simulink model "Dyn_Nonlinear_four"  (R2021a)
settings: Solver=VariableStepAuto  StartTime=0.0  StopTime=10  FixedStep=0.048  MaxStep=0.048  RelTol=1e-5
(part 2 of 7)

== matlab function Dyn_Nonlinear_four/MATLAB Function1 ==
  data: a_teta input; tau output; t input; td input
function tau  = fcn(a_teta, t, td)
theta1 = t(1); theta2 = t(2); theta3 = t(3); 
theta4 = t(4); theta5 = t(5);  

thetad1 = td(1); thetad2 = td(2); thetad3 = td(3);
thetad4 = td(4); thetad5 = td(5); 

M=zeros(5);
M(1,1) = 0.1666*cos(theta4) - 0.4018*sin(theta4) + 0.028*cos(theta4)*cos(theta5) - 1.12*cos(theta1)*sin(theta1) + 0.095452*cos(theta2)*sin(theta2) + 0.367108*cos(theta3)*sin(theta3) - 0.103292*cos(theta4)*sin(theta4) - 0.14*cos(theta4)*sin(theta5) + 0.028*cos(theta5)*sin(theta5) - 3.54*cos(theta1)^2 + 0.30418*cos(theta2)^2 - 0.217828*cos(theta3)^2 - 0.030156*cos(theta4)^2 + 0.0672*cos(theta5)^2 + 0.87*cos(theta2)^2*cos(theta3) - 0.1666*cos(theta2)^2*cos(theta4) - 0.1666*cos(theta3)^2*cos(theta4) - 0.3136*cos(theta2)^2*sin(theta3) + 0.4018*cos(theta2)^2*sin(theta4) + 0.4018*cos(theta3)^2*sin(theta4) + 0.435656*cos(theta2)^2*cos(theta3)^2 + 0.060312*cos(theta2)^2*cos(theta4)^2 - 0.0672*cos(theta2)^2*cos(theta5)^2 + 0.060312*cos(theta3)^2*cos(theta4)^2 - 0.0672*cos(theta3)^2*cos(theta5)^2 - 0.0672*cos(theta4)^2*cos(theta5)^2 - 0.120624*cos(theta2)^2*cos(theta3)^2*cos(theta4)^2 + 0.1344*cos(theta2)^2*cos(theta3)^2*cos(theta5)^2 + 0.1344*cos(theta2)^2*cos(theta4)^2*cos(theta5)^2 + 0.1344*cos(theta3)^2*cos(theta4)^2*cos(theta5)^2 - 0.87*cos(theta2)*sin(theta2)*sin(theta3) + 0.1666*cos(theta2)*sin(theta2)*sin(theta4) + 0.098*cos(theta2)*sin(theta2)*sin(theta5) + 0.1666*cos(theta3)*sin(theta3)*sin(theta4) + 0.098*cos(theta3)*sin(theta3)*sin(theta5) + 0.098*cos(theta4)*sin(theta4)*sin(theta5) + 0.1666*cos(theta2)^2*cos(theta3)*cos(theta4) - 0.028*cos(theta2)^2*cos(theta4)*cos(theta5) - 0.028*cos(theta3)^2*cos(theta4)*cos(theta5) - 0.734216*cos(theta2)*cos(theta3)^2*sin(theta2) + 0.206584*cos(theta2)*cos(theta4)^2*sin(theta2) - 0.734216*cos(theta2)^2*cos(theta3)*sin(theta3) - 0.4018*cos(theta2)^2*cos(theta3)*sin(theta4) - 0.4018*cos(theta2)^2*cos(theta4)*sin(theta3) + 0.206584*cos(theta3)*cos(theta4)^2*sin(theta3) + 0.206584*cos(theta2)^2*cos(theta4)*sin(theta4) + 0.14*cos(theta2)^2*cos(theta4)*sin(theta5) + 0.206584*cos(theta3)^2*cos(theta4)*sin(theta4) - 0.028*cos(theta2)^2*cos(theta5)*sin(theta5) + 0.14*cos(theta3)^2*cos(theta4)*sin(theta5) - 0.028*cos(theta3)^2*cos(theta5)*sin(theta5) - 0.028*cos(theta4)^2*cos(theta5)*sin(theta5) - 0.1666*cos(theta2)^2*sin(theta3)*sin(theta4) + 0.3332*cos(theta2)^2*cos(theta3)^2*cos(theta4) - 0.8036*cos(theta2)^2*cos(theta3)^2*sin(theta4) - 0.3136*cos(theta2)*cos(theta3)*sin(theta2) + 0.4018*cos(theta2)*cos(theta4)*sin(theta2) - 0.0196*cos(theta2)*cos(theta5)*sin(theta2) + 0.4018*cos(theta3)*cos(theta4)*sin(theta3) - 0.0196*cos(theta3)*cos(theta5)*sin(theta3) - 0.0196*cos(theta4)*cos(theta5)*sin(theta4) + 0.028*cos(theta2)^2*cos(theta3)*cos(theta4)*cos(theta5) - 0.8036*cos(theta2)*cos(theta3)^2*cos(theta4)*sin(theta2) + 0.0392*cos(theta2)*cos(theta3)^2*cos(theta5)*sin(theta2) - 0.8036*cos(theta2)^2*cos(theta3)*cos(theta4)*sin(theta3) + 0.0392*cos(theta2)*cos(theta4)^2*cos(theta5)*sin(theta2) + 0.0392*cos(theta2)^2*cos(theta3)*cos(theta5)*sin(theta3) - 0.14*cos(theta2)^2*cos(theta3)*cos(theta4)*sin(theta5) + 0.0392*cos(theta3)*cos(theta4)^2*cos(theta5)*sin(theta3) + 0.0392*cos(theta2)^2*cos(theta4)*cos(theta5)*sin(theta4) + 0.0392*cos(theta3)^2*cos(theta4)*cos(theta5)*sin(theta4) - 0.2688*cos(theta2)^2*cos(theta3)^2*cos(theta4)^2*cos(theta5)^2 - 0.3332*cos(theta2)*cos(theta3)^2*sin(theta2)*sin(theta4) - 0.196*cos(theta2)*cos(theta3)^2*sin(theta2)*sin(theta5) - 0.3332*cos(theta2)^2*cos(theta3)*sin(theta3)*sin(theta4) - 0.196*cos(theta2)*cos(theta4)^2*sin(theta2)*sin(theta5) - 0.196*cos(theta2)^2*cos(theta3)*sin(theta3)*sin(theta5) - 0.028*cos(theta2)^2*cos(theta5)*sin(theta3)*sin(theta4) - 0.196*cos(theta3)*cos(theta4)^2*sin(theta3)*sin(theta5) - 0.196*cos(theta2)^2*cos(theta4)*sin(theta4)*sin(theta5) - 0.196*cos(theta3)^2*cos(theta4)*sin(theta4)*sin(theta5) + 0.14*cos(theta2)^2*sin(theta3)*sin(theta4)*sin(theta5) + 0.056*cos(theta2)^2*cos(theta3)^2*cos(theta4)*cos(theta5) - 0.413168*cos(theta2)*cos(theta3)^2*cos(theta4)^2*sin(theta2) - 0.413168*cos(theta2)^2*cos(theta3)*cos(theta4)^2*sin(theta3) - 0.413168*cos(theta2)^2*cos(theta3)^2*cos(theta4)*sin(theta4) - 0.28*cos(theta2)^2*cos(theta3)^2*cos(theta4)*sin(theta5) + 0.056*cos(theta2)^2*cos(theta3)^2*cos(theta5)*sin(theta5) + 0.056*cos(theta2)^2*cos(theta4)^2*cos(theta5)*sin(theta5) + 0.056*cos(theta3)^2*cos(theta4)^2*cos(theta5)*sin(theta5) - 0.4018*cos(theta2)*cos(theta3)*cos(theta4)*sin(theta2) - 0.435656*cos(theta2)*cos(theta3)*sin(theta2)*sin(theta3) - 0.1666*cos(theta2)*cos(theta3)*sin(theta2)*sin(theta4) - 0.1666*cos(theta2)*cos(theta4)*sin(theta2)*sin(theta3) - 0.060312*cos(theta2)*cos(theta4)*sin(theta2)*sin(theta4) + 0.028*cos(theta2)*cos(theta5)*sin(theta2)*sin(theta4) - 0.060312*cos(theta3)*cos(theta4)*sin(theta3)*sin(theta4) + 0.028*cos(theta3)*cos(theta5)*sin(theta3)*sin(theta4) + 0.4018*cos(theta2)*sin(theta2)*sin(theta3)*sin(theta4) - 0.14*cos(theta2)*sin(theta2)*sin(theta4)*sin(theta5) - 0.14*cos(theta3)*sin(theta3)*sin(theta4)*sin(theta5) + 0.120624*cos(theta2)*cos(theta3)*cos(theta4)^2*sin(theta2)*sin(theta3) - 0.1344*cos(theta2)*cos(theta3)*cos(theta5)^2*sin(theta2)*sin(theta3) + 0.120624*cos(theta2)*cos(theta3)^2*cos(theta4)*sin(theta2)*sin(theta4) - 0.056*cos(theta2)*cos(theta3)^2*cos(theta5)*sin(theta2)*sin(theta4) + 0.120624*cos(theta2)^2*cos(theta3)*cos(theta4)*sin(theta3)*sin(theta4) - 0.1344*cos(theta2)*cos(theta4)*cos(theta5)^2*sin(theta2)*sin(theta4) - 0.056*cos(theta2)^2*cos(theta3)*cos(theta5)*sin(theta3)*sin(theta4) - 0.1344*cos(theta3)*cos(theta4)*cos(theta5)^2*sin(theta3)*sin(theta4) + 0.28*cos(theta2)*cos(theta3)^2*sin(theta2)*sin(theta4)*sin(theta5) + 0.28*cos(theta2)^2*cos(theta3)*sin(theta3)*sin(theta4)*sin(theta5) - 0.0784*cos(theta2)*cos(theta3)^2*cos(theta4)^2*cos(theta5)*sin(theta2) - 0.0784*cos(theta2)^2*cos(theta3)*cos(theta4)^2*cos(theta5)*sin(theta3) - 0.0784*cos(theta2)^2*cos(theta3)^2*cos(theta4)*cos(theta5)*sin(theta4) + 0.392*cos(theta2)*cos(theta3)^2*cos(theta4)^2*sin(theta2)*sin(theta5) + 0.392*cos(theta2)^2*cos(theta3)*cos(theta4)^2*sin(theta3)*sin(theta5) + 0.392*cos(theta2)^2*cos(theta3)^2*cos(theta4)*sin(theta4)*sin(theta5) - 0.3332*cos(theta2)*cos(theta3)*cos(theta4)*sin(theta2)*sin(theta3) - 0.028*cos(theta2)*cos(theta3)*cos(theta5)*sin(theta2)*sin(theta4) - 0.028*cos(theta2)*cos(theta4)*cos(theta5)*sin(theta2)*sin(theta3) - 0.112*cos(theta2)^2*cos(theta3)^2*cos(theta4)^2*cos(theta5)*sin(theta5) + 0.8036*cos(theta2)*cos(theta3)*sin(theta2)*sin(theta3)*sin(theta4) + 0.14*cos(theta2)*cos(theta3)*sin(theta2)*sin(theta4)*sin(theta5) + 0.14*cos(theta2)*cos(theta4)*sin(theta2)*sin(theta3)*sin(theta5) + 0.2688*cos(theta2)*cos(theta3)*cos(theta4)^2*cos(theta5)^2*sin(theta2)*sin(theta3) + 0.2688*cos(theta2)*cos(theta3)^2*cos(theta4)*cos(theta5)^2*sin(theta2)*sin(theta4) + 0.2688*cos(theta2)^2*cos(theta3)*cos(theta4)*cos(theta5)^2*sin(theta3)*sin(theta4) - 0.056*cos(theta2)*cos(theta3)*cos(theta4)*cos(theta5)*sin(theta2)*sin(theta3) + 0.413168*cos(theta2)*cos(theta3)*cos(theta4)*sin(theta2)*sin(theta3)*sin(theta4) + 0.28*cos(theta2)*cos(theta3)*cos(theta4)*sin(theta2)*sin(theta3)*sin(theta5) - 0.056*cos(theta2)*cos(theta3)*cos(theta5)*sin(theta2)*sin(theta3)*sin(theta5) - 0.056*cos(theta2)*cos(theta4)*cos(theta5)*sin(theta2)*sin(theta4)*sin(theta5) - 0.056*cos(theta3)*cos(theta4)*cos(theta5)*sin(theta3)*sin(theta4)*sin(theta5) + 0.0784*cos(theta2)*cos(theta3)*cos(theta4)*cos(theta5)*sin(theta2)*sin(theta3)*sin(theta4) - 0.392*cos(theta2)*cos(theta3)*cos(theta4)*sin(theta2)*sin(theta3)*sin(theta4)*sin(theta5) + 0.112*cos(theta2)*cos(theta3)*cos(theta4)^2*cos(theta5)*sin(theta2)*sin(theta3)*sin(theta5) + 0.112*cos(theta2)*cos(theta3)^2*cos(theta4)*cos(theta5)*sin(theta2)*sin(theta4)*sin(theta5) + 0.112*cos(theta2)^2*cos(theta3)*cos(theta4)*cos(theta5)*sin(theta3)*sin(theta4)*sin(theta5) + 6.759168 ;
M(1,2) = 0.441816*sin(theta2) - 0.053508*cos(theta2) - 0.150528*cos(theta2)*cos(theta3) - 1.1*cos(theta1)*sin(theta1) + 0.4875*cos(theta2)*sin(theta3) + 0.4875*cos(theta3)*sin(theta2) + 0.07*cos(theta5)*sin(theta2) + 0.150528*sin(theta2)*sin(theta3) + 0.014*sin(theta2)*sin(theta5) - 3.54*cos(theta1)^2 - 0.373674*cos(theta2)*sin(theta3)*sin(theta4) - 0.373674*cos(theta3)*sin(theta2)*sin(theta4) - 0.373674*cos(theta4)*sin(theta2)*sin(theta3) + 0.014*cos(theta2)*sin(theta3)*sin(theta5) + 0.014*cos(theta3)*sin(theta2)*sin(theta5) - 0.190918*sin(theta2)*sin(theta3)*sin(theta4) + 0.373674*cos(theta2)*cos(theta3)*cos(theta4) + 0.190918*cos(theta2)*cos(theta3)*sin(theta4) + 0.190918*cos(theta2)*cos(theta4)*sin(theta3) + 0.190918*cos(theta3)*cos(theta4)*sin(theta2) + 0.07*cos(theta2)*cos(theta5)*sin(theta3) + 0.07*cos(theta3)*cos(theta5)*sin(theta2) + 0.028*cos(theta2)*cos(theta3)*cos(theta5)^2*sin(theta4) + 0.028*cos(theta2)*cos(theta4)*cos(theta5)^2*sin(theta3) + 0.028*cos(theta3)*cos(theta4)*cos(theta5)^2*sin(theta2) - 0.028*cos(theta5)^2*sin(theta2)*sin(theta3)*sin(theta4) + 0.049*cos(theta2)*cos(theta3)*cos(theta4)*cos(theta5) + 0.0098*cos(theta2)*cos(theta3)*cos(theta4)*sin(theta5) - 0.049*cos(theta2)*cos(theta5)*sin(theta3)*sin(theta4) - 0.049*cos(theta3)*cos(theta5)*sin(theta2)*sin(theta4) - 0.049*cos(theta4)*cos(theta5)*sin(theta2)*sin(theta3) - 0.0098*cos(theta2)*sin(theta3)*sin(theta4)*sin(theta5) - 0.0098*cos(theta3)*sin(theta2)*sin(theta4)*sin(theta5) - 0.0098*cos(theta4)*sin(theta2)*sin(theta3)*sin(theta5) - 0.0672*cos(theta2)*cos(theta3)*cos(theta5)*sin(theta4)*sin(theta5) - 0.0672*cos(theta2)*cos(theta4)*cos(theta5)*sin(theta3)*sin(theta5) - 0.0672*cos(theta3)*cos(theta4)*cos(theta5)*sin(theta2)*sin(theta5) + 0.0672*cos(theta5)*sin(theta2)*sin(theta3)*sin(theta4)*sin(theta5) + 4.14 ;
M(1,3) = 0.4875*cos(theta2)*sin(theta3) - 1.04*cos(theta1)*sin(theta1) - 0.150528*cos(theta2)*cos(theta3) + 0.4875*cos(theta3)*sin(theta2) + 0.150528*sin(theta2)*sin(theta3) - 3.43*cos(theta1)^2 - 0.373674*cos(theta2)*sin(theta3)*sin(theta4) - 0.373674*cos(theta3)*sin(theta2)*sin(theta4) - 0.373674*cos(theta4)*sin(theta2)*sin(theta3) + 0.014*cos(theta2)*sin(theta3)*sin(theta5) + 0.014*cos(theta3)*sin(theta2)*sin(theta5) - 0.190918*sin(theta2)*sin(theta3)*sin(theta4) + 0.373674*cos(theta2)*cos(theta3)*cos(theta4) + 0.190918*cos(theta2)*cos(theta3)*sin(theta4) + 0.190918*cos(theta2)*cos(theta4)*sin(theta3) + 0.190918*cos(theta3)*cos(theta4)*sin(theta2) + 0.07*cos(theta2)*cos(theta5)*sin(theta3) + 0.07*cos(theta3)*cos(theta5)*sin(theta2) + 0.028*cos(theta2)*cos(theta3)*cos(theta5)^2*sin(theta4) + 0.028*cos(theta2)*cos(theta4)*cos(theta5)^2*sin(theta3) + 0.028*cos(theta3)*cos(theta4)*cos(theta5)^2*sin(theta2) - 0.028*cos(theta5)^2*sin(theta2)*sin(theta3)*sin(theta4) + 0.049*cos(theta2)*cos(theta3)*cos(theta4)*cos(theta5) + 0.0098*cos(theta2)*cos(theta3)*cos(theta4)*sin(theta5) - 0.049*cos(theta2)*cos(theta5)*sin(theta3)*sin(theta4) - 0.049*cos(theta3)*cos(theta5)*sin(theta2)*sin(theta4) - 0.049*cos(theta4)*cos(theta5)*sin(theta2)*sin(theta3) - 0.0098*cos(theta2)*sin(theta3)*sin(theta4)*sin(theta5) - 0.0098*cos(theta3)*sin(theta2)*sin(theta4)*sin(theta5) - 0.0098*cos(theta4)*sin(theta2)*sin(theta3)*sin(theta5) - 0.0672*cos(theta2)*cos(theta3)*cos(theta5)*sin(theta4)*sin(theta5) - 0.0672*cos(theta2)*cos(theta4)*cos(theta5)*sin(theta3)*sin(theta5) - 0.0672*cos(theta3)*cos(theta4)*cos(theta5)*sin(theta2)*sin(theta5) + 0.0672*cos(theta5)*sin(theta2)*sin(theta3)*sin(theta4)*sin(theta5) + 3.98 ;
M(1,4) = 0.249082*sin(theta2)*sin(theta3)*sin(theta4) - 0.373674*cos(theta3)*sin(theta2)*sin(theta4) - 0.373674*cos(theta4)*sin(theta2)*sin(theta3) - 0.373674*cos(theta2)*sin(theta3)*sin(theta4) + 0.373674*cos(theta2)*cos(theta3)*cos(theta4) - 0.249082*cos(theta2)*cos(theta3)*sin(theta4) - 0.249082*cos(theta2)*cos(theta4)*sin(theta3) - 0.249082*cos(theta3)*cos(theta4)*sin(theta2) + 0.88*cos(theta1)^2*cos(theta2)*cos(theta3)*sin(theta4) + 0.88*cos(theta1)^2*cos(theta2)*cos(theta4)*sin(theta3) + 0.88*cos(theta1)^2*cos(theta3)*cos(theta4)*sin(theta2) + 0.028*cos(theta2)*cos(theta3)*cos(theta5)^2*sin(theta4) + 0.028*cos(theta2)*cos(theta4)*cos(theta5)^2*sin(theta3) + 0.028*cos(theta3)*cos(theta4)*cos(theta5)^2*sin(theta2) - 0.88*cos(theta1)^2*sin(theta2)*sin(theta3)*sin(theta4) - 0.028*cos(theta5)^2*sin(theta2)*sin(theta3)*sin(theta4) - 0.7*cos(theta1)*cos(theta2)*cos(theta3)*cos(theta4) + 0.049*cos(theta2)*cos(theta3)*cos(theta4)*cos(theta5) + 0.1*cos(theta2)*cos(theta3)*cos(theta4)*sin(theta1) + 0.0098*cos(theta2)*cos(theta3)*cos(theta4)*sin(theta5) + 0.7*cos(theta1)*cos(theta2)*sin(theta3)*sin(theta4) + 0.7*cos(theta1)*cos(theta3)*sin(theta2)*sin(theta4) + 0.7*cos(theta1)*cos(theta4)*sin(theta2)*sin(theta3) - 0.049*cos(theta2)*cos(theta5)*sin(theta3)*sin(theta4) - 0.049*cos(theta3)*cos(theta5)*sin(theta2)*sin(theta4) - 0.049*cos(theta4)*cos(theta5)*sin(theta2)*sin(theta3) - 0.1*cos(theta2)*sin(theta1)*sin(theta3)*sin(theta4) - 0.1*cos(theta3)*sin(theta1)*sin(theta2)*sin(theta4) - 0.1*cos(theta4)*sin(theta1)*sin(theta2)*sin(theta3) - 0.0098*cos(theta2)*sin(theta3)*sin(theta4)*sin(theta5) - 0.0098*cos(theta3)*sin(theta2)*sin(theta4)*sin(theta5) - 0.0098*cos(theta4)*sin(theta2)*sin(theta3)*sin(theta5) - 3.14*cos(theta1)*cos(theta2)*cos(theta3)*sin(theta1)*sin(theta4) - 3.14*cos(theta1)*cos(theta2)*cos(theta4)*sin(theta1)*sin(theta3) - 3.14*cos(theta1)*cos(theta3)*cos(theta4)*sin(theta1)*sin(theta2) - 0.0672*cos(theta2)*cos(theta3)*cos(theta5)*sin(theta4)*sin(theta5) - 0.0672*cos(theta2)*cos(theta4)*cos(theta5)*sin(theta3)*sin(theta5) - 0.0672*cos(theta3)*cos(theta4)*cos(theta5)*sin(theta2)*sin(theta5) + 3.14*cos(theta1)*sin(theta1)*sin(theta2)*sin(theta3)*sin(theta4) + 0.0672*cos(theta5)*sin(theta2)*sin(theta3)*sin(theta4)*sin(theta5) ;
M(1,5) = 0.014*cos(theta2)*cos(theta5) - 0.07*cos(theta2)*sin(theta5) - 0.0728*cos(theta2)*sin(theta3)*sin(theta4) - 0.0728*cos(theta3)*sin(theta2)*sin(theta4) - 0.0728*cos(theta4)*sin(theta2)*sin(theta3) - 0.014*cos(theta5)*sin(theta2)*sin(theta3) + 0.22*sin(theta2)*sin(theta3)*sin(theta4) + 0.07*sin(theta2)*sin(theta3)*sin(theta5) + 0.0728*cos(theta2)*cos(theta3)*cos(theta4) + 0.014*cos(theta2)*cos(theta3)*cos(theta5) - 0.22*cos(theta2)*cos(theta3)*sin(theta4) - 0.22*cos(theta2)*cos(theta4)*sin(theta3) - 0.22*cos(theta3)*cos(theta4)*sin(theta2) - 0.07*cos(theta2)*cos(theta3)*sin(theta5) + 0.44*cos(theta1)^2*cos(theta2)*cos(theta3)*sin(theta4) + 0.44*cos(theta1)^2*cos(theta2)*cos(theta4)*sin(theta3) + 0.44*cos(theta1)^2*cos(theta3)*cos(theta4)*sin(theta2) - 0.44*cos(theta1)^2*sin(theta2)*sin(theta3)*sin(theta4) - 0.35*cos(theta1)*cos(theta2)*cos(theta3)*cos(theta4) + 0.05*cos(theta2)*cos(theta3)*cos(theta4)*sin(theta1) - 0.0098*cos(theta2)*cos(theta3)*cos(theta5)*sin(theta4) - 0.0098*cos(theta2)*cos(theta4)*cos(theta5)*sin(theta3) - 0.0098*cos(theta3)*cos(theta4)*cos(theta5)*sin(theta2) + 0.35*cos(theta1)*cos(theta2)*sin(theta3)*sin(theta4) + 0.35*cos(theta1)*cos(theta3)*sin(theta2)*sin(theta4) + 0.35*cos(theta1)*cos(theta4)*sin(theta2)*sin(theta3) + 0.049*cos(theta2)*cos(theta3)*sin(theta4)*sin(theta5) + 0.049*cos(theta2)*cos(theta4)*sin(theta3)*sin(theta5) + 0.049*cos(theta3)*cos(theta4)*sin(theta2)*sin(theta5) - 0.05*cos(theta2)*sin(theta1)*sin(theta3)*sin(theta4) - 0.05*cos(theta3)*sin(theta1)*sin(theta2)*sin(theta4) - 0.05*cos(theta4)*sin(theta1)*sin(theta2)*sin(theta3) + 0.0098*cos(theta5)*sin(theta2)*sin(theta3)*sin(theta4) - 0.049*sin(theta2)*sin(theta3)*sin(theta4)*sin(theta5) - 1.57*cos(theta1)*cos(theta2)*cos(theta3)*sin(theta1)*sin(theta4) - 1.57*cos(theta1)*cos(theta2)*cos(theta4)*sin(theta1)*sin(theta3) - 1.57*cos(theta1)*cos(theta3)*cos(theta4)*sin(theta1)*sin(theta2) + 1.57*cos(theta1)*sin(theta1)*sin(theta2)*sin(theta3)*sin(theta4) ;
M(2,1) = 0.441816*sin(theta2) - 0.053508*cos(theta2) - 0.150528*cos(theta2)*cos(theta3) - 1.1*cos(theta1)*sin(theta1) + 0.4875*cos(theta2)*sin(theta3) + 0.4875*cos(theta3)*sin(theta2) + 0.07*cos(theta5)*sin(theta2) + 0.150528*sin(theta2)*sin(theta3) + 0.014*sin(theta2)*sin(theta5) - 3.54*cos(theta1)^2 - 0.373674*cos(theta2)*sin(theta3)*sin(theta4) - 0.373674*cos(theta3)*sin(theta2)*sin(theta4) - 0.373674*cos(theta4)*sin(theta2)*sin(theta3) + 0.014*cos(theta2)*sin(theta3)*sin(theta5) + 0.014*cos(theta3)*sin(theta2)*sin(theta5) - 0.190918*sin(theta2)*sin(theta3)*sin(theta4) + 0.373674*cos(theta2)*cos(theta3)*cos(theta4) + 0.190918*cos(theta2)*cos(theta3)*sin(theta4) + 0.190918*cos(theta2)*cos(theta4)*sin(theta3) + 0.190918*cos(theta3)*cos(theta4)*sin(theta2) + 0.07*cos(theta2)*cos(theta5)*sin(theta3) + 0.07*cos(theta3)*cos(theta5)*sin(theta2) + 0.028*cos(theta2)*cos(theta3)*cos(theta5)^2*sin(theta4) + 0.028*cos(theta2)*cos(theta4)*cos(theta5)^2*sin(theta3) + 0.028*cos(theta3)*cos(theta4)*cos(theta5)^2*sin(theta2) - 0.028*cos(theta5)^2*sin(theta2)*sin(theta3)*sin(theta4) + 0.049*cos(theta2)*cos(theta3)*cos(theta4)*cos(theta5) + 0.0098*cos(theta2)*cos(theta3)*cos(theta4)*sin(theta5) - 0.049*cos(theta2)*cos(theta5)*sin(theta3)*sin(theta4) - 0.049*cos(theta3)*cos(theta5)*sin(theta2)*sin(theta4) - 0.049*cos(theta4)*cos(theta5)*sin(theta2)*sin(theta3) - 0.0098*cos(theta2)*sin(theta3)*sin(theta4)*sin(theta5) - 0.0098*cos(theta3)*sin(theta2)*sin(theta4)*sin(theta5) - 0.0098*cos(theta4)*sin(theta2)*sin(theta3)*sin(theta5) - 0.0672*cos(theta2)*cos(theta3)*cos(theta5)*sin(theta4)*sin(theta5) - 0.0672*cos(theta2)*cos(theta4)*cos(theta5)*sin(theta3)*sin(theta5) - 0.0672*cos(theta3)*cos(theta4)*cos(theta5)*sin(theta2)*sin(theta5) + 0.0672*cos(theta5)*sin(theta2)*sin(theta3)*sin(theta4)*sin(theta5) + 4.14 ;
M(2,2) = 0.87*cos(theta3) + 0.1666*cos(theta4) - 0.3136*sin(theta3) - 0.4018*sin(theta4) + 0.1666*cos(theta3)*cos(theta4) + 0.028*cos(theta4)*cos(theta5) - 1.1*cos(theta1)*sin(theta1) - 0.4018*cos(theta3)*sin(theta4) - 0.4018*cos(theta4)*sin(theta3) - 0.14*cos(theta4)*sin(theta5) - 0.028*cos(theta5)*sin(theta5) - 0.1666*sin(theta3)*sin(theta4) - 3.54*cos(theta1)^2 - 0.0672*cos(theta5)^2 - 0.028*cos(theta5)*sin(theta3)*sin(theta4) + 0.14*sin(theta3)*sin(theta4)*sin(theta5) + 0.028*cos(theta3)*cos(theta4)*cos(theta5) - 0.14*cos(theta3)*cos(theta4)*sin(theta5) + 5.864008 ;
M(2,3) = 0.435*cos(theta3) + 0.1666*cos(theta4) - 0.1568*sin(theta3) - 0.4018*sin(theta4) + 0.0833*cos(theta3)*cos(theta4) + 0.028*cos(theta4)*cos(theta5) - 1.04*cos(theta1)*sin(theta1) - 0.2009*cos(theta3)*sin(theta4) - 0.2009*cos(theta4)*sin(theta3) - 0.14*cos(theta4)*sin(theta5) - 0.028*cos(theta5)*sin(theta5) - 0.0833*sin(theta3)*sin(theta4) - 3.43*cos(theta1)^2 - 0.0672*cos(theta5)^2 - 0.014*cos(theta5)*sin(theta3)*sin(theta4) + 0.07*sin(theta3)*sin(theta4)*sin(theta5) + 0.014*cos(theta3)*cos(theta4)*cos(theta5) - 0.07*cos(theta3)*cos(theta4)*sin(theta5) + 5.009128 ;
M(2,4) = 0.0833*cos(theta4) - 0.2009*sin(theta4) + 0.0833*cos(theta3)*cos(theta4) + 0.014*cos(theta4)*cos(theta5) - 0.2009*cos(theta3)*sin(theta4) - 0.2009*cos(theta4)*sin(theta3) - 0.07*cos(theta4)*sin(theta5) - 0.028*cos(theta5)*sin(theta5) - 0.0833*sin(theta3)*sin(theta4) - 0.0672*cos(theta5)^2 - 0.014*cos(theta5)*sin(theta3)*sin(theta4) + 0.44*sin(theta2)*sin(theta3)*sin(theta4) + 0.07*sin(theta3)*sin(theta4)*sin(theta5) + 0.014*cos(theta3)*cos(theta4)*cos(theta5) - 0.44*cos(theta2)*cos(theta3)*sin(theta4) - 0.44*cos(theta2)*cos(theta4)*sin(theta3) - 0.44*cos(theta3)*cos(theta4)*sin(theta2) - 0.07*cos(theta3)*cos(theta4)*sin(theta5) + 0.88*cos(theta1)^2*cos(theta2)*cos(theta3)*sin(theta4) + 0.88*cos(theta1)^2*cos(theta2)*cos(theta4)*sin(theta3) + 0.88*cos(theta1)^2*cos(theta3)*cos(theta4)*sin(theta2) - 0.88*cos(theta1)^2*sin(theta2)*sin(theta3)*sin(theta4) - 0.7*cos(theta1)*cos(theta2)*cos(theta3)*cos(theta4) + 0.1*cos(theta2)*cos(theta3)*cos(theta4)*sin(theta1) + 0.7*cos(theta1)*cos(theta2)*sin(theta3)*sin(theta4) + 0.7*cos(theta1)*cos(theta3)*sin(theta2)*sin(theta4) + 0.7*cos(theta1)*cos(theta4)*sin(theta2)*sin(theta3) - 0.1*cos(theta2)*sin(theta1)*sin(theta3)*sin(theta4) - 0.1*cos(theta3)*sin(theta1)*sin(theta2)*sin(theta4) - 0.1*cos(theta4)*sin(theta1)*sin(theta2)*sin(theta3) - 3.14*cos(theta1)*cos(theta2)*cos(theta3)*sin(theta1)*sin(theta4) - 3.14*cos(theta1)*cos(theta2)*cos(theta4)*sin(theta1)*sin(theta3) - 3.14*cos(theta1)*cos(theta3)*cos(theta4)*sin(theta1)*sin(theta2) + 3.14*cos(theta1)*sin(theta1)*sin(theta2)*sin(theta3)*sin(theta4) + 0.2268 ;
M(2,5) = 0.049*cos(theta5) + 0.0098*sin(theta5) - 0.07*cos(theta5)*sin(theta4) - 0.014*sin(theta4)*sin(theta5) - 0.014*cos(theta3)*sin(theta4)*sin(theta5) - 0.014*cos(theta4)*sin(theta3)*sin(theta5) + 0.22*sin(theta2)*sin(theta3)*sin(theta4) - 0.22*cos(theta2)*cos(theta3)*sin(theta4) - 0.22*cos(theta2)*cos(theta4)*sin(theta3) - 0.22*cos(theta3)*cos(theta4)*sin(theta2) - 0.07*cos(theta3)*cos(theta5)*sin(theta4) - 0.07*cos(theta4)*cos(theta5)*sin(theta3) + 0.44*cos(theta1)^2*cos(theta2)*cos(theta3)*sin(theta4) + 0.44*cos(theta1)^2*cos(theta2)*cos(theta4)*sin(theta3) + 0.44*cos(theta1)^2*cos(theta3)*cos(theta4)*sin(theta2) - 0.44*cos(theta1)^2*sin(theta2)*sin(theta3)*sin(theta4) - 0.35*cos(theta1)*cos(theta2)*cos(theta3)*cos(theta4) + 0.05*cos(theta2)*cos(theta3)*cos(theta4)*sin(theta1) + 0.35*cos(theta1)*cos(theta2)*sin(theta3)*sin(theta4) + 0.35*cos(theta1)*cos(theta3)*sin(theta2)*sin(theta4) + 0.35*cos(theta1)*cos(theta4)*sin(theta2)*sin(theta3) - 0.05*cos(theta2)*sin(theta1)*sin(theta3)*sin(theta4) - 0.05*cos(theta3)*sin(theta1)*sin(theta2)*sin(theta4) - 0.05*cos(theta4)*sin(theta1)*sin(theta2)*sin(theta3) - 1.57*cos(theta1)*cos(theta2)*cos(theta3)*sin(theta1)*sin(theta4) - 1.57*cos(theta1)*cos(theta2)*cos(theta4)*sin(theta1)*sin(theta3) - 1.57*cos(theta1)*cos(theta3)*cos(theta4)*sin(theta1)*sin(theta2) + 1.57*cos(theta1)*sin(theta1)*sin(theta2)*sin(theta3)*sin(theta4) ;
M(3,1) = 0.4875*cos(theta2)*sin(theta3) - 1.04*cos(theta1)*sin(theta1) - 0.150528*cos(theta2)*cos(theta3) + 0.4875*cos(theta3)*sin(theta2) + 0.150528*sin(theta2)*sin(theta3) - 3.43*cos(theta1)^2 - 0.373674*cos(theta2)*sin(theta3)*sin(theta4) - 0.373674*cos(theta3)*sin(theta2)*sin(theta4) - 0.373674*cos(theta4)*sin(theta2)*sin(theta3) + 0.014*cos(theta2)*sin(theta3)*sin(theta5) + 0.014*cos(theta3)*sin(theta2)*sin(theta5) - 0.190918*sin(theta2)*sin(theta3)*sin(theta4) + 0.373674*cos(theta2)*cos(theta3)*cos(theta4) + 0.190918*cos(theta2)*cos(theta3)*sin(theta4) + 0.190918*cos(theta2)*cos(theta4)*sin(theta3) + 0.190918*cos(theta3)*cos(theta4)*sin(theta2) + 0.07*cos(theta2)*cos(theta5)*sin(theta3) + 0.07*cos(theta3)*cos(theta5)*sin(theta2) + 0.028*cos(theta2)*cos(theta3)*cos(theta5)^2*sin(theta4) + 0.028*cos(theta2)*cos(theta4)*cos(theta5)^2*sin(theta3) + 0.028*cos(theta3)*cos(theta4)*cos(theta5)^2*sin(theta2) - 0.028*cos(theta5)^2*sin(theta2)*sin(theta3)*sin(theta4) + 0.049*cos(theta2)*cos(theta3)*cos(theta4)*cos(theta5) + 0.0098*cos(theta2)*cos(theta3)*cos(theta4)*sin(theta5) - 0.049*cos(theta2)*cos(theta5)*sin(theta3)*sin(theta4) - 0.049*cos(theta3)*cos(theta5)*sin(theta2)*sin(theta4) - 0.049*cos(theta4)*cos(theta5)*sin(theta2)*sin(theta3) - 0.0098*cos(theta2)*sin(theta3)*sin(theta4)*sin(theta5) - 0.0098*cos(theta3)*sin(theta2)*sin(theta4)*sin(theta5) - 0.0098*cos(theta4)*sin(theta2)*sin(theta3)*sin(theta5) - 0.0672*cos(theta2)*cos(theta3)*cos(theta5)*sin(theta4)*sin(theta5) - 0.0672*cos(theta2)*cos(theta4)*cos(theta5)*sin(theta3)*sin(theta5) - 0.0672*cos(theta3)*cos(theta4)*cos(theta5)*sin(theta2)*sin(theta5) + 0.0672*cos(theta5)*sin(theta2)*sin(theta3)*sin(theta4)*sin(theta5) + 3.98 ;
M(3,2) = 0.435*cos(theta3) + 0.1666*cos(theta4) - 0.1568*sin(theta3) - 0.4018*sin(theta4) + 0.0833*cos(theta3)*cos(theta4) + 0.028*cos(theta4)*cos(theta5) - 1.04*cos(theta1)*sin(theta1) - 0.2009*cos(theta3)*sin(theta4) - 0.2009*cos(theta4)*sin(theta3) - 0.14*cos(theta4)*sin(theta5) - 0.028*cos(theta5)*sin(theta5) - 0.0833*sin(theta3)*sin(theta4) - 3.43*cos(theta1)^2 - 0.0672*cos(theta5)^2 - 0.014*cos(theta5)*sin(theta3)*sin(theta4) + 0.07*sin(theta3)*sin(theta4)*sin(theta5) + 0.014*cos(theta3)*cos(theta4)*cos(theta5) - 0.07*cos(theta3)*cos(theta4)*sin(theta5) + 5.009128 ;
M(3,3) = 0.1666*cos(theta4) - 0.4018*sin(theta4) + 0.028*cos(theta4)*cos(theta5) - 1.04*cos(theta1)*sin(theta1) - 0.14*cos(theta4)*sin(theta5) - 0.028*cos(theta5)*sin(theta5) - 3.43*cos(theta1)^2 - 0.0672*cos(theta5)^2 + 5.009128 ;
M(3,4) = 0.0833*cos(theta4) - 0.2009*sin(theta4) + 0.014*cos(theta4)*cos(theta5) - 0.07*cos(theta4)*sin(theta5) - 0.028*cos(theta5)*sin(theta5) - 0.0672*cos(theta5)^2 + 0.44*sin(theta2)*sin(theta3)*sin(theta4) - 0.44*cos(theta2)*cos(theta3)*sin(theta4) - 0.44*cos(theta2)*cos(theta4)*sin(theta3) - 0.44*cos(theta3)*cos(theta4)*sin(theta2) + 0.88*cos(theta1)^2*cos(theta2)*cos(theta3)*sin(theta4) + 0.88*cos(theta1)^2*cos(theta2)*cos(theta4)*sin(theta3) + 0.88*cos(theta1)^2*cos(theta3)*cos(theta4)*sin(theta2) - 0.88*cos(theta1)^2*sin(theta2)*sin(theta3)*sin(theta4) - 0.7*cos(theta1)*cos(theta2)*cos(theta3)*cos(theta4) + 0.1*cos(theta2)*cos(theta3)*cos(theta4)*sin(theta1) + 0.7*cos(theta1)*cos(theta2)*sin(theta3)*sin(theta4) + 0.7*cos(theta1)*cos(theta3)*sin(theta2)*sin(theta4) + 0.7*cos(theta1)*cos(theta4)*sin(theta2)*sin(theta3) - 0.1*cos(theta2)*sin(theta1)*sin(theta3)*sin(theta4) - 0.1*cos(theta3)*sin(theta1)*sin(theta2)*sin(theta4) - 0.1*cos(theta4)*sin(theta1)*sin(theta2)*sin(theta3) - 3.14*cos(theta1)*cos(theta2)*cos(theta3)*sin(theta1)*sin(theta4) - 3.14*cos(theta1)*cos(theta2)*cos(theta4)*sin(theta1)*sin(theta3) - 3.14*cos(theta1)*cos(theta3)*cos(theta4)*sin(theta1)*sin(theta2) + 3.14*cos(theta1)*sin(theta1)*sin(theta2)*sin(theta3)*sin(theta4) + 0.2268 ;
M(3,5) = 0.049*cos(theta5) + 0.0098*sin(theta5) - 0.07*cos(theta5)*sin(theta4) - 0.014*sin(theta4)*sin(theta5) + 0.22*sin(theta2)*sin(theta3)*sin(theta4) - 0.22*cos(theta2)*cos(theta3)*sin(theta4) - 0.22*cos(theta2)*cos(theta4)*sin(theta3) - 0.22*cos(theta3)*cos(theta4)*sin(theta2) + 0.44*cos(theta1)^2*cos(theta2)*cos(theta3)*sin(theta4) + 0.44*cos(theta1)^2*cos(theta2)*cos(theta4)*sin(theta3) + 0.44*cos(theta1)^2*cos(theta3)*cos(theta4)*sin(theta2) - 0.44*cos(theta1)^2*sin(theta2)*sin(theta3)*sin(theta4) - 0.35*cos(theta1)*cos(theta2)*cos(theta3)*cos(theta4) + 0.05*cos(theta2)*cos(theta3)*cos(theta4)*sin(theta1) + 0.35*cos(theta1)*cos(theta2)*sin(theta3)*sin(theta4) + 0.35*cos(theta1)*cos(theta3)*sin(theta2)*sin(theta4) + 0.35*cos(theta1)*cos(theta4)*sin(theta2)*sin(theta3) - 0.05*cos(theta2)*sin(theta1)*sin(theta3)*sin(theta4) - 0.05*cos(theta3)*sin(theta1)*sin(theta2)*sin(theta4) - 0.05*cos(theta4)*sin(theta1)*sin(theta2)*sin(theta3) - 1.57*cos(theta1)*cos(theta2)*cos(theta3)*sin(theta1)*sin(theta4) - 1.57*cos(theta1)*cos(theta2)*cos(theta4)*sin(theta1)*sin(theta3) - 1.57*cos(theta1)*cos(theta3)*cos(theta4)*sin(theta1)*sin(theta2) + 1.57*cos(theta1)*sin(theta1)*sin(theta2)*sin(theta3)*sin(theta4) ;
M(4,1) = 0.249082*sin(theta2)*sin(theta3)*sin(theta4) - 0.373674*cos(theta3)*sin(theta2)*sin(theta4) - 0.373674*cos(theta4)*sin(theta2)*sin(theta3) - 0.373674*cos(theta2)*sin(theta3)*sin(theta4) + 0.373674*cos(theta2)*cos(theta3)*cos(theta4) - 0.249082*cos(theta2)*cos(theta3)*sin(theta4) - 0.249082*cos(theta2)*cos(theta4)*sin(theta3) - 0.249082*cos(theta3)*cos(theta4)*sin(theta2) + 0.88*cos(theta1)^2*cos(theta2)*cos(theta3)*sin(theta4) + 0.88*cos(theta1)^2*cos(theta2)*cos(theta4)*sin(theta3) + 0.88*cos(theta1)^2*cos(theta3)*cos(theta4)*sin(theta2) + 0.028*cos(theta2)*cos(theta3)*cos(theta5)^2*sin(theta4) + 0.028*cos(theta2)*cos(theta4)*cos(theta5)^2*sin(theta3) + 0.028*cos(theta3)*cos(theta4)*cos(theta5)^2*sin(theta2) - 0.88*cos(theta1)^2*sin(theta2)*sin(theta3)*sin(theta4) - 0.028*cos(theta5)^2*sin(theta2)*sin(theta3)*sin(theta4) - 0.7*cos(theta1)*cos(theta2)*cos(theta3)*cos(theta4) + 0.049*cos(theta2)*cos(theta3)*cos(theta4)*cos(theta5) + 0.1*cos(theta2)*cos(theta3)*cos(theta4)*sin(theta1) + 0.0098*cos(theta2)*cos(theta3)*cos(theta4)*sin(theta5) + 0.7*cos(theta1)*cos(theta2)*sin(theta3)*sin(theta4) + 0.7*cos(theta1)*cos(theta3)*sin(theta2)*sin(theta4) + 0.7*cos(theta1)*cos(theta4)*sin(theta2)*sin(theta3) - 0.049*cos(theta2)*cos(theta5)*sin(theta3)*sin(theta4) - 0.049*cos(theta3)*cos(theta5)*sin(theta2)*sin(theta4) - 0.049*cos(theta4)*cos(theta5)*sin(theta2)*sin(theta3) - 0.1*cos(theta2)*sin(theta1)*sin(theta3)*sin(theta4) - 0.1*cos(theta3)*sin(theta1)*sin(theta2)*sin(theta4) - 0.1*cos(theta4)*sin(theta1)*sin(theta2)*sin(theta3) - 0.0098*cos(theta2)*sin(theta3)*sin(theta4)*sin(theta5) - 0.0098*cos(theta3)*sin(theta2)*sin(theta4)*sin(theta5) - 0.0098*cos(theta4)*sin(theta2)*sin(theta3)*sin(theta5) - 3.14*cos(theta1)*cos(theta2)*cos(theta3)*sin(theta1)*sin(theta4) - 3.14*cos(theta1)*cos(theta2)*cos(theta4)*sin(theta1)*sin(theta3) - 3.14*cos(theta1)*cos(theta3)*cos(theta4)*sin(theta1)*sin(theta2) - 0.0672*cos(theta2)*cos(theta3)*cos(theta5)*sin(theta4)*sin(theta5) - 0.0672*cos(theta2)*cos(theta4)*cos(theta5)*sin(theta3)*sin(theta5) - 0.0672*cos(theta3)*cos(theta4)*cos(theta5)*sin(theta2)*sin(theta5) + 3.14*cos(theta1)*sin(theta1)*sin(theta2)*sin(theta3)*sin(theta4) + 0.0672*cos(theta5)*sin(theta2)*sin(theta3)*sin(theta4)*sin(theta5) ;
M(4,2) = 0.0833*cos(theta4) - 0.2009*sin(theta4) + 0.0833*cos(theta3)*cos(theta4) + 0.014*cos(theta4)*cos(theta5) - 0.2009*cos(theta3)*sin(theta4) - 0.2009*cos(theta4)*sin(theta3) - 0.07*cos(theta4)*sin(theta5) - 0.028*cos(theta5)*sin(theta5) - 0.0833*sin(theta3)*sin(theta4) - 0.0672*cos(theta5)^2 - 0.014*cos(theta5)*sin(theta3)*sin(theta4) + 0.44*sin(theta2)*sin(theta3)*sin(theta4) + 0.07*sin(theta3)*sin(theta4)*sin(theta5) + 0.014*cos(theta3)*cos(theta4)*cos(theta5) - 0.44*cos(theta2)*cos(theta3)*sin(theta4) - 0.44*cos(theta2)*cos(theta4)*sin(theta3) - 0.44*cos(theta3)*cos(theta4)*sin(theta2) - 0.07*cos(theta3)*cos(theta4)*sin(theta5) + 0.88*cos(theta1)^2*cos(theta2)*cos(theta3)*sin(theta4) + 0.88*cos(theta1)^2*cos(theta2)*cos(theta4)*sin(theta3) + 0.88*cos(theta1)^2*cos(theta3)*cos(theta4)*sin(theta2) - 0.88*cos(theta1)^2*sin(theta2)*sin(theta3)*sin(theta4) - 0.7*cos(theta1)*cos(theta2)*cos(theta3)*cos(theta4) + 0.1*cos(theta2)*cos(theta3)*cos(theta4)*sin(theta1) + 0.7*cos(theta1)*cos(theta2)*sin(theta3)*sin(theta4) + 0.7*cos(theta1)*cos(theta3)*sin(theta2)*sin(theta4) + 0.7*cos(theta1)*cos(theta4)*sin(theta2)*sin(theta3) - 0.1*cos(theta2)*sin(theta1)*sin(theta3)*sin(theta4) - 0.1*cos(theta3)*sin(theta1)*sin(theta2)*sin(theta4) - 0.1*cos(theta4)*sin(theta1)*sin(theta2)*sin(theta3) - 3.14*cos(theta1)*cos(theta2)*cos(theta3)*sin(theta1)*sin(theta4) - 3.14*cos(theta1)*cos(theta2)*cos(theta4)*sin(theta1)*sin(theta3) - 3.14*cos(theta1)*cos(theta3)*cos(theta4)*sin(theta1)*sin(theta2) + 3.14*cos(theta1)*sin(theta1)*sin(theta2)*sin(theta3)*sin(theta4) + 0.2268 ;
M(4,3) = 0.0833*cos(theta4) - 0.2009*sin(theta4) + 0.014*cos(theta4)*cos(theta5) - 0.07*cos(theta4)*sin(theta5) - 0.028*cos(theta5)*sin(theta5) - 0.0672*cos(theta5)^2 + 0.44*sin(theta2)*sin(theta3)*sin(theta4) - 0.44*cos(theta2)*cos(theta3)*sin(theta4) - 0.44*cos(theta2)*cos(theta4)*sin(theta3) - 0.44*cos(theta3)*cos(theta4)*sin(theta2) + 0.88*cos(theta1)^2*cos(theta2)*cos(theta3)*sin(theta4) + 0.88*cos(theta1)^2*cos(theta2)*cos(theta4)*sin(theta3) + 0.88*cos(theta1)^2*cos(theta3)*cos(theta4)*sin(theta2) - 0.88*cos(theta1)^2*sin(theta2)*sin(theta3)*sin(theta4) - 0.7*cos(theta1)*cos(theta2)*cos(theta3)*cos(theta4) + 0.1*cos(theta2)*cos(theta3)*cos(theta4)*sin(theta1) + 0.7*cos(theta1)*cos(theta2)*sin(theta3)*sin(theta4) + 0.7*cos(theta1)*cos(theta3)*sin(theta2)*sin(theta4) + 0.7*cos(theta1)*cos(theta4)*sin(theta2)*sin(theta3) - 0.1*cos(theta2)*sin(theta1)*sin(theta3)*sin(theta4) - 0.1*cos(theta3)*sin(theta1)*sin(theta2)*sin(theta4) - 0.1*cos(theta4)*sin(theta1)*sin(theta2)*sin(theta3) - 3.14*cos(theta1)*cos(theta2)*cos(theta3)*sin(theta1)*sin(theta4) - 3.14*cos(theta1)*cos(theta2)*cos(theta4)*sin(theta1)*sin(theta3) - 3.14*cos(theta1)*cos(theta3)*cos(theta4)*sin(theta1)*sin(theta2) + 3.14*cos(theta1)*sin(theta1)*sin(theta2)*sin(theta3)*sin(theta4) + 0.2268 ;
M(4,4) = 0.88*cos(theta1)*sin(theta1) - 0.028*cos(theta5)*sin(theta5) + 3.14*cos(theta1)^2 + 2.82*cos(theta2)^2 + 2.82*cos(theta3)^2 + 2.82*cos(theta4)^2 - 0.0672*cos(theta5)^2 - 3.14*cos(theta1)^2*cos(theta2)^2 - 3.14*cos(theta1)^2*cos(theta3)^2 - 3.14*cos(theta1)^2*cos(theta4)^2 - 5.64*cos(theta2)^2*cos(theta3)^2 - 5.64*cos(theta2)^2*cos(theta4)^2 - 5.64*cos(theta3)^2*cos(theta4)^2 + 6.28*cos(theta1)^2*cos(theta2)^2*cos(theta3)^2 + 6.28*cos(theta1)^2*cos(theta2)^2*cos(theta4)^2 + 6.28*cos(theta1)^2*cos(theta3)^2*cos(theta4)^2 + 11.28*cos(theta2)^2*cos(theta3)^2*cos(theta4)^2 - 1.4*cos(theta2)*sin(theta1)*sin(theta2) - 1.4*cos(theta3)*sin(theta1)*sin(theta3) - 1.4*cos(theta4)*sin(theta1)*sin(theta4) - 0.88*cos(theta1)*cos(theta2)^2*sin(theta1) - 0.88*cos(theta1)*cos(theta3)^2*sin(theta1) - 0.88*cos(theta1)*cos(theta4)^2*sin(theta1) - 0.2*cos(theta1)*cos(theta2)*sin(theta2) - 0.2*cos(theta1)*cos(theta3)*sin(theta3) - 0.2*cos(theta1)*cos(theta4)*sin(theta4) + 0.4*cos(theta1)*cos(theta2)*cos(theta3)^2*sin(theta2) + 0.4*cos(theta1)*cos(theta2)*cos(theta4)^2*sin(theta2) + 0.4*cos(theta1)*cos(theta2)^2*cos(theta3)*sin(theta3) + 0.4*cos(theta1)*cos(theta3)*cos(theta4)^2*sin(theta3) + 0.4*cos(theta1)*cos(theta2)^2*cos(theta4)*sin(theta4) + 0.4*cos(theta1)*cos(theta3)^2*cos(theta4)*sin(theta4) - 12.56*cos(theta1)^2*cos(theta2)^2*cos(theta3)^2*cos(theta4)^2 + 2.8*cos(theta2)*cos(theta3)^2*sin(theta1)*sin(theta2) + 2.8*cos(theta2)*cos(theta4)^2*sin(theta1)*sin(theta2) + 2.8*cos(theta2)^2*cos(theta3)*sin(theta1)*sin(theta3) + 2.8*cos(theta3)*cos(theta4)^2*sin(theta1)*sin(theta3) + 2.8*cos(theta2)^2*cos(theta4)*sin(theta1)*sin(theta4) + 2.8*cos(theta3)^2*cos(theta4)*sin(theta1)*sin(theta4) + 1.76*cos(theta1)*cos(theta2)^2*cos(theta3)^2*sin(theta1) + 1.76*cos(theta1)*cos(theta2)^2*cos(theta4)^2*sin(theta1) + 1.76*cos(theta1)*cos(theta3)^2*cos(theta4)^2*sin(theta1) + 5.64*cos(theta2)*cos(theta3)*sin(theta2)*sin(theta3) + 5.64*cos(theta2)*cos(theta4)*sin(theta2)*sin(theta4) + 5.64*cos(theta3)*cos(theta4)*sin(theta3)*sin(theta4) - 6.28*cos(theta1)^2*cos(theta2)*cos(theta3)*sin(theta2)*sin(theta3) - 6.28*cos(theta1)^2*cos(theta2)*cos(theta4)*sin(theta2)*sin(theta4) - 11.28*cos(theta2)*cos(theta3)*cos(theta4)^2*sin(theta2)*sin(theta3) - 11.28*cos(theta2)*cos(theta3)^2*cos(theta4)*sin(theta2)*sin(theta4) - 6.28*cos(theta1)^2*cos(theta3)*cos(theta4)*sin(theta3)*sin(theta4) - 11.28*cos(theta2)^2*cos(theta3)*cos(theta4)*sin(theta3)*sin(theta4) - 0.8*cos(theta1)*cos(theta2)*cos(theta3)^2*cos(theta4)^2*sin(theta2) - 0.8*cos(theta1)*cos(theta2)^2*cos(theta3)*cos(theta4)^2*sin(theta3) - 0.8*cos(theta1)*cos(theta2)^2*cos(theta3)^2*cos(theta4)*sin(theta4) - 5.6*cos(theta2)*cos(theta3)^2*cos(theta4)^2*sin(theta1)*sin(theta2) - 5.6*cos(theta2)^2*cos(theta3)*cos(theta4)^2*sin(theta1)*sin(theta3) - 5.6*cos(theta2)^2*cos(theta3)^2*cos(theta4)*sin(theta1)*sin(theta4) - 3.52*cos(theta1)*cos(theta2)^2*cos(theta3)^2*cos(theta4)^2*sin(theta1) + 12.56*cos(theta1)^2*cos(theta2)*cos(theta3)*cos(theta4)^2*sin(theta2)*sin(theta3) + 12.56*cos(theta1)^2*cos(theta2)*cos(theta3)^2*cos(theta4)*sin(theta2)*sin(theta4) + 12.56*cos(theta1)^2*cos(theta2)^2*cos(theta3)*cos(theta4)*sin(theta3)*sin(theta4) - 1.76*cos(theta1)*cos(theta2)*cos(theta3)*sin(theta1)*sin(theta2)*sin(theta3) - 1.76*cos(theta1)*cos(theta2)*cos(theta4)*sin(theta1)*sin(theta2)*sin(theta4) - 1.76*cos(theta1)*cos(theta3)*cos(theta4)*sin(theta1)*sin(theta3)*sin(theta4) + 0.8*cos(theta1)*cos(theta2)*cos(theta3)*cos(theta4)*sin(theta2)*sin(theta3)*sin(theta4) + 5.6*cos(theta2)*cos(theta3)*cos(theta4)*sin(theta1)*sin(theta2)*sin(theta3)*sin(theta4) + 3.52*cos(theta1)*cos(theta2)*cos(theta3)*cos(theta4)^2*sin(theta1)*sin(theta2)*sin(theta3) + 3.52*cos(theta1)*cos(theta2)*cos(theta3)^2*cos(theta4)*sin(theta1)*sin(theta2)*sin(theta4) + 3.52*cos(theta1)*cos(theta2)^2*cos(theta3)*cos(theta4)*sin(theta1)*sin(theta3)*sin(theta4) + 0.6668 ;
M(4,5) = 0.049*cos(theta5) + 0.0098*sin(theta5) + 0.44*cos(theta1)*sin(theta1) + 1.57*cos(theta1)^2 + 1.41*cos(theta2)^2 + 1.41*cos(theta3)^2 + 1.41*cos(theta4)^2 - 1.57*cos(theta1)^2*cos(theta2)^2 - 1.57*cos(theta1)^2*cos(theta3)^2 - 1.57*cos(theta1)^2*cos(theta4)^2 - 2.82*cos(theta2)^2*cos(theta3)^2 - 2.82*cos(theta2)^2*cos(theta4)^2 - 2.82*cos(theta3)^2*cos(theta4)^2 + 3.14*cos(theta1)^2*cos(theta2)^2*cos(theta3)^2 + 3.14*cos(theta1)^2*cos(theta2)^2*cos(theta4)^2 + 3.14*cos(theta1)^2*cos(theta3)^2*cos(theta4)^2 + 5.64*cos(theta2)^2*cos(theta3)^2*cos(theta4)^2 - 0.7*cos(theta2)*sin(theta1)*sin(theta2) - 0.7*cos(theta3)*sin(theta1)*sin(theta3) - 0.7*cos(theta4)*sin(theta1)*sin(theta4) - 0.44*cos(theta1)*cos(theta2)^2*sin(theta1) - 0.44*cos(theta1)*cos(theta3)^2*sin(theta1) - 0.44*cos(theta1)*cos(theta4)^2*sin(theta1) - 0.1*cos(theta1)*cos(theta2)*sin(theta2) - 0.1*cos(theta1)*cos(theta3)*sin(theta3) - 0.1*cos(theta1)*cos(theta4)*sin(theta4) + 0.2*cos(theta1)*cos(theta2)*cos(theta3)^2*sin(theta2) + 0.2*cos(theta1)*cos(theta2)*cos(theta4)^2*sin(theta2) + 0.2*cos(theta1)*cos(theta2)^2*cos(theta3)*sin(theta3) + 0.2*cos(theta1)*cos(theta3)*cos(theta4)^2*sin(theta3) + 0.2*cos(theta1)*cos(theta2)^2*cos(theta4)*sin(theta4) + 0.2*cos(theta1)*cos(theta3)^2*cos(theta4)*sin(theta4) - 6.28*cos(theta1)^2*cos(theta2)^2*cos(theta3)^2*cos(theta4)^2 + 1.4*cos(theta2)*cos(theta3)^2*sin(theta1)*sin(theta2) + 1.4*cos(theta2)*cos(theta4)^2*sin(theta1)*sin(theta2) + 1.4*cos(theta2)^2*cos(theta3)*sin(theta1)*sin(theta3) + 1.4*cos(theta3)*cos(theta4)^2*sin(theta1)*sin(theta3) + 1.4*cos(theta2)^2*cos(theta4)*sin(theta1)*sin(theta4) + 1.4*cos(theta3)^2*cos(theta4)*sin(theta1)*sin(theta4) + 0.88*cos(theta1)*cos(theta2)^2*cos(theta3)^2*sin(theta1) + 0.88*cos(theta1)*cos(theta2)^2*cos(theta4)^2*sin(theta1) + 0.88*cos(theta1)*cos(theta3)^2*cos(theta4)^2*sin(theta1) + 2.82*cos(theta2)*cos(theta3)*sin(theta2)*sin(theta3) + 2.82*cos(theta2)*cos(theta4)*sin(theta2)*sin(theta4) + 2.82*cos(theta3)*cos(theta4)*sin(theta3)*sin(theta4) - 3.14*cos(theta1)^2*cos(theta2)*cos(theta3)*sin(theta2)*sin(theta3) - 3.14*cos(theta1)^2*cos(theta2)*cos(theta4)*sin(theta2)*sin(theta4) - 5.64*cos(theta2)*cos(theta3)*cos(theta4)^2*sin(theta2)*sin(theta3) - 5.64*cos(theta2)*cos(theta3)^2*cos(theta4)*sin(theta2)*sin(theta4) - 3.14*cos(theta1)^2*cos(theta3)*cos(theta4)*sin(theta3)*sin(theta4) - 5.64*cos(theta2)^2*cos(theta3)*cos(theta4)*sin(theta3)*sin(theta4) - 0.4*cos(theta1)*cos(theta2)*cos(theta3)^2*cos(theta4)^2*sin(theta2) - 0.4*cos(theta1)*cos(theta2)^2*cos(theta3)*cos(theta4)^2*sin(theta3) - 0.4*cos(theta1)*cos(theta2)^2*cos(theta3)^2*cos(theta4)*sin(theta4) - 2.8*cos(theta2)*cos(theta3)^2*cos(theta4)^2*sin(theta1)*sin(theta2) - 2.8*cos(theta2)^2*cos(theta3)*cos(theta4)^2*sin(theta1)*sin(theta3) - 2.8*cos(theta2)^2*cos(theta3)^2*cos(theta4)*sin(theta1)*sin(theta4) - 1.76*cos(theta1)*cos(theta2)^2*cos(theta3)^2*cos(theta4)^2*sin(theta1) + 6.28*cos(theta1)^2*cos(theta2)*cos(theta3)*cos(theta4)^2*sin(theta2)*sin(theta3) + 6.28*cos(theta1)^2*cos(theta2)*cos(theta3)^2*cos(theta4)*sin(theta2)*sin(theta4) + 6.28*cos(theta1)^2*cos(theta2)^2*cos(theta3)*cos(theta4)*sin(theta3)*sin(theta4) - 0.88*cos(theta1)*cos(theta2)*cos(theta3)*sin(theta1)*sin(theta2)*sin(theta3) - 0.88*cos(theta1)*cos(theta2)*cos(theta4)*sin(theta1)*sin(theta2)*sin(theta4) - 0.88*cos(theta1)*cos(theta3)*cos(theta4)*sin(theta1)*sin(theta3)*sin(theta4) + 0.4*cos(theta1)*cos(theta2)*cos(theta3)*cos(theta4)*sin(theta2)*sin(theta3)*sin(theta4) + 2.8*cos(theta2)*cos(theta3)*cos(theta4)*sin(theta1)*sin(theta2)*sin(theta3)*sin(theta4) + 1.76*cos(theta1)*cos(theta2)*cos(theta3)*cos(theta4)^2*sin(theta1)*sin(theta2)*sin(theta3) + 1.76*cos(theta1)*cos(theta2)*cos(theta3)^2*cos(theta4)*sin(theta1)*sin(theta2)*sin(theta4) + 1.76*cos(theta1)*cos(theta2)^2*cos(theta3)*cos(theta4)*sin(theta1)*sin(theta3)*sin(theta4) + 0.22 ;
M(5,1) = 0.014*cos(theta2)*cos(theta5) - 0.07*cos(theta2)*sin(theta5) - 0.0728*cos(theta2)*sin(theta3)*sin(theta4) - 0.0728*cos(theta3)*sin(theta2)*sin(theta4) - 0.0728*cos(theta4)*sin(theta2)*sin(theta3) - 0.014*cos(theta5)*sin(theta2)*sin(theta3) + 0.22*sin(theta2)*sin(theta3)*sin(theta4) + 0.07*sin(theta2)*sin(theta3)*sin(theta5) + 0.0728*cos(theta2)*cos(theta3)*cos(theta4) + 0.014*cos(theta2)*cos(theta3)*cos(theta5) - 0.22*cos(theta2)*cos(theta3)*sin(theta4) - 0.22*cos(theta2)*cos(theta4)*sin(theta3) - 0.22*cos(theta3)*cos(theta4)*sin(theta2) - 0.07*cos(theta2)*cos(theta3)*sin(theta5) + 0.44*cos(theta1)^2*cos(theta2)*cos(theta3)*sin(theta4) + 0.44*cos(theta1)^2*cos(theta2)*cos(theta4)*sin(theta3) + 0.44*cos(theta1)^2*cos(theta3)*cos(theta4)*sin(theta2) - 0.44*cos(theta1)^2*sin(theta2)*sin(theta3)*sin(theta4) - 0.35*cos(theta1)*cos(theta2)*cos(theta3)*cos(theta4) + 0.05*cos(theta2)*cos(theta3)*cos(theta4)*sin(theta1) - 0.0098*cos(theta2)*cos(theta3)*cos(theta5)*sin(theta4) - 0.0098*cos(theta2)*cos(theta4)*cos(theta5)*sin(theta3) - 0.0098*cos(theta3)*cos(theta4)*cos(theta5)*sin(theta2) + 0.35*cos(theta1)*cos(theta2)*sin(theta3)*sin(theta4) + 0.35*cos(theta1)*cos(theta3)*sin(theta2)*sin(theta4) + 0.35*cos(theta1)*cos(theta4)*sin(theta2)*sin(theta3) + 0.049*cos(theta2)*cos(theta3)*sin(theta4)*sin(theta5) + 0.049*cos(theta2)*cos(theta4)*sin(theta3)*sin(theta5) + 0.049*cos(theta3)*cos(theta4)*sin(theta2)*sin(theta5) - 0.05*cos(theta2)*sin(theta1)*sin(theta3)*sin(theta4) - 0.05*cos(theta3)*sin(theta1)*sin(theta2)*sin(theta4) - 0.05*cos(theta4)*sin(theta1)*sin(theta2)*sin(theta3) + 0.0098*cos(theta5)*sin(theta2)*sin(theta3)*sin(theta4) - 0.049*sin(theta2)*sin(theta3)*sin(theta4)*sin(theta5) - 1.57*cos(theta1)*cos(theta2)*cos(theta3)*sin(theta1)*sin(theta4) - 1.57*cos(theta1)*cos(theta2)*cos(theta4)*sin(theta1)*sin(theta3) - 1.57*cos(theta1)*cos(theta3)*cos(theta4)*sin(theta1)*sin(theta2) + 1.57*cos(theta1)*sin(theta1)*sin(theta2)*sin(theta3)*sin(theta4) ;
M(5,2) = 0.049*cos(theta5) + 0.0098*sin(theta5) - 0.07*cos(theta5)*sin(theta4) - 0.014*sin(theta4)*sin(theta5) - 0.014*cos(theta3)*sin(theta4)*sin(theta5) - 0.014*cos(theta4)*sin(theta3)*sin(theta5) + 0.22*sin(theta2)*sin(theta3)*sin(theta4) - 0.22*cos(theta2)*cos(theta3)*sin(theta4) - 0.22*cos(theta2)*cos(theta4)*sin(theta3) - 0.22*cos(theta3)*cos(theta4)*sin(theta2) - 0.07*cos(theta3)*cos(theta5)*sin(theta4) - 0.07*cos(theta4)*cos(theta5)*sin(theta3) + 0.44*cos(theta1)^2*cos(theta2)*cos(theta3)*sin(theta4) + 0.44*cos(theta1)^2*cos(theta2)*cos(theta4)*sin(theta3) + 0.44*cos(theta1)^2*cos(theta3)*cos(theta4)*sin(theta2) - 0.44*cos(theta1)^2*sin(theta2)*sin(theta3)*sin(theta4) - 0.35*cos(theta1)*cos(theta2)*cos(theta3)*cos(theta4) + 0.05*cos(theta2)*cos(theta3)*cos(theta4)*sin(theta1) + 0.35*cos(theta1)*cos(theta2)*sin(theta3)*sin(theta4) + 0.35*cos(theta1)*cos(theta3)*sin(theta2)*sin(theta4) + 0.35*cos(theta1)*cos(theta4)*sin(theta2)*sin(theta3) - 0.05*cos(theta2)*sin(theta1)*sin(theta3)*sin(theta4) - 0.05*cos(theta3)*sin(theta1)*sin(theta2)*sin(theta4) - 0.05*cos(theta4)*sin(theta1)*sin(theta2)*sin(theta3) - 1.57*cos(theta1)*cos(theta2)*cos(theta3)*sin(theta1)*sin(theta4) - 1.57*cos(theta1)*cos(theta2)*cos(theta4)*sin(theta1)*sin(theta3) - 1.57*cos(theta1)*cos(theta3)*cos(theta4)*sin(theta1)*sin(theta2) + 1.57*cos(theta1)*sin(theta1)*sin(theta2)*sin(theta3)*sin(theta4) ;
M(5,3) = 0.049*cos(theta5) + 0.0098*sin(theta5) - 0.07*cos(theta5)*sin(theta4) - 0.014*sin(theta4)*sin(theta5) + 0.22*sin(theta2)*sin(theta3)*sin(theta4) - 0.22*cos(theta2)*cos(theta3)*sin(theta4) - 0.22*cos(theta2)*cos(theta4)*sin(theta3) - 0.22*cos(theta3)*cos(theta4)*sin(theta2) + 0.44*cos(theta1)^2*cos(theta2)*cos(theta3)*sin(theta4) + 0.44*cos(theta1)^2*cos(theta2)*cos(theta4)*sin(theta3) + 0.44*cos(theta1)^2*cos(theta3)*cos(theta4)*sin(theta2) - 0.44*cos(theta1)^2*sin(theta2)*sin(theta3)*sin(theta4) - 0.35*cos(theta1)*cos(theta2)*cos(theta3)*cos(theta4) + 0.05*cos(theta2)*cos(theta3)*cos(theta4)*sin(theta1) + 0.35*cos(theta1)*cos(theta2)*sin(theta3)*sin(theta4) + 0.35*cos(theta1)*cos(theta3)*sin(theta2)*sin(theta4) + 0.35*cos(theta1)*cos(theta4)*sin(theta2)*sin(theta3) - 0.05*cos(theta2)*sin(theta1)*sin(theta3)*sin(theta4) - 0.05*cos(theta3)*sin(theta1)*sin(theta2)*sin(theta4) - 0.05*cos(theta4)*sin(theta1)*sin(theta2)*sin(theta3) - 1.57*cos(theta1)*cos(theta2)*cos(theta3)*sin(theta1)*sin(theta4) - 1.57*cos(theta1)*cos(theta2)*cos(theta4)*sin(theta1)*sin(theta3) - 1.57*cos(theta1)*cos(theta3)*cos(theta4)*sin(theta1)*sin(theta2) + 1.57*cos(theta1)*sin(theta1)*sin(theta2)*sin(theta3)*sin(theta4) ;
M(5,4) = 0.049*cos(theta5) + 0.0098*sin(theta5) + 0.44*cos(theta1)*sin(theta1) + 1.57*cos(theta1)^2 + 1.41*cos(theta2)^2 + 1.41*cos(theta3)^2 + 1.41*cos(theta4)^2 - 1.57*cos(theta1)^2*cos(theta2)^2 - 1.57*cos(theta1)^2*cos(theta3)^2 - 1.57*cos(theta1)^2*cos(theta4)^2 - 2.82*cos(theta2)^2*cos(theta3)^2 - 2.82*cos(theta2)^2*cos(theta4)^2 - 2.82*cos(theta3)^2*cos(theta4)^2 + 3.14*cos(theta1)^2*cos(theta2)^2*cos(theta3)^2 + 3.14*cos(theta1)^2*cos(theta2)^2*cos(theta4)^2 + 3.14*cos(theta1)^2*cos(theta3)^2*cos(theta4)^2 + 5.64*cos(theta2)^2*cos(theta3)^2*cos(theta4)^2 - 0.7*cos(theta2)*sin(theta1)*sin(theta2) - 0.7*cos(theta3)*sin(theta1)*sin(theta3) - 0.7*cos(theta4)*sin(theta1)*sin(theta4) - 0.44*cos(theta1)*cos(theta2)^2*sin(theta1) - 0.44*cos(theta1)*cos(theta3)^2*sin(theta1) - 0.44*cos(theta1)*cos(theta4)^2*sin(theta1) - 0.1*cos(theta1)*cos(theta2)*sin(theta2) - 0.1*cos(theta1)*cos(theta3)*sin(theta3) - 0.1*cos(theta1)*cos(theta4)*sin(theta4) + 0.2*cos(theta1)*cos(theta2)*cos(theta3)^2*sin(theta2) + 0.2*cos(theta1)*cos(theta2)*cos(theta4)^2*sin(theta2) + 0.2*cos(theta1)*cos(theta2)^2*cos(theta3)*sin(theta3) + 0.2*cos(theta1)*cos(theta3)*cos(theta4)^2*sin(theta3) + 0.2*cos(theta1)*cos(theta2)^2*cos(theta4)*sin(theta4) + 0.2*cos(theta1)*cos(theta3)^2*cos(theta4)*sin(theta4) - 6.28*cos(theta1)^2*cos(theta2)^2*cos(theta3)^2*cos(theta4)^2 + 1.4*cos(theta2)*cos(theta3)^2*sin(theta1)*sin(theta2) + 1.4*cos(theta2)*cos(theta4)^2*sin(theta1)*sin(theta2) + 1.4*cos(theta2)^2*cos(theta3)*sin(theta1)*sin(theta3) + 1.4*cos(theta3)*cos(theta4)^2*sin(theta1)*sin(theta3) + 1.4*cos(theta2)^2*cos(theta4)*sin(theta1)*sin(theta4) + 1.4*cos(theta3)^2*cos(theta4)*sin(theta1)*sin(theta4) + 0.88*cos(theta1)*cos(theta2)^2*cos(theta3)^2*sin(theta1) + 0.88*cos(theta1)*cos(theta2)^2*cos(theta4)^2*sin(theta1) + 0.88*cos(theta1)*cos(theta3)^2*cos(theta4)^2*sin(theta1) + 2.82*cos(theta2)*cos(theta3)*sin(theta2)*sin(theta3) + 2.82*cos(theta2)*cos(theta4)*sin(theta2)*sin(theta4) + 2.82*cos(theta3)*cos(theta4)*sin(theta3)*sin(theta4) - 3.14*cos(theta1)^2*cos(theta2)*cos(theta3)*sin(theta2)*sin(theta3) - 3.14*cos(theta1)^2*cos(theta2)*cos(theta4)*sin(theta2)*sin(theta4) - 5.64*cos(theta2)*cos(theta3)*cos(theta4)^2*sin(theta2)*sin(theta3) - 5.64*cos(theta2)*cos(theta3)^2*cos(theta4)*sin(theta2)*sin(theta4) - 3.14*cos(theta1)^2*cos(theta3)*cos(theta4)*sin(theta3)*sin(theta4) - 5.64*cos(theta2)^2*cos(theta3)*cos(theta4)*sin(theta3)*sin(theta4) - 0.4*cos(theta1)*cos(theta2)*cos(theta3)^2*cos(theta4)^2*sin(theta2) - 0.4*cos(theta1)*cos(theta2)^2*cos(theta3)*cos(theta4)^2*sin(theta3) - 0.4*cos(theta1)*cos(theta2)^2*cos(theta3)^2*cos(theta4)*sin(theta4) - 2.8*cos(theta2)*cos(theta3)^2*cos(theta4)^2*sin(theta1)*sin(theta2) - 2.8*cos(theta2)^2*cos(theta3)*cos(theta4)^2*sin(theta1)*sin(theta3) - 2.8*cos(theta2)^2*cos(theta3)^2*cos(theta4)*sin(theta1)*sin(theta4) - 1.76*cos(theta1)*cos(theta2)^2*cos(theta3)^2*cos(theta4)^2*sin(theta1) + 6.28*cos(theta1)^2*cos(theta2)*cos(theta3)*cos(theta4)^2*sin(theta2)*sin(theta3) + 6.28*cos(theta1)^2*cos(theta2)*cos(theta3)^2*cos(theta4)*sin(theta2)*sin(theta4) + 6.28*cos(theta1)^2*cos(theta2)^2*cos(theta3)*cos(theta4)*sin(theta3)*sin(theta4) - 0.88*cos(theta1)*cos(theta2)*cos(theta3)*sin(theta1)*sin(theta2)*sin(theta3) - 0.88*cos(theta1)*cos(theta2)*cos(theta4)*sin(theta1)*sin(theta2)*sin(theta4) - 0.88*cos(theta1)*cos(theta3)*cos(theta4)*sin(theta1)*sin(theta3)*sin(theta4) + 0.4*cos(theta1)*cos(theta2)*cos(theta3)*cos(theta4)*sin(theta2)*sin(theta3)*sin(theta4) + 2.8*cos(theta2)*cos(theta3)*cos(theta4)*sin(theta1)*sin(theta2)*sin(theta3)*sin(theta4) + 1.76*cos(theta1)*cos(theta2)*cos(theta3)*cos(theta4)^2*sin(theta1)*sin(theta2)*sin(theta3) + 1.76*cos(theta1)*cos(theta2)*cos(theta3)^2*cos(theta4)*sin(theta1)*sin(theta2)*sin(theta4) + 1.76*cos(theta1)*cos(theta2)^2*cos(theta3)*cos(theta4)*sin(theta1)*sin(theta3)*sin(theta4) + 0.22 ;
M(5,5) = 0.44*cos(theta1)*sin(theta1) + 1.57*cos(theta1)^2 + 1.41*cos(theta2)^2 + 1.41*cos(theta3)^2 + 1.41*cos(theta4)^2 - 1.57*cos(theta1)^2*cos(theta2)^2 - 1.57*cos(theta1)^2*cos(theta3)^2 - 1.57*cos(theta1)^2*cos(theta4)^2 - 2.82*cos(theta2)^2*cos(theta3)^2 - 2.82*cos(theta2)^2*cos(theta4)^2 - 2.82*cos(theta3)^2*cos(theta4)^2 + 3.14*cos(theta1)^2*cos(theta2)^2*cos(theta3)^2 + 3.14*cos(theta1)^2*cos(theta2)^2*cos(theta4)^2 + 3.14*cos(theta1)^2*cos(theta3)^2*cos(theta4)^2 + 5.64*cos(theta2)^2*cos(theta3)^2*cos(theta4)^2 - 0.7*cos(theta2)*sin(theta1)*sin(theta2) - 0.7*cos(theta3)*sin(theta1)*sin(theta3) - 0.7*cos(theta4)*sin(theta1)*sin(theta4) - 0.44*cos(theta1)*cos(theta2)^2*sin(theta1) - 0.44*cos(theta1)*cos(theta3)^2*sin(theta1) - 0.44*cos(theta1)*cos(theta4)^2*sin(theta1) - 0.1*cos(theta1)*cos(theta2)*sin(theta2) - 0.1*cos(theta1)*cos(theta3)*sin(theta3) - 0.1*cos(theta1)*cos(theta4)*sin(theta4) + 0.2*cos(theta1)*cos(theta2)*cos(theta3)^2*sin(theta2) + 0.2*cos(theta1)*cos(theta2)*cos(theta4)^2*sin(theta2) + 0.2*cos(theta1)*cos(theta2)^2*cos(theta3)*sin(theta3) + 0.2*cos(theta1)*cos(theta3)*cos(theta4)^2*sin(theta3) + 0.2*cos(theta1)*cos(theta2)^2*cos(theta4)*sin(theta4) + 0.2*cos(theta1)*cos(theta3)^2*cos(theta4)*sin(theta4) - 6.28*cos(theta1)^2*cos(theta2)^2*cos(theta3)^2*cos(theta4)^2 + 1.4*cos(theta2)*cos(theta3)^2*sin(theta1)*sin(theta2) + 1.4*cos(theta2)*cos(theta4)^2*sin(theta1)*sin(theta2) + 1.4*cos(theta2)^2*cos(theta3)*sin(theta1)*sin(theta3) + 1.4*cos(theta3)*cos(theta4)^2*sin(theta1)*sin(theta3) + 1.4*cos(theta2)^2*cos(theta4)*sin(theta1)*sin(theta4) + 1.4*cos(theta3)^2*cos(theta4)*sin(theta1)*sin(theta4) + 0.88*cos(theta1)*cos(theta2)^2*cos(theta3)^2*sin(theta1) + 0.88*cos(theta1)*cos(theta2)^2*cos(theta4)^2*sin(theta1) + 0.88*cos(theta1)*cos(theta3)^2*cos(theta4)^2*sin(theta1) + 2.82*cos(theta2)*cos(theta3)*sin(theta2)*sin(theta3) + 2.82*cos(theta2)*cos(theta4)*sin(theta2)*sin(theta4) + 2.82*cos(theta3)*cos(theta4)*sin(theta3)*sin(theta4) - 3.14*cos(theta1)^2*cos(theta2)*cos(theta3)*sin(theta2)*sin(theta3) - 3.14*cos(theta1)^2*cos(theta2)*cos(theta4)*sin(theta2)*sin(theta4) - 5.64*cos(theta2)*cos(theta3)*cos(theta4)^2*sin(theta2)*sin(theta3) - 5.64*cos(theta2)*cos(theta3)^2*cos(theta4)*sin(theta2)*sin(theta4) - 3.14*cos(theta1)^2*cos(theta3)*cos(theta4)*sin(theta3)*sin(theta4) - 5.64*cos(theta2)^2*cos(theta3)*cos(theta4)*sin(theta3)*sin(theta4) - 0.4*cos(theta1)*cos(theta2)*cos(theta3)^2*cos(theta4)^2*sin(theta2) - 0.4*cos(theta1)*cos(theta2)^2*cos(theta3)*cos(theta4)^2*sin(theta3) - 0.4*cos(theta1)*cos(theta2)^2*cos(theta3)^2*cos(theta4)*sin(theta4) - 2.8*cos(theta2)*cos(theta3)^2*cos(theta4)^2*sin(theta1)*sin(theta2) - 2.8*cos(theta2)^2*cos(theta3)*cos(theta4)^2*sin(theta1)*sin(theta3) - 2.8*cos(theta2)^2*cos(theta3)^2*cos(theta4)*sin(theta1)*sin(theta4) - 1.76*cos(theta1)*cos(theta2)^2*cos(theta3)^2*cos(theta4)^2*sin(theta1) + 6.28*cos(theta1)^2*cos(theta2)*cos(theta3)*cos(theta4)^2*sin(theta2)*sin(theta3) + 6.28*cos(theta1)^2*cos(theta2)*cos(theta3)^2*cos(theta4)*sin(theta2)*sin(theta4) + 6.28*cos(theta1)^2*cos(theta2)^2*cos(theta3)*cos(theta4)*sin(theta3)*sin(theta4) - 0.88*cos(theta1)*cos(theta2)*cos(theta3)*sin(theta1)*sin(theta2)*sin(theta3) - 0.88*cos(theta1)*cos(theta2)*cos(theta4)*sin(theta1)*sin(theta2)*sin(theta4) - 0.88*cos(theta1)*cos(theta3)*cos(theta4)*sin(theta1)*sin(theta3)*sin(theta4) + 0.4*cos(theta1)*cos(theta2)*cos(theta3)*cos(theta4)*sin(theta2)*sin(theta3)*sin(theta4) + 2.8*cos(theta2)*cos(theta3)*cos(theta4)*sin(theta1)*sin(theta2)*sin(theta3)*sin(theta4) + 1.76*cos(theta1)*cos(theta2)*cos(theta3)*cos(theta4)^2*sin(theta1)*sin(theta2)*sin(theta3) + 1.76*cos(theta1)*cos(theta2)*cos(theta3)^2*cos(theta4)*sin(theta1)*sin(theta2)*sin(theta4) + 1.76*cos(theta1)*cos(theta2)^2*cos(theta3)*cos(theta4)*sin(theta1)*sin(theta3)*sin(theta4) + 0.2928 ;



C=zeros(5);
C(1,1) = 2.24*thetad1*cos(theta1)^2 - 1.1*thetad2 - 1.04*thetad3 - 1.12*thetad1 + 2.2*thetad2*cos(theta1)^2 + 2.08*thetad3*cos(theta1)^2 - 7.08*thetad1*cos(theta1)*sin(theta1) - 7.08*thetad2*cos(theta1)*sin(theta1) - 6.86*thetad3*cos(theta1)*sin(theta1) - 3.14*thetad4*cos(theta2)*cos(theta3)*sin(theta4) - 3.14*thetad4*cos(theta2)*cos(theta4)*sin(theta3) - 3.14*thetad4*cos(theta3)*cos(theta4)*sin(theta2) - 1.57*thetad5*cos(theta2)*cos(theta3)*sin(theta4) - 1.57*thetad5*cos(theta2)*cos(theta4)*sin(theta3) - 1.57*thetad5*cos(theta3)*cos(theta4)*sin(theta2) + 3.14*thetad4*sin(theta2)*sin(theta3)*sin(theta4) + 1.57*thetad5*sin(theta2)*sin(theta3)*sin(theta4) - 0.1*thetad4*cos(theta1)*cos(theta2)*cos(theta3)*cos(theta4) - 0.05*thetad5*cos(theta1)*cos(theta2)*cos(theta3)*cos(theta4) - 0.7*thetad4*cos(theta2)*cos(theta3)*cos(theta4)*sin(theta1) - 0.35*thetad5*cos(theta2)*cos(theta3)*cos(theta4)*sin(theta1) + 0.1*thetad4*cos(theta1)*cos(theta2)*sin(theta3)*sin(theta4) + 0.1*thetad4*cos(theta1)*cos(theta3)*sin(theta2)*sin(theta4) + 0.1*thetad4*cos(theta1)*cos(theta4)*sin(theta2)*sin(theta3) + 0.05*thetad5*cos(theta1)*cos(theta2)*sin(theta3)*sin(theta4) + 0.05*thetad5*cos(theta1)*cos(theta3)*sin(theta2)*sin(theta4) + 0.05*thetad5*cos(theta1)*cos(theta4)*sin(theta2)*sin(theta3) + 0.7*thetad4*cos(theta2)*sin(theta1)*sin(theta3)*sin(theta4) + 0.7*thetad4*cos(theta3)*sin(theta1)*sin(theta2)*sin(theta4) + 0.7*thetad4*cos(theta4)*sin(theta1)*sin(theta2)*sin(theta3) + 0.35*thetad5*cos(theta2)*sin(theta1)*sin(theta3)*sin(theta4) + 0.35*thetad5*cos(theta3)*sin(theta1)*sin(theta2)*sin(theta4) + 0.35*thetad5*cos(theta4)*sin(theta1)*sin(theta2)*sin(theta3) + 6.28*thetad4*cos(theta1)^2*cos(theta2)*cos(theta3)*sin(theta4) + 6.28*thetad4*cos(theta1)^2*cos(theta2)*cos(theta4)*sin(theta3) + 6.28*thetad4*cos(theta1)^2*cos(theta3)*cos(theta4)*sin(theta2) + 3.14*thetad5*cos(theta1)^2*cos(theta2)*cos(theta3)*sin(theta4) + 3.14*thetad5*cos(theta1)^2*cos(theta2)*cos(theta4)*sin(theta3) + 3.14*thetad5*cos(theta1)^2*cos(theta3)*cos(theta4)*sin(theta2) - 6.28*thetad4*cos(theta1)^2*sin(theta2)*sin(theta3)*sin(theta4) - 3.14*thetad5*cos(theta1)^2*sin(theta2)*sin(theta3)*sin(theta4) + 1.76*thetad4*cos(theta1)*cos(theta2)*cos(theta3)*sin(theta1)*sin(theta4) + 1.76*thetad4*cos(theta1)*cos(theta2)*cos(theta4)*sin(theta1)*sin(theta3) + 1.76*thetad4*cos(theta1)*cos(theta3)*cos(theta4)*sin(theta1)*sin(theta2) + 0.88*thetad5*cos(theta1)*cos(theta2)*cos(theta3)*sin(theta1)*sin(theta4) + 0.88*thetad5*cos(theta1)*cos(theta2)*cos(theta4)*sin(theta1)*sin(theta3) + 0.88*thetad5*cos(theta1)*cos(theta3)*cos(theta4)*sin(theta1)*sin(theta2) - 1.76*thetad4*cos(theta1)*sin(theta1)*sin(theta2)*sin(theta3)*sin(theta4) - 0.88*thetad5*cos(theta1)*sin(theta1)*sin(theta2)*sin(theta3)*sin(theta4) ;
C(1,2) = 2.2*thetad1*cos(theta1)^2 - 1.1*thetad2 - 1.04*thetad3 - 1.1*thetad1 + 2.2*thetad2*cos(theta1)^2 + 2.08*thetad3*cos(theta1)^2 - 7.08*thetad1*cos(theta1)*sin(theta1) - 7.08*thetad2*cos(theta1)*sin(theta1) - 6.86*thetad3*cos(theta1)*sin(theta1) - 3.14*thetad4*cos(theta2)*cos(theta3)*sin(theta4) - 3.14*thetad4*cos(theta2)*cos(theta4)*sin(theta3) - 3.14*thetad4*cos(theta3)*cos(theta4)*sin(theta2) - 1.57*thetad5*cos(theta2)*cos(theta3)*sin(theta4) - 1.57*thetad5*cos(theta2)*cos(theta4)*sin(theta3) - 1.57*thetad5*cos(theta3)*cos(theta4)*sin(theta2) + 3.14*thetad4*sin(theta2)*sin(theta3)*sin(theta4) + 1.57*thetad5*sin(theta2)*sin(theta3)*sin(theta4) - 0.1*thetad4*cos(theta1)*cos(theta2)*cos(theta3)*cos(theta4) - 0.05*thetad5*cos(theta1)*cos(theta2)*cos(theta3)*cos(theta4) - 0.7*thetad4*cos(theta2)*cos(theta3)*cos(theta4)*sin(theta1) - 0.35*thetad5*cos(theta2)*cos(theta3)*cos(theta4)*sin(theta1) + 0.1*thetad4*cos(theta1)*cos(theta2)*sin(theta3)*sin(theta4) + 0.1*thetad4*cos(theta1)*cos(theta3)*sin(theta2)*sin(theta4) + 0.1*thetad4*cos(theta1)*cos(theta4)*sin(theta2)*sin(theta3) + 0.05*thetad5*cos(theta1)*cos(theta2)*sin(theta3)*sin(theta4) + 0.05*thetad5*cos(theta1)*cos(theta3)*sin(theta2)*sin(theta4) + 0.05*thetad5*cos(theta1)*cos(theta4)*sin(theta2)*sin(theta3) + 0.7*thetad4*cos(theta2)*sin(theta1)*sin(theta3)*sin(theta4) + 0.7*thetad4*cos(theta3)*sin(theta1)*sin(theta2)*sin(theta4) + 0.7*thetad4*cos(theta4)*sin(theta1)*sin(theta2)*sin(theta3) + 0.35*thetad5*cos(theta2)*sin(theta1)*sin(theta3)*sin(theta4) + 0.35*thetad5*cos(theta3)*sin(theta1)*sin(theta2)*sin(theta4) + 0.35*thetad5*cos(theta4)*sin(theta1)*sin(theta2)*sin(theta3) + 6.28*thetad4*cos(theta1)^2*cos(theta2)*cos(theta3)*sin(theta4) + 6.28*thetad4*cos(theta1)^2*cos(theta2)*cos(theta4)*sin(theta3) + 6.28*thetad4*cos(theta1)^2*cos(theta3)*cos(theta4)*sin(theta2) + 3.14*thetad5*cos(theta1)^2*cos(theta2)*cos(theta3)*sin(theta4) + 3.14*thetad5*cos(theta1)^2*cos(theta2)*cos(theta4)*sin(theta3) + 3.14*thetad5*cos(theta1)^2*cos(theta3)*cos(theta4)*sin(theta2) - 6.28*thetad4*cos(theta1)^2*sin(theta2)*sin(theta3)*sin(theta4) - 3.14*thetad5*cos(theta1)^2*sin(theta2)*sin(theta3)*sin(theta4) + 1.76*thetad4*cos(theta1)*cos(theta2)*cos(theta3)*sin(theta1)*sin(theta4) + 1.76*thetad4*cos(theta1)*cos(theta2)*cos(theta4)*sin(theta1)*sin(theta3) + 1.76*thetad4*cos(theta1)*cos(theta3)*cos(theta4)*sin(theta1)*sin(theta2) + 0.88*thetad5*cos(theta1)*cos(theta2)*cos(theta3)*sin(theta1)*sin(theta4) + 0.88*thetad5*cos(theta1)*cos(theta2)*cos(theta4)*sin(theta1)*sin(theta3) + 0.88*thetad5*cos(theta1)*cos(theta3)*cos(theta4)*sin(theta1)*sin(theta2) - 1.76*thetad4*cos(theta1)*sin(theta1)*sin(theta2)*sin(theta3)*sin(theta4) - 0.88*thetad5*cos(theta1)*sin(theta1)*sin(theta2)*sin(theta3)*sin(theta4) ;
C(1,3) = 2.08*thetad1*cos(theta1)^2 - 1.04*thetad2 - 1.04*thetad3 - 1.04*thetad1 + 2.08*thetad2*cos(theta1)^2 + 2.08*thetad3*cos(theta1)^2 - 6.86*thetad1*cos(theta1)*sin(theta1) - 6.86*thetad2*cos(theta1)*sin(theta1) - 6.86*thetad3*cos(theta1)*sin(theta1) - 3.14*thetad4*cos(theta2)*cos(theta3)*sin(theta4) - 3.14*thetad4*cos(theta2)*cos(theta4)*sin(theta3) - 3.14*thetad4*cos(theta3)*cos(theta4)*sin(theta2) - 1.57*thetad5*cos(theta2)*cos(theta3)*sin(theta4) - 1.57*thetad5*cos(theta2)*cos(theta4)*sin(theta3) - 1.57*thetad5*cos(theta3)*cos(theta4)*sin(theta2) + 3.14*thetad4*sin(theta2)*sin(theta3)*sin(theta4) + 1.57*thetad5*sin(theta2)*sin(theta3)*sin(theta4) - 0.1*thetad4*cos(theta1)*cos(theta2)*cos(theta3)*cos(theta4) - 0.05*thetad5*cos(theta1)*cos(theta2)*cos(theta3)*cos(theta4) - 0.7*thetad4*cos(theta2)*cos(theta3)*cos(theta4)*sin(theta1) - 0.35*thetad5*cos(theta2)*cos(theta3)*cos(theta4)*sin(theta1) + 0.1*thetad4*cos(theta1)*cos(theta2)*sin(theta3)*sin(theta4) + 0.1*thetad4*cos(theta1)*cos(theta3)*sin(theta2)*sin(theta4) + 0.1*thetad4*cos(theta1)*cos(theta4)*sin(theta2)*sin(theta3) + 0.05*thetad5*cos(theta1)*cos(theta2)*sin(theta3)*sin(theta4) + 0.05*thetad5*cos(theta1)*cos(theta3)*sin(theta2)*sin(theta4) + 0.05*thetad5*cos(theta1)*cos(theta4)*sin(theta2)*sin(theta3) + 0.7*thetad4*cos(theta2)*sin(theta1)*sin(theta3)*sin(theta4) + 0.7*thetad4*cos(theta3)*sin(theta1)*sin(theta2)*sin(theta4) + 0.7*thetad4*cos(theta4)*sin(theta1)*sin(theta2)*sin(theta3) + 0.35*thetad5*cos(theta2)*sin(theta1)*sin(theta3)*sin(theta4) + 0.35*thetad5*cos(theta3)*sin(theta1)*sin(theta2)*sin(theta4) + 0.35*thetad5*cos(theta4)*sin(theta1)*sin(theta2)*sin(theta3) + 6.28*thetad4*cos(theta1)^2*cos(theta2)*cos(theta3)*sin(theta4) + 6.28*thetad4*cos(theta1)^2*cos(theta2)*cos(theta4)*sin(theta3) + 6.28*thetad4*cos(theta1)^2*cos(theta3)*cos(theta4)*sin(theta2) + 3.14*thetad5*cos(theta1)^2*cos(theta2)*cos(theta3)*sin(theta4) + 3.14*thetad5*cos(theta1)^2*cos(theta2)*cos(theta4)*sin(theta3) + 3.14*thetad5*cos(theta1)^2*cos(theta3)*cos(theta4)*sin(theta2) - 6.28*thetad4*cos(theta1)^2*sin(theta2)*sin(theta3)*sin(theta4) - 3.14*thetad5*cos(theta1)^2*sin(theta2)*sin(theta3)*sin(theta4) + 1.76*thetad4*cos(theta1)*cos(theta2)*cos(theta3)*sin(theta1)*sin(theta4) + 1.76*thetad4*cos(theta1)*cos(theta2)*cos(theta4)*sin(theta1)*sin(theta3) + 1.76*thetad4*cos(theta1)*cos(theta3)*cos(theta4)*sin(theta1)*sin(theta2) + 0.88*thetad5*cos(theta1)*cos(theta2)*cos(theta3)*sin(theta1)*sin(theta4) + 0.88*thetad5*cos(theta1)*cos(theta2)*cos(theta4)*sin(theta1)*sin(theta3) + 0.88*thetad5*cos(theta1)*cos(theta3)*cos(theta4)*sin(theta1)*sin(theta2) - 1.76*thetad4*cos(theta1)*sin(theta1)*sin(theta2)*sin(theta3)*sin(theta4) - 0.88*thetad5*cos(theta1)*sin(theta1)*sin(theta2)*sin(theta3)*sin(theta4) ;
C(1,4) = 0.88*thetad4 + 0.44*thetad5 - 1.76*thetad4*cos(theta1)^2 - 0.88*thetad4*cos(theta2)^2 - 0.88*thetad5*cos(theta1)^2 - 0.88*thetad4*cos(theta3)^2 - 0.44*thetad5*cos(theta2)^2 - 0.88*thetad4*cos(theta4)^2 - 0.44*thetad5*cos(theta3)^2 - 0.44*thetad5*cos(theta4)^2 + 1.76*thetad4*cos(theta1)^2*cos(theta2)^2 + 1.76*thetad4*cos(theta1)^2*cos(theta3)^2 + 0.88*thetad5*cos(theta1)^2*cos(theta2)^2 + 1.76*thetad4*cos(theta1)^2*cos(theta4)^2 + 1.76*thetad4*cos(theta2)^2*cos(theta3)^2 + 0.88*thetad5*cos(theta1)^2*cos(theta3)^2 + 1.76*thetad4*cos(theta2)^2*cos(theta4)^2 + 0.88*thetad5*cos(theta1)^2*cos(theta4)^2 + 0.88*thetad5*cos(theta2)^2*cos(theta3)^2 + 1.76*thetad4*cos(theta3)^2*cos(theta4)^2 + 0.88*thetad5*cos(theta2)^2*cos(theta4)^2 + 0.88*thetad5*cos(theta3)^2*cos(theta4)^2 + 6.28*thetad4*cos(theta1)*sin(theta1) + 3.14*thetad5*cos(theta1)*sin(theta1) + 1.4*thetad4*cos(theta1)*cos(theta2)*sin(theta2) - 3.14*thetad1*cos(theta2)*cos(theta3)*sin(theta4) - 3.14*thetad1*cos(theta2)*cos(theta4)*sin(theta3) - 3.14*thetad1*cos(theta3)*cos(theta4)*sin(theta2) + 0.7*thetad5*cos(theta1)*cos(theta2)*sin(theta2) - 3.14*thetad2*cos(theta2)*cos(theta3)*sin(theta4) - 3.14*thetad2*cos(theta2)*cos(theta4)*sin(theta3) - 3.14*thetad2*cos(theta3)*cos(theta4)*sin(theta2) + 1.4*thetad4*cos(theta1)*cos(theta3)*sin(theta3) - 3.14*thetad3*cos(theta2)*cos(theta3)*sin(theta4) - 3.14*thetad3*cos(theta2)*cos(theta4)*sin(theta3) - 3.14*thetad3*cos(theta3)*cos(theta4)*sin(theta2) + 0.7*thetad5*cos(theta1)*cos(theta3)*sin(theta3) + 1.4*thetad4*cos(theta1)*cos(theta4)*sin(theta4) + 0.7*thetad5*cos(theta1)*cos(theta4)*sin(theta4) - 3.52*thetad4*cos(theta1)^2*cos(theta2)^2*cos(theta3)^2 - 3.52*thetad4*cos(theta1)^2*cos(theta2)^2*cos(theta4)^2 - 1.76*thetad5*cos(theta1)^2*cos(theta2)^2*cos(theta3)^2 - 3.52*thetad4*cos(theta1)^2*cos(theta3)^2*cos(theta4)^2 - 1.76*thetad5*cos(theta1)^2*cos(theta2)^2*cos(theta4)^2 - 3.52*thetad4*cos(theta2)^2*cos(theta3)^2*cos(theta4)^2 - 1.76*thetad5*cos(theta1)^2*cos(theta3)^2*cos(theta4)^2 - 1.76*thetad5*cos(theta2)^2*cos(theta3)^2*cos(theta4)^2 - 0.2*thetad4*cos(theta2)*sin(theta1)*sin(theta2) - 0.1*thetad5*cos(theta2)*sin(theta1)*sin(theta2) - 0.2*thetad4*cos(theta3)*sin(theta1)*sin(theta3) - 0.1*thetad5*cos(theta3)*sin(theta1)*sin(theta3) - 0.2*thetad4*cos(theta4)*sin(theta1)*sin(theta4) - 0.1*thetad5*cos(theta4)*sin(theta1)*sin(theta4) + 3.14*thetad1*sin(theta2)*sin(theta3)*sin(theta4) + 3.14*thetad2*sin(theta2)*sin(theta3)*sin(theta4) + 3.14*thetad3*sin(theta2)*sin(theta3)*sin(theta4) - 6.28*thetad4*cos(theta1)*cos(theta2)^2*sin(theta1) - 6.28*thetad4*cos(theta1)*cos(theta3)^2*sin(theta1) - 3.14*thetad5*cos(theta1)*cos(theta2)^2*sin(theta1) - 6.28*thetad4*cos(theta1)*cos(theta4)^2*sin(theta1) - 3.14*thetad5*cos(theta1)*cos(theta3)^2*sin(theta1) - 3.14*thetad5*cos(theta1)*cos(theta4)^2*sin(theta1) + 12.56*thetad4*cos(theta1)*cos(theta2)^2*cos(theta3)^2*sin(theta1) + 12.56*thetad4*cos(theta1)*cos(theta2)^2*cos(theta4)^2*sin(theta1) + 6.28*thetad5*cos(theta1)*cos(theta2)^2*cos(theta3)^2*sin(theta1) + 12.56*thetad4*cos(theta1)*cos(theta3)^2*cos(theta4)^2*sin(theta1) + 6.28*thetad5*cos(theta1)*cos(theta2)^2*cos(theta4)^2*sin(theta1) + 6.28*thetad5*cos(theta1)*cos(theta3)^2*cos(theta4)^2*sin(theta1) - 0.1*thetad1*cos(theta1)*cos(theta2)*cos(theta3)*cos(theta4) - 0.1*thetad2*cos(theta1)*cos(theta2)*cos(theta3)*cos(theta4) - 0.1*thetad3*cos(theta1)*cos(theta2)*cos(theta3)*cos(theta4) - 0.7*thetad1*cos(theta2)*cos(theta3)*cos(theta4)*sin(theta1) - 0.7*thetad2*cos(theta2)*cos(theta3)*cos(theta4)*sin(theta1) - 0.7*thetad3*cos(theta2)*cos(theta3)*cos(theta4)*sin(theta1) + 0.1*thetad1*cos(theta1)*cos(theta2)*sin(theta3)*sin(theta4) + 0.1*thetad1*cos(theta1)*cos(theta3)*sin(theta2)*sin(theta4) + 0.1*thetad1*cos(theta1)*cos(theta4)*sin(theta2)*sin(theta3) + 0.1*thetad2*cos(theta1)*cos(theta2)*sin(theta3)*sin(theta4) + 0.1*thetad2*cos(theta1)*cos(theta3)*sin(theta2)*sin(theta4) + 0.1*thetad2*cos(theta1)*cos(theta4)*sin(theta2)*sin(theta3) + 0.1*thetad3*cos(theta1)*cos(theta2)*sin(theta3)*sin(theta4) + 0.1*thetad3*cos(theta1)*cos(theta3)*sin(theta2)*sin(theta4) + 0.1*thetad3*cos(theta1)*cos(theta4)*sin(theta2)*sin(theta3) - 1.76*thetad4*cos(theta2)*cos(theta3)*sin(theta2)*sin(theta3) - 0.88*thetad5*cos(theta2)*cos(theta3)*sin(theta2)*sin(theta3) - 1.76*thetad4*cos(theta2)*cos(theta4)*sin(theta2)*sin(theta4) - 0.88*thetad5*cos(theta2)*cos(theta4)*sin(theta2)*sin(theta4) - 1.76*thetad4*cos(theta3)*cos(theta4)*sin(theta3)*sin(theta4) - 0.88*thetad5*cos(theta3)*cos(theta4)*sin(theta3)*sin(theta4) + 0.7*thetad1*cos(theta2)*sin(theta1)*sin(theta3)*sin(theta4) + 0.7*thetad1*cos(theta3)*sin(theta1)*sin(theta2)*sin(theta4) + 0.7*thetad1*cos(theta4)*sin(theta1)*sin(theta2)*sin(theta3) + 0.7*thetad2*cos(theta2)*sin(theta1)*sin(theta3)*sin(theta4) + 0.7*thetad2*cos(theta3)*sin(theta1)*sin(theta2)*sin(theta4) + 0.7*thetad2*cos(theta4)*sin(theta1)*sin(theta2)*sin(theta3) + 0.7*thetad3*cos(theta2)*sin(theta1)*sin(theta3)*sin(theta4) + 0.7*thetad3*cos(theta3)*sin(theta1)*sin(theta2)*sin(theta4) + 0.7*thetad3*cos(theta4)*sin(theta1)*sin(theta2)*sin(theta3) + 6.28*thetad1*cos(theta1)^2*cos(theta2)*cos(theta3)*sin(theta4) + 6.28*thetad1*cos(theta1)^2*cos(theta2)*cos(theta4)*sin(theta3) + 6.28*thetad1*cos(theta1)^2*cos(theta3)*cos(theta4)*sin(theta2) + 6.28*thetad2*cos(theta1)^2*cos(theta2)*cos(theta3)*sin(theta4) + 6.28*thetad2*cos(theta1)^2*cos(theta2)*cos(theta4)*sin(theta3) + 6.28*thetad2*cos(theta1)^2*cos(theta3)*cos(theta4)*sin(theta2) - 2.8*thetad4*cos(theta1)*cos(theta2)*cos(theta3)^2*sin(theta2) + 6.28*thetad3*cos(theta1)^2*cos(theta2)*cos(theta3)*sin(theta4) + 6.28*thetad3*cos(theta1)^2*cos(theta2)*cos(theta4)*sin(theta3) + 6.28*thetad3*cos(theta1)^2*cos(theta3)*cos(theta4)*sin(theta2) - 2.8*thetad4*cos(theta1)*cos(theta2)*cos(theta4)^2*sin(theta2) - 2.8*thetad4*cos(theta1)*cos(theta2)^2*cos(theta3)*sin(theta3) - 1.4*thetad5*cos(theta1)*cos(theta2)*cos(theta3)^2*sin(theta2) - 1.4*thetad5*cos(theta1)*cos(theta2)*cos(theta4)^2*sin(theta2) - 1.4*thetad5*cos(theta1)*cos(theta2)^2*cos(theta3)*sin(theta3) - 2.8*thetad4*cos(theta1)*cos(theta3)*cos(theta4)^2*sin(theta3) - 2.8*thetad4*cos(theta1)*cos(theta2)^2*cos(theta4)*sin(theta4) - 2.8*thetad4*cos(theta1)*cos(theta3)^2*cos(theta4)*sin(theta4) - 1.4*thetad5*cos(theta1)*cos(theta3)*cos(theta4)^2*sin(theta3) - 1.4*thetad5*cos(theta1)*cos(theta2)^2*cos(theta4)*sin(theta4) - 1.4*thetad5*cos(theta1)*cos(theta3)^2*cos(theta4)*sin(theta4) + 7.04*thetad4*cos(theta1)^2*cos(theta2)^2*cos(theta3)^2*cos(theta4)^2 + 3.52*thetad5*cos(theta1)^2*cos(theta2)^2*cos(theta3)^2*cos(theta4)^2 + 0.4*thetad4*cos(theta2)*cos(theta3)^2*sin(theta1)*sin(theta2) + 0.4*thetad4*cos(theta2)*cos(theta4)^2*sin(theta1)*sin(theta2) + 0.4*thetad4*cos(theta2)^2*cos(theta3)*sin(theta1)*sin(theta3) + 0.2*thetad5*cos(theta2)*cos(theta3)^2*sin(theta1)*sin(theta2) + 0.2*thetad5*cos(theta2)*cos(theta4)^2*sin(theta1)*sin(theta2) + 0.2*thetad5*cos(theta2)^2*cos(theta3)*sin(theta1)*sin(theta3) + 0.4*thetad4*cos(theta3)*cos(theta4)^2*sin(theta1)*sin(theta3) + 0.4*thetad4*cos(theta2)^2*cos(theta4)*sin(theta1)*sin(theta4) + 0.4*thetad4*cos(theta3)^2*cos(theta4)*sin(theta1)*sin(theta4) + 0.2*thetad5*cos(theta3)*cos(theta4)^2*sin(theta1)*sin(theta3) + 0.2*thetad5*cos(theta2)^2*cos(theta4)*sin(theta1)*sin(theta4) + 0.2*thetad5*cos(theta3)^2*cos(theta4)*sin(theta1)*sin(theta4) - 6.28*thetad1*cos(theta1)^2*sin(theta2)*sin(theta3)*sin(theta4) - 6.28*thetad2*cos(theta1)^2*sin(theta2)*sin(theta3)*sin(theta4) - 6.28*thetad3*cos(theta1)^2*sin(theta2)*sin(theta3)*sin(theta4) + 1.76*thetad1*cos(theta1)*cos(theta2)*cos(theta3)*sin(theta1)*sin(theta4) + 1.76*thetad1*cos(theta1)*cos(theta2)*cos(theta4)*sin(theta1)*sin(theta3) + 1.76*thetad1*cos(theta1)*cos(theta3)*cos(theta4)*sin(theta1)*sin(theta2) + 1.76*thetad2*cos(theta1)*cos(theta2)*cos(theta3)*sin(theta1)*sin(theta4) + 1.76*thetad2*cos(theta1)*cos(theta2)*cos(theta4)*sin(theta1)*sin(theta3) + 1.76*thetad2*cos(theta1)*cos(theta3)*cos(theta4)*sin(theta1)*sin(theta2) + 1.76*thetad3*cos(theta1)*cos(theta2)*cos(theta3)*sin(theta1)*sin(theta4) + 1.76*thetad3*cos(theta1)*cos(theta2)*cos(theta4)*sin(theta1)*sin(theta3) + 1.76*thetad3*cos(theta1)*cos(theta3)*cos(theta4)*sin(theta1)*sin(theta2) - 25.12*thetad4*cos(theta1)*cos(theta2)^2*cos(theta3)^2*cos(theta4)^2*sin(theta1) - 12.56*thetad5*cos(theta1)*cos(theta2)^2*cos(theta3)^2*cos(theta4)^2*sin(theta1) - 1.76*thetad1*cos(theta1)*sin(theta1)*sin(theta2)*sin(theta3)*sin(theta4) - 1.76*thetad2*cos(theta1)*sin(theta1)*sin(theta2)*sin(theta3)*sin(theta4) - 1.76*thetad3*cos(theta1)*sin(theta1)*sin(theta2)*sin(theta3)*sin(theta4) + 3.52*thetad4*cos(theta1)^2*cos(theta2)*cos(theta3)*sin(theta2)*sin(theta3) + 1.76*thetad5*cos(theta1)^2*cos(theta2)*cos(theta3)*sin(theta2)*sin(theta3) + 3.52*thetad4*cos(theta1)^2*cos(theta2)*cos(theta4)*sin(theta2)*sin(theta4) + 3.52*thetad4*cos(theta2)*cos(theta3)*cos(theta4)^2*sin(theta2)*sin(theta3) + 1.76*thetad5*cos(theta1)^2*cos(theta2)*cos(theta4)*sin(theta2)*sin(theta4) + 3.52*thetad4*cos(theta2)*cos(theta3)^2*cos(theta4)*sin(theta2)*sin(theta4) + 3.52*thetad4*cos(theta1)^2*cos(theta3)*cos(theta4)*sin(theta3)*sin(theta4) + 1.76*thetad5*cos(theta2)*cos(theta3)*cos(theta4)^2*sin(theta2)*sin(theta3) + 3.52*thetad4*cos(theta2)^2*cos(theta3)*cos(theta4)*sin(theta3)*sin(theta4) + 1.76*thetad5*cos(theta2)*cos(theta3)^2*cos(theta4)*sin(theta2)*sin(theta4) + 1.76*thetad5*cos(theta1)^2*cos(theta3)*cos(theta4)*sin(theta3)*sin(theta4) + 1.76*thetad5*cos(theta2)^2*cos(theta3)*cos(theta4)*sin(theta3)*sin(theta4) + 5.6*thetad4*cos(theta1)*cos(theta2)*cos(theta3)^2*cos(theta4)^2*sin(theta2) + 5.6*thetad4*cos(theta1)*cos(theta2)^2*cos(theta3)*cos(theta4)^2*sin(theta3) + 2.8*thetad5*cos(theta1)*cos(theta2)*cos(theta3)^2*cos(theta4)^2*sin(theta2) + 5.6*thetad4*cos(theta1)*cos(theta2)^2*cos(theta3)^2*cos(theta4)*sin(theta4) + 2.8*thetad5*cos(theta1)*cos(theta2)^2*cos(theta3)*cos(theta4)^2*sin(theta3) + 2.8*thetad5*cos(theta1)*cos(theta2)^2*cos(theta3)^2*cos(theta4)*sin(theta4) - 0.8*thetad4*cos(theta2)*cos(theta3)^2*cos(theta4)^2*sin(theta1)*sin(theta2) - 0.8*thetad4*cos(theta2)^2*cos(theta3)*cos(theta4)^2*sin(theta1)*sin(theta3) - 0.4*thetad5*cos(theta2)*cos(theta3)^2*cos(theta4)^2*sin(theta1)*sin(theta2) - 0.8*thetad4*cos(theta2)^2*cos(theta3)^2*cos(theta4)*sin(theta1)*sin(theta4) - 0.4*thetad5*cos(theta2)^2*cos(theta3)*cos(theta4)^2*sin(theta1)*sin(theta3) - 0.4*thetad5*cos(theta2)^2*cos(theta3)^2*cos(theta4)*sin(theta1)*sin(theta4) - 12.56*thetad4*cos(theta1)*cos(theta2)*cos(theta3)*sin(theta1)*sin(theta2)*sin(theta3) - 6.28*thetad5*cos(theta1)*cos(theta2)*cos(theta3)*sin(theta1)*sin(theta2)*sin(theta3) - 12.56*thetad4*cos(theta1)*cos(theta2)*cos(theta4)*sin(theta1)*sin(theta2)*sin(theta4) - 6.28*thetad5*cos(theta1)*cos(theta2)*cos(theta4)*sin(theta1)*sin(theta2)*sin(theta4) - 12.56*thetad4*cos(theta1)*cos(theta3)*cos(theta4)*sin(theta1)*sin(theta3)*sin(theta4) - 6.28*thetad5*cos(theta1)*cos(theta3)*cos(theta4)*sin(theta1)*sin(theta3)*sin(theta4) - 7.04*thetad4*cos(theta1)^2*cos(theta2)*cos(theta3)*cos(theta4)^2*sin(theta2)*sin(theta3) - 7.04*thetad4*cos(theta1)^2*cos(theta2)*cos(theta3)^2*cos(theta4)*sin(theta2)*sin(theta4) - 3.52*thetad5*cos(theta1)^2*cos(theta2)*cos(theta3)*cos(theta4)^2*sin(theta2)*sin(theta3) - 7.04*thetad4*cos(theta1)^2*cos(theta2)^2*cos(theta3)*cos(theta4)*sin(theta3)*sin(theta4) - 3.52*thetad5*cos(theta1)^2*cos(theta2)*cos(theta3)^2*cos(theta4)*sin(theta2)*sin(theta4) - 3.52*thetad5*cos(theta1)^2*cos(theta2)^2*cos(theta3)*cos(theta4)*sin(theta3)*sin(theta4) + 25.12*thetad4*cos(theta1)*cos(theta2)*cos(theta3)*cos(theta4)^2*sin(theta1)*sin(theta2)*sin(theta3) + 25.12*thetad4*cos(theta1)*cos(theta2)*cos(theta3)^2*cos(theta4)*sin(theta1)*sin(theta2)*sin(theta4) + 12.56*thetad5*cos(theta1)*cos(theta2)*cos(theta3)*cos(theta4)^2*sin(theta1)*sin(theta2)*sin(theta3) + 25.12*thetad4*cos(theta1)*cos(theta2)^2*cos(theta3)*cos(theta4)*sin(theta1)*sin(theta3)*sin(theta4) + 12.56*thetad5*cos(theta1)*cos(theta2)*cos(theta3)^2*cos(theta4)*sin(theta1)*sin(theta2)*sin(theta4) + 12.56*thetad5*cos(theta1)*cos(theta2)^2*cos(theta3)*cos(theta4)*sin(theta1)*sin(theta3)*sin(theta4) - 5.6*thetad4*cos(theta1)*cos(theta2)*cos(theta3)*cos(theta4)*sin(theta2)*sin(theta3)*sin(theta4) - 2.8*thetad5*cos(theta1)*cos(theta2)*cos(theta3)*cos(theta4)*sin(theta2)*sin(theta3)*sin(theta4) + 0.8*thetad4*cos(theta2)*cos(theta3)*cos(theta4)*sin(theta1)*sin(theta2)*sin(theta3)*sin(theta4) + 0.4*thetad5*cos(theta2)*cos(theta3)*cos(theta4)*sin(theta1)*sin(theta2)*sin(theta3)*sin(theta4) ;
C(1,5) = 0.44*thetad4 + 0.44*thetad5 - 0.88*thetad4*cos(theta1)^2 - 0.44*thetad4*cos(theta2)^2 - 0.88*thetad5*cos(theta1)^2 - 0.44*thetad4*cos(theta3)^2 - 0.44*thetad5*cos(theta2)^2 - 0.44*thetad4*cos(theta4)^2 - 0.44*thetad5*cos(theta3)^2 - 0.44*thetad5*cos(theta4)^2 + 0.88*thetad4*cos(theta1)^2*cos(theta2)^2 + 0.88*thetad4*cos(theta1)^2*cos(theta3)^2 + 0.88*thetad5*cos(theta1)^2*cos(theta2)^2 + 0.88*thetad4*cos(theta1)^2*cos(theta4)^2 + 0.88*thetad4*cos(theta2)^2*cos(theta3)^2 + 0.88*thetad5*cos(theta1)^2*cos(theta3)^2 + 0.88*thetad4*cos(theta2)^2*cos(theta4)^2 + 0.88*thetad5*cos(theta1)^2*cos(theta4)^2 + 0.88*thetad5*cos(theta2)^2*cos(theta3)^2 + 0.88*thetad4*cos(theta3)^2*cos(theta4)^2 + 0.88*thetad5*cos(theta2)^2*cos(theta4)^2 + 0.88*thetad5*cos(theta3)^2*cos(theta4)^2 + 3.14*thetad4*cos(theta1)*sin(theta1) + 3.14*thetad5*cos(theta1)*sin(theta1) + 0.7*thetad4*cos(theta1)*cos(theta2)*sin(theta2) - 1.57*thetad1*cos(theta2)*cos(theta3)*sin(theta4) - 1.57*thetad1*cos(theta2)*cos(theta4)*sin(theta3) - 1.57*thetad1*cos(theta3)*cos(theta4)*sin(theta2) + 0.7*thetad5*cos(theta1)*cos(theta2)*sin(theta2) - 1.57*thetad2*cos(theta2)*cos(theta3)*sin(theta4) - 1.57*thetad2*cos(theta2)*cos(theta4)*sin(theta3) - 1.57*thetad2*cos(theta3)*cos(theta4)*sin(theta2) + 0.7*thetad4*cos(theta1)*cos(theta3)*sin(theta3) - 1.57*thetad3*cos(theta2)*cos(theta3)*sin(theta4) - 1.57*thetad3*cos(theta2)*cos(theta4)*sin(theta3) - 1.57*thetad3*cos(theta3)*cos(theta4)*sin(theta2) + 0.7*thetad5*cos(theta1)*cos(theta3)*sin(theta3) + 0.7*thetad4*cos(theta1)*cos(theta4)*sin(theta4) + 0.7*thetad5*cos(theta1)*cos(theta4)*sin(theta4) - 1.76*thetad4*cos(theta1)^2*cos(theta2)^2*cos(theta3)^2 - 1.76*thetad4*cos(theta1)^2*cos(theta2)^2*cos(theta4)^2 - 1.76*thetad5*cos(theta1)^2*cos(theta2)^2*cos(theta3)^2 - 1.76*thetad4*cos(theta1)^2*cos(theta3)^2*cos(theta4)^2 - 1.76*thetad5*cos(theta1)^2*cos(theta2)^2*cos(theta4)^2 - 1.76*thetad4*cos(theta2)^2*cos(theta3)^2*cos(theta4)^2 - 1.76*thetad5*cos(theta1)^2*cos(theta3)^2*cos(theta4)^2 - 1.76*thetad5*cos(theta2)^2*cos(theta3)^2*cos(theta4)^2 - 0.1*thetad4*cos(theta2)*sin(theta1)*sin(theta2) - 0.1*thetad5*cos(theta2)*sin(theta1)*sin(theta2) - 0.1*thetad4*cos(theta3)*sin(theta1)*sin(theta3) - 0.1*thetad5*cos(theta3)*sin(theta1)*sin(theta3) - 0.1*thetad4*cos(theta4)*sin(theta1)*sin(theta4) - 0.1*thetad5*cos(theta4)*sin(theta1)*sin(theta4) + 1.57*thetad1*sin(theta2)*sin(theta3)*sin(theta4) + 1.57*thetad2*sin(theta2)*sin(theta3)*sin(theta4) + 1.57*thetad3*sin(theta2)*sin(theta3)*sin(theta4) - 3.14*thetad4*cos(theta1)*cos(theta2)^2*sin(theta1) - 3.14*thetad4*cos(theta1)*cos(theta3)^2*sin(theta1) - 3.14*thetad5*cos(theta1)*cos(theta2)^2*sin(theta1) - 3.14*thetad4*cos(theta1)*cos(theta4)^2*sin(theta1) - 3.14*thetad5*cos(theta1)*cos(theta3)^2*sin(theta1) - 3.14*thetad5*cos(theta1)*cos(theta4)^2*sin(theta1) + 6.28*thetad4*cos(theta1)*cos(theta2)^2*cos(theta3)^2*sin(theta1) + 6.28*thetad4*cos(theta1)*cos(theta2)^2*cos(theta4)^2*sin(theta1) + 6.28*thetad5*cos(theta1)*cos(theta2)^2*cos(theta3)^2*sin(theta1) + 6.28*thetad4*cos(theta1)*cos(theta3)^2*cos(theta4)^2*sin(theta1) + 6.28*thetad5*cos(theta1)*cos(theta2)^2*cos(theta4)^2*sin(theta1) + 6.28*thetad5*cos(theta1)*cos(theta3)^2*cos(theta4)^2*sin(theta1) - 0.05*thetad1*cos(theta1)*cos(theta2)*cos(theta3)*cos(theta4) - 0.05*thetad2*cos(theta1)*cos(theta2)*cos(theta3)*cos(theta4) - 0.05*thetad3*cos(theta1)*cos(theta2)*cos(theta3)*cos(theta4) - 0.35*thetad1*cos(theta2)*cos(theta3)*cos(theta4)*sin(theta1) - 0.35*thetad2*cos(theta2)*cos(theta3)*cos(theta4)*sin(theta1) - 0.35*thetad3*cos(theta2)*cos(theta3)*cos(theta4)*sin(theta1) + 0.05*thetad1*cos(theta1)*cos(theta2)*sin(theta3)*sin(theta4) + 0.05*thetad1*cos(theta1)*cos(theta3)*sin(theta2)*sin(theta4) + 0.05*thetad1*cos(theta1)*cos(theta4)*sin(theta2)*sin(theta3) + 0.05*thetad2*cos(theta1)*cos(theta2)*sin(theta3)*sin(theta4) + 0.05*thetad2*cos(theta1)*cos(theta3)*sin(theta2)*sin(theta4) + 0.05*thetad2*cos(theta1)*cos(theta4)*sin(theta2)*sin(theta3) + 0.05*thetad3*cos(theta1)*cos(theta2)*sin(theta3)*sin(theta4) + 0.05*thetad3*cos(theta1)*cos(theta3)*sin(theta2)*sin(theta4) + 0.05*thetad3*cos(theta1)*cos(theta4)*sin(theta2)*sin(theta3) - 0.88*thetad4*cos(theta2)*cos(theta3)*sin(theta2)*sin(theta3) - 0.88*thetad5*cos(theta2)*cos(theta3)*sin(theta2)*sin(theta3) - 0.88*thetad4*cos(theta2)*cos(theta4)*sin(theta2)*sin(theta4) - 0.88*thetad5*cos(theta2)*cos(theta4)*sin(theta2)*sin(theta4) - 0.88*thetad4*cos(theta3)*cos(theta4)*sin(theta3)*sin(theta4) - 0.88*thetad5*cos(theta3)*cos(theta4)*sin(theta3)*sin(theta4) + 0.35*thetad1*cos(theta2)*sin(theta1)*sin(theta3)*sin(theta4) + 0.35*thetad1*cos(theta3)*sin(theta1)*sin(theta2)*sin(theta4) + 0.35*thetad1*cos(theta4)*sin(theta1)*sin(theta2)*sin(theta3) + 0.35*thetad2*cos(theta2)*sin(theta1)*sin(theta3)*sin(theta4) + 0.35*thetad2*cos(theta3)*sin(theta1)*sin(theta2)*sin(theta4) + 0.35*thetad2*cos(theta4)*sin(theta1)*sin(theta2)*sin(theta3) + 0.35*thetad3*cos(theta2)*sin(theta1)*sin(theta3)*sin(theta4) + 0.35*thetad3*cos(theta3)*sin(theta1)*sin(theta2)*sin(theta4) + 0.35*thetad3*cos(theta4)*sin(theta1)*sin(theta2)*sin(theta3) + 3.14*thetad1*cos(theta1)^2*cos(theta2)*cos(theta3)*sin(theta4) + 3.14*thetad1*cos(theta1)^2*cos(theta2)*cos(theta4)*sin(theta3) + 3.14*thetad1*cos(theta1)^2*cos(theta3)*cos(theta4)*sin(theta2) + 3.14*thetad2*cos(theta1)^2*cos(theta2)*cos(theta3)*sin(theta4) + 3.14*thetad2*cos(theta1)^2*cos(theta2)*cos(theta4)*sin(theta3) + 3.14*thetad2*cos(theta1)^2*cos(theta3)*cos(theta4)*sin(theta2) - 1.4*thetad4*cos(theta1)*cos(theta2)*cos(theta3)^2*sin(theta2) + 3.14*thetad3*cos(theta1)^2*cos(theta2)*cos(theta3)*sin(theta4) + 3.14*thetad3*cos(theta1)^2*cos(theta2)*cos(theta4)*sin(theta3) + 3.14*thetad3*cos(theta1)^2*cos(theta3)*cos(theta4)*sin(theta2) - 1.4*thetad4*cos(theta1)*cos(theta2)*cos(theta4)^2*sin(theta2) - 1.4*thetad4*cos(theta1)*cos(theta2)^2*cos(theta3)*sin(theta3) - 1.4*thetad5*cos(theta1)*cos(theta2)*cos(theta3)^2*sin(theta2) - 1.4*thetad5*cos(theta1)*cos(theta2)*cos(theta4)^2*sin(theta2) - 1.4*thetad5*cos(theta1)*cos(theta2)^2*cos(theta3)*sin(theta3) - 1.4*thetad4*cos(theta1)*cos(theta3)*cos(theta4)^2*sin(theta3) - 1.4*thetad4*cos(theta1)*cos(theta2)^2*cos(theta4)*sin(theta4) - 1.4*thetad4*cos(theta1)*cos(theta3)^2*cos(theta4)*sin(theta4) - 1.4*thetad5*cos(theta1)*cos(theta3)*cos(theta4)^2*sin(theta3) - 1.4*thetad5*cos(theta1)*cos(theta2)^2*cos(theta4)*sin(theta4) - 1.4*thetad5*cos(theta1)*cos(theta3)^2*cos(theta4)*sin(theta4) + 3.52*thetad4*cos(theta1)^2*cos(theta2)^2*cos(theta3)^2*cos(theta4)^2 + 3.52*thetad5*cos(theta1)^2*cos(theta2)^2*cos(theta3)^2*cos(theta4)^2 + 0.2*thetad4*cos(theta2)*cos(theta3)^2*sin(theta1)*sin(theta2) + 0.2*thetad4*cos(theta2)*cos(theta4)^2*sin(theta1)*sin(theta2) + 0.2*thetad4*cos(theta2)^2*cos(theta3)*sin(theta1)*sin(theta3) + 0.2*thetad5*cos(theta2)*cos(theta3)^2*sin(theta1)*sin(theta2) + 0.2*thetad5*cos(theta2)*cos(theta4)^2*sin(theta1)*sin(theta2) + 0.2*thetad5*cos(theta2)^2*cos(theta3)*sin(theta1)*sin(theta3) + 0.2*thetad4*cos(theta3)*cos(theta4)^2*sin(theta1)*sin(theta3) + 0.2*thetad4*cos(theta2)^2*cos(theta4)*sin(theta1)*sin(theta4) + 0.2*thetad4*cos(theta3)^2*cos(theta4)*sin(theta1)*sin(theta4) + 0.2*thetad5*cos(theta3)*cos(theta4)^2*sin(theta1)*sin(theta3) + 0.2*thetad5*cos(theta2)^2*cos(theta4)*sin(theta1)*sin(theta4) + 0.2*thetad5*cos(theta3)^2*cos(theta4)*sin(theta1)*sin(theta4) - 3.14*thetad1*cos(theta1)^2*sin(theta2)*sin(theta3)*sin(theta4) - 3.14*thetad2*cos(theta1)^2*sin(theta2)*sin(theta3)*sin(theta4) - 3.14*thetad3*cos(theta1)^2*sin(theta2)*sin(theta3)*sin(theta4) + 0.88*thetad1*cos(theta1)*cos(theta2)*cos(theta3)*sin(theta1)*sin(theta4) + 0.88*thetad1*cos(theta1)*cos(theta2)*cos(theta4)*sin(theta1)*sin(theta3) + 0.88*thetad1*cos(theta1)*cos(theta3)*cos(theta4)*sin(theta1)*sin(theta2) + 0.88*thetad2*cos(theta1)*cos(theta2)*cos(theta3)*sin(theta1)*sin(theta4) + 0.88*thetad2*cos(theta1)*cos(theta2)*cos(theta4)*sin(theta1)*sin(theta3) + 0.88*thetad2*cos(theta1)*cos(theta3)*cos(theta4)*sin(theta1)*sin(theta2) + 0.88*thetad3*cos(theta1)*cos(theta2)*cos(theta3)*sin(theta1)*sin(theta4) + 0.88*thetad3*cos(theta1)*cos(theta2)*cos(theta4)*sin(theta1)*sin(theta3) + 0.88*thetad3*cos(theta1)*cos(theta3)*cos(theta4)*sin(theta1)*sin(theta2) - 12.56*thetad4*cos(theta1)*cos(theta2)^2*cos(theta3)^2*cos(theta4)^2*sin(theta1) - 12.56*thetad5*cos(theta1)*cos(theta2)^2*cos(theta3)^2*cos(theta4)^2*sin(theta1) - 0.88*thetad1*cos(theta1)*sin(theta1)*sin(theta2)*sin(theta3)*sin(theta4) - 0.88*thetad2*cos(theta1)*sin(theta1)*sin(theta2)*sin(theta3)*sin(theta4) - 0.88*thetad3*cos(theta1)*sin(theta1)*sin(theta2)*sin(theta3)*sin(theta4) + 1.76*thetad4*cos(theta1)^2*cos(theta2)*cos(theta3)*sin(theta2)*sin(theta3) + 1.76*thetad5*cos(theta1)^2*cos(theta2)*cos(theta3)*sin(theta2)*sin(theta3) + 1.76*thetad4*cos(theta1)^2*cos(theta2)*cos(theta4)*sin(theta2)*sin(theta4) + 1.76*thetad4*cos(theta2)*cos(theta3)*cos(theta4)^2*sin(theta2)*sin(theta3) + 1.76*thetad5*cos(theta1)^2*cos(theta2)*cos(theta4)*sin(theta2)*sin(theta4) + 1.76*thetad4*cos(theta2)*cos(theta3)^2*cos(theta4)*sin(theta2)*sin(theta4) + 1.76*thetad4*cos(theta1)^2*cos(theta3)*cos(theta4)*sin(theta3)*sin(theta4) + 1.76*thetad5*cos(theta2)*cos(theta3)*cos(theta4)^2*sin(theta2)*sin(theta3) + 1.76*thetad4*cos(theta2)^2*cos(theta3)*cos(theta4)*sin(theta3)*sin(theta4) + 1.76*thetad5*cos(theta2)*cos(theta3)^2*cos(theta4)*sin(theta2)*sin(theta4) + 1.76*thetad5*cos(theta1)^2*cos(theta3)*cos(theta4)*sin(theta3)*sin(theta4) + 1.76*thetad5*cos(theta2)^2*cos(theta3)*cos(theta4)*sin(theta3)*sin(theta4) + 2.8*thetad4*cos(theta1)*cos(theta2)*cos(theta3)^2*cos(theta4)^2*sin(theta2) + 2.8*thetad4*cos(theta1)*cos(theta2)^2*cos(theta3)*cos(theta4)^2*sin(theta3) + 2.8*thetad5*cos(theta1)*cos(theta2)*cos(theta3)^2*cos(theta4)^2*sin(theta2) + 2.8*thetad4*cos(theta1)*cos(theta2)^2*cos(theta3)^2*cos(theta4)*sin(theta4) + 2.8*thetad5*cos(theta1)*cos(theta2)^2*cos(theta3)*cos(theta4)^2*sin(theta3) + 2.8*thetad5*cos(theta1)*cos(theta2)^2*cos(theta3)^2*cos(theta4)*sin(theta4) - 0.4*thetad4*cos(theta2)*cos(theta3)^2*cos(theta4)^2*sin(theta1)*sin(theta2) - 0.4*thetad4*cos(theta2)^2*cos(theta3)*cos(theta4)^2*sin(theta1)*sin(theta3) - 0.4*thetad5*cos(theta2)*cos(theta3)^2*cos(theta4)^2*sin(theta1)*sin(theta2) - 0.4*thetad4*cos(theta2)^2*cos(theta3)^2*cos(theta4)*sin(theta1)*sin(theta4) - 0.4*thetad5*cos(theta2)^2*cos(theta3)*cos(theta4)^2*sin(theta1)*sin(theta3) - 0.4*thetad5*cos(theta2)^2*cos(theta3)^2*cos(theta4)*sin(theta1)*sin(theta4) - 6.28*thetad4*cos(theta1)*cos(theta2)*cos(theta3)*sin(theta1)*sin(theta2)*sin(theta3) - 6.28*thetad5*cos(theta1)*cos(theta2)*cos(theta3)*sin(theta1)*sin(theta2)*sin(theta3) - 6.28*thetad4*cos(theta1)*cos(theta2)*cos(theta4)*sin(theta1)*sin(theta2)*sin(theta4) - 6.28*thetad5*cos(theta1)*cos(theta2)*cos(theta4)*sin(theta1)*sin(theta2)*sin(theta4) - 6.28*thetad4*cos(theta1)*cos(theta3)*cos(theta4)*sin(theta1)*sin(theta3)*sin(theta4) - 6.28*thetad5*cos(theta1)*cos(theta3)*cos(theta4)*sin(theta1)*sin(theta3)*sin(theta4) - 3.52*thetad4*cos(theta1)^2*cos(theta2)*cos(theta3)*cos(theta4)^2*sin(theta2)*sin(theta3) - 3.52*thetad4*cos(theta1)^2*cos(theta2)*cos(theta3)^2*cos(theta4)*sin(theta2)*sin(theta4) - 3.52*thetad5*cos(theta1)^2*cos(theta2)*cos(theta3)*cos(theta4)^2*sin(theta2)*sin(theta3) - 3.52*thetad4*cos(theta1)^2*cos(theta2)^2*cos(theta3)*cos(theta4)*sin(theta3)*sin(theta4) - 3.52*thetad5*cos(theta1)^2*cos(theta2)*cos(theta3)^2*cos(theta4)*sin(theta2)*sin(theta4) - 3.52*thetad5*cos(theta1)^2*cos(theta2)^2*cos(theta3)*cos(theta4)*sin(theta3)*sin(theta4) + 12.56*thetad4*cos(theta1)*cos(theta2)*cos(theta3)*cos(theta4)^2*sin(theta1)*sin(theta2)*sin(theta3) + 12.56*thetad4*cos(theta1)*cos(theta2)*cos(theta3)^2*cos(theta4)*sin(theta1)*sin(theta2)*sin(theta4) + 12.56*thetad5*cos(theta1)*cos(theta2)*cos(theta3)*cos(theta4)^2*sin(theta1)*sin(theta2)*sin(theta3) + 12.56*thetad4*cos(theta1)*cos(theta2)^2*cos(theta3)*cos(theta4)*sin(theta1)*sin(theta3)*sin(theta4) + 12.56*thetad5*cos(theta1)*cos(theta2)*cos(theta3)^2*cos(theta4)*sin(theta1)*sin(theta2)*sin(theta4) + 12.56*thetad5*cos(theta1)*cos(theta2)^2*cos(theta3)*cos(theta4)*sin(theta1)*sin(theta3)*sin(theta4) - 2.8*thetad4*cos(theta1)*cos(theta2)*cos(theta3)*cos(theta4)*sin(theta2)*sin(theta3)*sin(theta4) - 2.8*thetad5*cos(theta1)*cos(theta2)*cos(theta3)*cos(theta4)*sin(theta2)*sin(theta3)*sin(theta4) + 0.4*thetad4*cos(theta2)*cos(theta3)*cos(theta4)*sin(theta1)*sin(theta2)*sin(theta3)*sin(theta4) + 0.4*thetad5*cos(theta2)*cos(theta3)*cos(theta4)*sin(theta1)*sin(theta2)*sin(theta3)*sin(theta4) ;
C(2,1) = 0.095452*thetad1 - 0.190904*thetad1*cos(theta2)^2 - 0.734216*thetad1*cos(theta3)^2 + 0.206584*thetad1*cos(theta4)^2 - 0.3136*thetad1*cos(theta3) - 0.441816*thetad2*cos(theta2) + 0.4018*thetad1*cos(theta4) - 0.0196*thetad1*cos(theta5) - 0.87*thetad1*sin(theta3) - 0.053508*thetad2*sin(theta2) + 0.1666*thetad1*sin(theta4) + 0.098*thetad1*sin(theta5) + 1.468432*thetad1*cos(theta2)^2*cos(theta3)^2 - 0.413168*thetad1*cos(theta2)^2*cos(theta4)^2 - 0.413168*thetad1*cos(theta3)^2*cos(theta4)^2 - 0.4875*thetad2*cos(theta2)*cos(theta3) - 0.4018*thetad1*cos(theta3)*cos(theta4) - 0.4875*thetad3*cos(theta2)*cos(theta3) - 0.07*thetad2*cos(theta2)*cos(theta5) + 0.60836*thetad1*cos(theta2)*sin(theta2) - 0.435656*thetad1*cos(theta3)*sin(theta3) - 0.150528*thetad2*cos(theta2)*sin(theta3) - 0.150528*thetad2*cos(theta3)*sin(theta2) - 0.1666*thetad1*cos(theta3)*sin(theta4) - 0.1666*thetad1*cos(theta4)*sin(theta3) - 0.150528*thetad3*cos(theta2)*sin(theta3) - 0.150528*thetad3*cos(theta3)*sin(theta2) - 0.060312*thetad1*cos(theta4)*sin(theta4) - 0.014*thetad2*cos(theta2)*sin(theta5) + 0.028*thetad1*cos(theta5)*sin(theta4) + 0.014*thetad5*cos(theta5)*sin(theta2) + 0.4875*thetad2*sin(theta2)*sin(theta3) + 0.4018*thetad1*sin(theta3)*sin(theta4) + 0.4875*thetad3*sin(theta2)*sin(theta3) - 0.14*thetad1*sin(theta4)*sin(theta5) - 0.07*thetad5*sin(theta2)*sin(theta5) + 0.6272*thetad1*cos(theta2)^2*cos(theta3) - 0.8036*thetad1*cos(theta2)^2*cos(theta4) + 0.0392*thetad1*cos(theta2)^2*cos(theta5) - 0.8036*thetad1*cos(theta3)^2*cos(theta4) + 0.0392*thetad1*cos(theta3)^2*cos(theta5) + 0.0392*thetad1*cos(theta4)^2*cos(theta5) + 1.74*thetad1*cos(theta2)^2*sin(theta3) - 0.3332*thetad1*cos(theta2)^2*sin(theta4) - 0.196*thetad1*cos(theta2)^2*sin(theta5) - 0.3332*thetad1*cos(theta3)^2*sin(theta4) - 0.196*thetad1*cos(theta3)^2*sin(theta5) - 0.196*thetad1*cos(theta4)^2*sin(theta5) + 1.6072*thetad1*cos(theta2)^2*cos(theta3)^2*cos(theta4) - 0.0784*thetad1*cos(theta2)^2*cos(theta3)^2*cos(theta5) - 0.0784*thetad1*cos(theta2)^2*cos(theta4)^2*cos(theta5) - 0.0784*thetad1*cos(theta3)^2*cos(theta4)^2*cos(theta5) + 0.6664*thetad1*cos(theta2)^2*cos(theta3)^2*sin(theta4) + 0.392*thetad1*cos(theta2)^2*cos(theta3)^2*sin(theta5) + 0.392*thetad1*cos(theta2)^2*cos(theta4)^2*sin(theta5) + 0.392*thetad1*cos(theta3)^2*cos(theta4)^2*sin(theta5) - 0.190918*thetad2*cos(theta2)*cos(theta3)*cos(theta4) - 0.07*thetad2*cos(theta2)*cos(theta3)*cos(theta5) - 0.190918*thetad3*cos(theta2)*cos(theta3)*cos(theta4) - 0.07*thetad3*cos(theta2)*cos(theta3)*cos(theta5) + 0.249082*thetad4*cos(theta2)*cos(theta3)*cos(theta4) + 0.22*thetad5*cos(theta2)*cos(theta3)*cos(theta4) + 1.74*thetad1*cos(theta2)*cos(theta3)*sin(theta2) - 0.3332*thetad1*cos(theta2)*cos(theta4)*sin(theta2) - 0.3332*thetad1*cos(theta3)*cos(theta4)*sin(theta3) + 0.373674*thetad2*cos(theta2)*cos(theta3)*sin(theta4) + 0.373674*thetad2*cos(theta2)*cos(theta4)*sin(theta3) + 0.373674*thetad2*cos(theta3)*cos(theta4)*sin(theta2) - 0.014*thetad2*cos(theta2)*cos(theta3)*sin(theta5) + 0.373674*thetad3*cos(theta2)*cos(theta3)*sin(theta4) + 0.373674*thetad3*cos(theta2)*cos(theta4)*sin(theta3) + 0.373674*thetad3*cos(theta3)*cos(theta4)*sin(theta2) - 0.028*thetad1*cos(theta3)*cos(theta5)*sin(theta4) - 0.028*thetad1*cos(theta4)*cos(theta5)*sin(theta3) - 0.014*thetad3*cos(theta2)*cos(theta3)*sin(theta5) + 0.373674*thetad4*cos(theta2)*cos(theta3)*sin(theta4) + 0.373674*thetad4*cos(theta2)*cos(theta4)*sin(theta3) + 0.373674*thetad4*cos(theta3)*cos(theta4)*sin(theta2) + 0.0728*thetad5*cos(theta2)*cos(theta3)*sin(theta4) + 0.0728*thetad5*cos(theta2)*cos(theta4)*sin(theta3) + 0.0728*thetad5*cos(theta3)*cos(theta4)*sin(theta2) + 0.014*thetad5*cos(theta2)*cos(theta5)*sin(theta3) + 0.014*thetad5*cos(theta3)*cos(theta5)*sin(theta2) + 0.826336*thetad1*cos(theta2)^2*cos(theta3)^2*cos(theta4)^2 - 0.6272*thetad1*cos(theta2)*sin(theta2)*sin(theta3) + 0.8036*thetad1*cos(theta2)*sin(theta2)*sin(theta4) + 0.8036*thetad1*cos(theta3)*sin(theta3)*sin(theta4) + 0.190918*thetad2*cos(theta2)*sin(theta3)*sin(theta4) + 0.190918*thetad2*cos(theta3)*sin(theta2)*sin(theta4) + 0.190918*thetad2*cos(theta4)*sin(theta2)*sin(theta3) + 0.07*thetad2*cos(theta5)*sin(theta2)*sin(theta3) + 0.190918*thetad3*cos(theta2)*sin(theta3)*sin(theta4) + 0.190918*thetad3*cos(theta3)*sin(theta2)*sin(theta4) + 0.190918*thetad3*cos(theta4)*sin(theta2)*sin(theta3) + 0.14*thetad1*cos(theta3)*sin(theta4)*sin(theta5) + 0.14*thetad1*cos(theta4)*sin(theta3)*sin(theta5) + 0.07*thetad3*cos(theta5)*sin(theta2)*sin(theta3) - 0.249082*thetad4*cos(theta2)*sin(theta3)*sin(theta4) - 0.249082*thetad4*cos(theta3)*sin(theta2)*sin(theta4) - 0.249082*thetad4*cos(theta4)*sin(theta2)*sin(theta3) - 0.22*thetad5*cos(theta2)*sin(theta3)*sin(theta4) - 0.22*thetad5*cos(theta3)*sin(theta2)*sin(theta4) - 0.22*thetad5*cos(theta4)*sin(theta2)*sin(theta3) - 0.07*thetad5*cos(theta2)*sin(theta3)*sin(theta5) - 0.07*thetad5*cos(theta3)*sin(theta2)*sin(theta5) - 0.373674*thetad2*sin(theta2)*sin(theta3)*sin(theta4) + 0.014*thetad2*sin(theta2)*sin(theta3)*sin(theta5) - 0.373674*thetad3*sin(theta2)*sin(theta3)*sin(theta4) + 0.014*thetad3*sin(theta2)*sin(theta3)*sin(theta5) - 0.373674*thetad4*sin(theta2)*sin(theta3)*sin(theta4) - 0.0728*thetad5*sin(theta2)*sin(theta3)*sin(theta4) + 0.8036*thetad1*cos(theta2)^2*cos(theta3)*cos(theta4) + 0.871312*thetad1*cos(theta2)*cos(theta3)^2*sin(theta2) + 0.120624*thetad1*cos(theta2)*cos(theta4)^2*sin(theta2) + 0.871312*thetad1*cos(theta2)^2*cos(theta3)*sin(theta3) - 0.1344*thetad1*cos(theta2)*cos(theta5)^2*sin(theta2) + 0.3332*thetad1*cos(theta2)^2*cos(theta3)*sin(theta4) + 0.3332*thetad1*cos(theta2)^2*cos(theta4)*sin(theta3) + 0.120624*thetad1*cos(theta3)*cos(theta4)^2*sin(theta3) + 0.120624*thetad1*cos(theta2)^2*cos(theta4)*sin(theta4) - 0.1344*thetad1*cos(theta3)*cos(theta5)^2*sin(theta3) - 0.056*thetad1*cos(theta2)^2*cos(theta5)*sin(theta4) + 0.120624*thetad1*cos(theta3)^2*cos(theta4)*sin(theta4) - 0.056*thetad1*cos(theta3)^2*cos(theta5)*sin(theta4) - 0.1344*thetad1*cos(theta4)*cos(theta5)^2*sin(theta4) - 0.8036*thetad1*cos(theta2)^2*sin(theta3)*sin(theta4) + 0.28*thetad1*cos(theta2)^2*sin(theta4)*sin(theta5) + 0.28*thetad1*cos(theta3)^2*sin(theta4)*sin(theta5) - 0.241248*thetad1*cos(theta2)*cos(theta3)^2*cos(theta4)^2*sin(theta2) + 0.2688*thetad1*cos(theta2)*cos(theta3)^2*cos(theta5)^2*sin(theta2) - 0.241248*thetad1*cos(theta2)^2*cos(theta3)*cos(theta4)^2*sin(theta3) + 0.2688*thetad1*cos(theta2)*cos(theta4)^2*cos(theta5)^2*sin(theta2) + 0.2688*thetad1*cos(theta2)^2*cos(theta3)*cos(theta5)^2*sin(theta3) - 0.241248*thetad1*cos(theta2)^2*cos(theta3)^2*cos(theta4)*sin(theta4) + 0.112*thetad1*cos(theta2)^2*cos(theta3)^2*cos(theta5)*sin(theta4) + 0.2688*thetad1*cos(theta3)*cos(theta4)^2*cos(theta5)^2*sin(theta3) + 0.2688*thetad1*cos(theta2)^2*cos(theta4)*cos(theta5)^2*sin(theta4) + 0.2688*thetad1*cos(theta3)^2*cos(theta4)*cos(theta5)^2*sin(theta4) - 0.56*thetad1*cos(theta2)^2*cos(theta3)^2*sin(theta4)*sin(theta5) + 0.0098*thetad5*cos(theta2)*cos(theta3)*cos(theta4)*cos(theta5) + 0.3332*thetad1*cos(theta2)*cos(theta3)*cos(theta4)*sin(theta2) - 0.056*thetad1*cos(theta2)*cos(theta4)*cos(theta5)*sin(theta2) - 0.7*thetad4*cos(theta1)*cos(theta2)*cos(theta3)*sin(theta4) - 0.7*thetad4*cos(theta1)*cos(theta2)*cos(theta4)*sin(theta3) - 0.7*thetad4*cos(theta1)*cos(theta3)*cos(theta4)*sin(theta2) - 0.35*thetad5*cos(theta1)*cos(theta2)*cos(theta3)*sin(theta4) - 0.35*thetad5*cos(theta1)*cos(theta2)*cos(theta4)*sin(theta3) - 0.35*thetad5*cos(theta1)*cos(theta3)*cos(theta4)*sin(theta2) - 0.056*thetad1*cos(theta3)*cos(theta4)*cos(theta5)*sin(theta3) + 0.049*thetad2*cos(theta2)*cos(theta3)*cos(theta5)*sin(theta4) + 0.049*thetad2*cos(theta2)*cos(theta4)*cos(theta5)*sin(theta3) + 0.049*thetad2*cos(theta3)*cos(theta4)*cos(theta5)*sin(theta2) + 0.049*thetad3*cos(theta2)*cos(theta3)*cos(theta5)*sin(theta4) + 0.049*thetad3*cos(theta2)*cos(theta4)*cos(theta5)*sin(theta3) + 0.049*thetad3*cos(theta3)*cos(theta4)*cos(theta5)*sin(theta2) + 0.049*thetad4*cos(theta2)*cos(theta3)*cos(theta5)*sin(theta4) + 0.049*thetad4*cos(theta2)*cos(theta4)*cos(theta5)*sin(theta3) + 0.049*thetad4*cos(theta3)*cos(theta4)*cos(theta5)*sin(theta2) - 0.049*thetad5*cos(theta2)*cos(theta3)*cos(theta4)*sin(theta5) + 0.1568*thetad1*cos(theta2)^2*cos(theta3)^2*cos(theta4)^2*cos(theta5) - 1.468432*thetad1*cos(theta2)*cos(theta3)*sin(theta2)*sin(theta3) - 0.8036*thetad1*cos(theta2)*cos(theta3)*sin(theta2)*sin(theta4) - 0.8036*thetad1*cos(theta2)*cos(theta4)*sin(theta2)*sin(theta3) + 0.413168*thetad1*cos(theta2)*cos(theta4)*sin(theta2)*sin(theta4) + 0.28*thetad1*cos(theta2)*cos(theta4)*sin(theta2)*sin(theta5) + 0.1*thetad4*cos(theta2)*cos(theta3)*sin(theta1)*sin(theta4) + 0.1*thetad4*cos(theta2)*cos(theta4)*sin(theta1)*sin(theta3) + 0.1*thetad4*cos(theta3)*cos(theta4)*sin(theta1)*sin(theta2) - 0.056*thetad1*cos(theta2)*cos(theta5)*sin(theta2)*sin(theta5) + 0.413168*thetad1*cos(theta3)*cos(theta4)*sin(theta3)*sin(theta4) + 0.05*thetad5*cos(theta2)*cos(theta3)*sin(theta1)*sin(theta4) + 0.05*thetad5*cos(theta2)*cos(theta4)*sin(theta1)*sin(theta3) + 0.05*thetad5*cos(theta3)*cos(theta4)*sin(theta1)*sin(theta2) + 0.28*thetad1*cos(theta3)*cos(theta4)*sin(theta3)*sin(theta5) + 0.0098*thetad2*cos(theta2)*cos(theta3)*sin(theta4)*sin(theta5) + 0.0098*thetad2*cos(theta2)*cos(theta4)*sin(theta3)*sin(theta5) + 0.0098*thetad2*cos(theta3)*cos(theta4)*sin(theta2)*sin(theta5) - 0.056*thetad1*cos(theta3)*cos(theta5)*sin(theta3)*sin(theta5) + 0.0098*thetad3*cos(theta2)*cos(theta3)*sin(theta4)*sin(theta5) + 0.0098*thetad3*cos(theta2)*cos(theta4)*sin(theta3)*sin(theta5) + 0.0098*thetad3*cos(theta3)*cos(theta4)*sin(theta2)*sin(theta5) + 0.0098*thetad4*cos(theta2)*cos(theta3)*sin(theta4)*sin(theta5) + 0.0098*thetad4*cos(theta2)*cos(theta4)*sin(theta3)*sin(theta5) + 0.0098*thetad4*cos(theta3)*cos(theta4)*sin(theta2)*sin(theta5) - 0.056*thetad1*cos(theta4)*cos(theta5)*sin(theta4)*sin(theta5) - 0.0098*thetad5*cos(theta2)*cos(theta5)*sin(theta3)*sin(theta4) - 0.0098*thetad5*cos(theta3)*cos(theta5)*sin(theta2)*sin(theta4) - 0.0098*thetad5*cos(theta4)*cos(theta5)*sin(theta2)*sin(theta3) - 0.784*thetad1*cos(theta2)^2*cos(theta3)^2*cos(theta4)^2*sin(theta5) - 0.3332*thetad1*cos(theta2)*sin(theta2)*sin(theta3)*sin(theta4) + 0.7*thetad4*cos(theta1)*sin(theta2)*sin(theta3)*sin(theta4) + 0.35*thetad5*cos(theta1)*sin(theta2)*sin(theta3)*sin(theta4) - 0.049*thetad2*cos(theta5)*sin(theta2)*sin(theta3)*sin(theta4) - 0.049*thetad3*cos(theta5)*sin(theta2)*sin(theta3)*sin(theta4) - 0.049*thetad4*cos(theta5)*sin(theta2)*sin(theta3)*sin(theta4) + 0.049*thetad5*cos(theta2)*sin(theta3)*sin(theta4)*sin(theta5) + 0.049*thetad5*cos(theta3)*sin(theta2)*sin(theta4)*sin(theta5) + 0.049*thetad5*cos(theta4)*sin(theta2)*sin(theta3)*sin(theta5) - 0.1*thetad4*sin(theta1)*sin(theta2)*sin(theta3)*sin(theta4) - 0.05*thetad5*sin(theta1)*sin(theta2)*sin(theta3)*sin(theta4) - 0.0098*thetad2*sin(theta2)*sin(theta3)*sin(theta4)*sin(theta5) - 0.0098*thetad3*sin(theta2)*sin(theta3)*sin(theta4)*sin(theta5) - 0.0098*thetad4*sin(theta2)*sin(theta3)*sin(theta4)*sin(theta5) - 0.88*thetad4*cos(theta1)^2*cos(theta2)*cos(theta3)*cos(theta4) - 0.44*thetad5*cos(theta1)^2*cos(theta2)*cos(theta3)*cos(theta4) - 0.028*thetad2*cos(theta2)*cos(theta3)*cos(theta4)*cos(theta5)^2 - 0.028*thetad3*cos(theta2)*cos(theta3)*cos(theta4)*cos(theta5)^2 - 0.028*thetad4*cos(theta2)*cos(theta3)*cos(theta4)*cos(theta5)^2 + 0.6664*thetad1*cos(theta2)*cos(theta3)^2*cos(theta4)*sin(theta2) + 0.6664*thetad1*cos(theta2)^2*cos(theta3)*cos(theta4)*sin(theta3) + 0.056*thetad1*cos(theta2)^2*cos(theta3)*cos(theta5)*sin(theta4) + 0.056*thetad1*cos(theta2)^2*cos(theta4)*cos(theta5)*sin(theta3) - 1.6072*thetad1*cos(theta2)*cos(theta3)^2*sin(theta2)*sin(theta4) - 1.6072*thetad1*cos(theta2)^2*cos(theta3)*sin(theta3)*sin(theta4) + 0.88*thetad4*cos(theta1)^2*cos(theta2)*sin(theta3)*sin(theta4) + 0.88*thetad4*cos(theta1)^2*cos(theta3)*sin(theta2)*sin(theta4) + 0.88*thetad4*cos(theta1)^2*cos(theta4)*sin(theta2)*sin(theta3) - 0.28*thetad1*cos(theta2)^2*cos(theta3)*sin(theta4)*sin(theta5) - 0.28*thetad1*cos(theta2)^2*cos(theta4)*sin(theta3)*sin(theta5) + 0.44*thetad5*cos(theta1)^2*cos(theta2)*sin(theta3)*sin(theta4) + 0.44*thetad5*cos(theta1)^2*cos(theta3)*sin(theta2)*sin(theta4) + 0.44*thetad5*cos(theta1)^2*cos(theta4)*sin(theta2)*sin(theta3) + 0.028*thetad2*cos(theta2)*cos(theta5)^2*sin(theta3)*sin(theta4) + 0.028*thetad2*cos(theta3)*cos(theta5)^2*sin(theta2)*sin(theta4) + 0.028*thetad2*cos(theta4)*cos(theta5)^2*sin(theta2)*sin(theta3) + 0.028*thetad3*cos(theta2)*cos(theta5)^2*sin(theta3)*sin(theta4) + 0.028*thetad3*cos(theta3)*cos(theta5)^2*sin(theta2)*sin(theta4) + 0.028*thetad3*cos(theta4)*cos(theta5)^2*sin(theta2)*sin(theta3) + 0.028*thetad4*cos(theta2)*cos(theta5)^2*sin(theta3)*sin(theta4) + 0.028*thetad4*cos(theta3)*cos(theta5)^2*sin(theta2)*sin(theta4) + 0.028*thetad4*cos(theta4)*cos(theta5)^2*sin(theta2)*sin(theta3) + 3.14*thetad4*cos(theta1)*cos(theta2)*cos(theta3)*cos(theta4)*sin(theta1) + 1.57*thetad5*cos(theta1)*cos(theta2)*cos(theta3)*cos(theta4)*sin(theta1) + 0.056*thetad1*cos(theta2)*cos(theta3)*cos(theta4)*cos(theta5)*sin(theta2) + 0.0672*thetad2*cos(theta2)*cos(theta3)*cos(theta4)*cos(theta5)*sin(theta5) + 0.0672*thetad3*cos(theta2)*cos(theta3)*cos(theta4)*cos(theta5)*sin(theta5) + 0.0672*thetad4*cos(theta2)*cos(theta3)*cos(theta4)*cos(theta5)*sin(theta5) - 1.6072*thetad1*cos(theta2)*cos(theta3)*cos(theta4)*sin(theta2)*sin(theta3) + 0.0784*thetad1*cos(theta2)*cos(theta3)*cos(theta5)*sin(theta2)*sin(theta3) - 0.28*thetad1*cos(theta2)*cos(theta3)*cos(theta4)*sin(theta2)*sin(theta5) + 0.0784*thetad1*cos(theta2)*cos(theta4)*cos(theta5)*sin(theta2)*sin(theta4) + 0.0784*thetad1*cos(theta3)*cos(theta4)*cos(theta5)*sin(theta3)*sin(theta4) - 0.5376*thetad1*cos(theta2)*cos(theta3)^2*cos(theta4)^2*cos(theta5)^2*sin(theta2) - 0.5376*thetad1*cos(theta2)^2*cos(theta3)*cos(theta4)^2*cos(theta5)^2*sin(theta3) - 0.5376*thetad1*cos(theta2)^2*cos(theta3)^2*cos(theta4)*cos(theta5)^2*sin(theta4) - 0.6664*thetad1*cos(theta2)*cos(theta3)*sin(theta2)*sin(theta3)*sin(theta4) - 3.14*thetad4*cos(theta1)*cos(theta2)*sin(theta1)*sin(theta3)*sin(theta4) - 3.14*thetad4*cos(theta1)*cos(theta3)*sin(theta1)*sin(theta2)*sin(theta4) - 3.14*thetad4*cos(theta1)*cos(theta4)*sin(theta1)*sin(theta2)*sin(theta3) - 0.392*thetad1*cos(theta2)*cos(theta3)*sin(theta2)*sin(theta3)*sin(theta5) - 1.57*thetad5*cos(theta1)*cos(theta2)*sin(theta1)*sin(theta3)*sin(theta4) - 1.57*thetad5*cos(theta1)*cos(theta3)*sin(theta1)*sin(theta2)*sin(theta4) - 1.57*thetad5*cos(theta1)*cos(theta4)*sin(theta1)*sin(theta2)*sin(theta3) - 0.056*thetad1*cos(theta2)*cos(theta5)*sin(theta2)*sin(theta3)*sin(theta4) - 0.392*thetad1*cos(theta2)*cos(theta4)*sin(theta2)*sin(theta4)*sin(theta5) - 0.392*thetad1*cos(theta3)*cos(theta4)*sin(theta3)*sin(theta4)*sin(theta5) - 0.0672*thetad2*cos(theta2)*cos(theta5)*sin(theta3)*sin(theta4)*sin(theta5) - 0.0672*thetad2*cos(theta3)*cos(theta5)*sin(theta2)*sin(theta4)*sin(theta5) - 0.0672*thetad2*cos(theta4)*cos(theta5)*sin(theta2)*sin(theta3)*sin(theta5) - 0.0672*thetad3*cos(theta2)*cos(theta5)*sin(theta3)*sin(theta4)*sin(theta5) - 0.0672*thetad3*cos(theta3)*cos(theta5)*sin(theta2)*sin(theta4)*sin(theta5) - 0.0672*thetad3*cos(theta4)*cos(theta5)*sin(theta2)*sin(theta3)*sin(theta5) - 0.0672*thetad4*cos(theta2)*cos(theta5)*sin(theta3)*sin(theta4)*sin(theta5) - 0.0672*thetad4*cos(theta3)*cos(theta5)*sin(theta2)*sin(theta4)*sin(theta5) - 0.0672*thetad4*cos(theta4)*cos(theta5)*sin(theta2)*sin(theta3)*sin(theta5) + 0.28*thetad1*cos(theta2)*sin(theta2)*sin(theta3)*sin(theta4)*sin(theta5) + 0.112*thetad1*cos(theta2)*cos(theta3)^2*cos(theta4)*cos(theta5)*sin(theta2) + 0.112*thetad1*cos(theta2)^2*cos(theta3)*cos(theta4)*cos(theta5)*sin(theta3) - 0.826336*thetad1*cos(theta2)*cos(theta3)*cos(theta4)^2*sin(theta2)*sin(theta3) - 0.826336*thetad1*cos(theta2)*cos(theta3)^2*cos(theta4)*sin(theta2)*sin(theta4) - 0.56*thetad1*cos(theta2)*cos(theta3)^2*cos(theta4)*sin(theta2)*sin(theta5) - 0.826336*thetad1*cos(theta2)^2*cos(theta3)*cos(theta4)*sin(theta3)*sin(theta4) + 0.112*thetad1*cos(theta2)*cos(theta3)^2*cos(theta5)*sin(theta2)*sin(theta5) - 0.56*thetad1*cos(theta2)^2*cos(theta3)*cos(theta4)*sin(theta3)*sin(theta5) + 0.112*thetad1*cos(theta2)*cos(theta4)^2*cos(theta5)*sin(theta2)*sin(theta5) + 0.112*thetad1*cos(theta2)^2*cos(theta3)*cos(theta5)*sin(theta3)*sin(theta5) + 0.112*thetad1*cos(theta3)*cos(theta4)^2*cos(theta5)*sin(theta3)*sin(theta5) + 0.112*thetad1*cos(theta2)^2*cos(theta4)*cos(theta5)*sin(theta4)*sin(theta5) + 0.112*thetad1*cos(theta3)^2*cos(theta4)*cos(theta5)*sin(theta4)*sin(theta5) + 0.241248*thetad1*cos(theta2)*cos(theta3)*cos(theta4)*sin(theta2)*sin(theta3)*sin(theta4) - 0.112*thetad1*cos(theta2)*cos(theta3)*cos(theta5)*sin(theta2)*sin(theta3)*sin(theta4) + 0.56*thetad1*cos(theta2)*cos(theta3)*sin(theta2)*sin(theta3)*sin(theta4)*sin(theta5) - 0.1568*thetad1*cos(theta2)*cos(theta3)*cos(theta4)^2*cos(theta5)*sin(theta2)*sin(theta3) - 0.1568*thetad1*cos(theta2)*cos(theta3)^2*cos(theta4)*cos(theta5)*sin(theta2)*sin(theta4) - 0.1568*thetad1*cos(theta2)^2*cos(theta3)*cos(theta4)*cos(theta5)*sin(theta3)*sin(theta4) + 0.784*thetad1*cos(theta2)*cos(theta3)*cos(theta4)^2*sin(theta2)*sin(theta3)*sin(theta5) + 0.784*thetad1*cos(theta2)*cos(theta3)^2*cos(theta4)*sin(theta2)*sin(theta4)*sin(theta5) + 0.784*thetad1*cos(theta2)^2*cos(theta3)*cos(theta4)*sin(theta3)*sin(theta4)*sin(theta5) - 0.224*thetad1*cos(theta2)*cos(theta3)^2*cos(theta4)^2*cos(theta5)*sin(theta2)*sin(theta5) - 0.224*thetad1*cos(theta2)^2*cos(theta3)*cos(theta4)^2*cos(theta5)*sin(theta3)*sin(theta5) - 0.224*thetad1*cos(theta2)^2*cos(theta3)^2*cos(theta4)*cos(theta5)*sin(theta4)*sin(theta5) + 0.5376*thetad1*cos(theta2)*cos(theta3)*cos(theta4)*cos(theta5)^2*sin(theta2)*sin(theta3)*sin(theta4) + 0.224*thetad1*cos(theta2)*cos(theta3)*cos(theta4)*cos(theta5)*sin(theta2)*sin(theta3)*sin(theta4)*sin(theta5) ;
C(2,2) = 0.4875*thetad1*sin(theta2)*sin(theta3) - 0.053508*thetad1*sin(theta2) - 0.4875*thetad1*cos(theta2)*cos(theta3) - 0.07*thetad1*cos(theta2)*cos(theta5) - 0.150528*thetad1*cos(theta2)*sin(theta3) - 0.150528*thetad1*cos(theta3)*sin(theta2) - 0.014*thetad1*cos(theta2)*sin(theta5) - 0.441816*thetad1*cos(theta2) - 0.190918*thetad1*cos(theta2)*cos(theta3)*cos(theta4) - 0.07*thetad1*cos(theta2)*cos(theta3)*cos(theta5) + 0.44*thetad4*cos(theta2)*cos(theta3)*cos(theta4) + 0.22*thetad5*cos(theta2)*cos(theta3)*cos(theta4) + 0.373674*thetad1*cos(theta2)*cos(theta3)*sin(theta4) + 0.373674*thetad1*cos(theta2)*cos(theta4)*sin(theta3) + 0.373674*thetad1*cos(theta3)*cos(theta4)*sin(theta2) - 0.014*thetad1*cos(theta2)*cos(theta3)*sin(theta5) + 0.190918*thetad1*cos(theta2)*sin(theta3)*sin(theta4) + 0.190918*thetad1*cos(theta3)*sin(theta2)*sin(theta4) + 0.190918*thetad1*cos(theta4)*sin(theta2)*sin(theta3) + 0.07*thetad1*cos(theta5)*sin(theta2)*sin(theta3) - 0.44*thetad4*cos(theta2)*sin(theta3)*sin(theta4) - 0.44*thetad4*cos(theta3)*sin(theta2)*sin(theta4) - 0.44*thetad4*cos(theta4)*sin(theta2)*sin(theta3) - 0.22*thetad5*cos(theta2)*sin(theta3)*sin(theta4) - 0.22*thetad5*cos(theta3)*sin(theta2)*sin(theta4) - 0.22*thetad5*cos(theta4)*sin(theta2)*sin(theta3) - 0.373674*thetad1*sin(theta2)*sin(theta3)*sin(theta4) + 0.014*thetad1*sin(theta2)*sin(theta3)*sin(theta5) - 0.7*thetad4*cos(theta1)*cos(theta2)*cos(theta3)*sin(theta4) - 0.7*thetad4*cos(theta1)*cos(theta2)*cos(theta4)*sin(theta3) - 0.7*thetad4*cos(theta1)*cos(theta3)*cos(theta4)*sin(theta2) + 0.049*thetad1*cos(theta2)*cos(theta3)*cos(theta5)*sin(theta4) + 0.049*thetad1*cos(theta2)*cos(theta4)*cos(theta5)*sin(theta3) + 0.049*thetad1*cos(theta3)*cos(theta4)*cos(theta5)*sin(theta2) - 0.35*thetad5*cos(theta1)*cos(theta2)*cos(theta3)*sin(theta4) - 0.35*thetad5*cos(theta1)*cos(theta2)*cos(theta4)*sin(theta3) - 0.35*thetad5*cos(theta1)*cos(theta3)*cos(theta4)*sin(theta2) + 0.1*thetad4*cos(theta2)*cos(theta3)*sin(theta1)*sin(theta4) + 0.1*thetad4*cos(theta2)*cos(theta4)*sin(theta1)*sin(theta3) + 0.1*thetad4*cos(theta3)*cos(theta4)*sin(theta1)*sin(theta2) + 0.0098*thetad1*cos(theta2)*cos(theta3)*sin(theta4)*sin(theta5) + 0.0098*thetad1*cos(theta2)*cos(theta4)*sin(theta3)*sin(theta5) + 0.0098*thetad1*cos(theta3)*cos(theta4)*sin(theta2)*sin(theta5) + 0.05*thetad5*cos(theta2)*cos(theta3)*sin(theta1)*sin(theta4) + 0.05*thetad5*cos(theta2)*cos(theta4)*sin(theta1)*sin(theta3) + 0.05*thetad5*cos(theta3)*cos(theta4)*sin(theta1)*sin(theta2) + 0.7*thetad4*cos(theta1)*sin(theta2)*sin(theta3)*sin(theta4) - 0.049*thetad1*cos(theta5)*sin(theta2)*sin(theta3)*sin(theta4) + 0.35*thetad5*cos(theta1)*sin(theta2)*sin(theta3)*sin(theta4) - 0.1*thetad4*sin(theta1)*sin(theta2)*sin(theta3)*sin(theta4) - 0.0098*thetad1*sin(theta2)*sin(theta3)*sin(theta4)*sin(theta5) - 0.05*thetad5*sin(theta1)*sin(theta2)*sin(theta3)*sin(theta4) - 0.88*thetad4*cos(theta1)^2*cos(theta2)*cos(theta3)*cos(theta4) - 0.028*thetad1*cos(theta2)*cos(theta3)*cos(theta4)*cos(theta5)^2 - 0.44*thetad5*cos(theta1)^2*cos(theta2)*cos(theta3)*cos(theta4) + 0.88*thetad4*cos(theta1)^2*cos(theta2)*sin(theta3)*sin(theta4) + 0.88*thetad4*cos(theta1)^2*cos(theta3)*sin(theta2)*sin(theta4) + 0.88*thetad4*cos(theta1)^2*cos(theta4)*sin(theta2)*sin(theta3) + 0.028*thetad1*cos(theta2)*cos(theta5)^2*sin(theta3)*sin(theta4) + 0.028*thetad1*cos(theta3)*cos(theta5)^2*sin(theta2)*sin(theta4) + 0.028*thetad1*cos(theta4)*cos(theta5)^2*sin(theta2)*sin(theta3) + 0.44*thetad5*cos(theta1)^2*cos(theta2)*sin(theta3)*sin(theta4) + 0.44*thetad5*cos(theta1)^2*cos(theta3)*sin(theta2)*sin(theta4) + 0.44*thetad5*cos(theta1)^2*cos(theta4)*sin(theta2)*sin(theta3) + 3.14*thetad4*cos(theta1)*cos(theta2)*cos(theta3)*cos(theta4)*sin(theta1) + 1.57*thetad5*cos(theta1)*cos(theta2)*cos(theta3)*cos(theta4)*sin(theta1) + 0.0672*thetad1*cos(theta2)*cos(theta3)*cos(theta4)*cos(theta5)*sin(theta5) - 3.14*thetad4*cos(theta1)*cos(theta2)*sin(theta1)*sin(theta3)*sin(theta4) - 3.14*thetad4*cos(theta1)*cos(theta3)*sin(theta1)*sin(theta2)*sin(theta4) - 3.14*thetad4*cos(theta1)*cos(theta4)*sin(theta1)*sin(theta2)*sin(theta3) - 1.57*thetad5*cos(theta1)*cos(theta2)*sin(theta1)*sin(theta3)*sin(theta4) - 1.57*thetad5*cos(theta1)*cos(theta3)*sin(theta1)*sin(theta2)*sin(theta4) - 1.57*thetad5*cos(theta1)*cos(theta4)*sin(theta1)*sin(theta2)*sin(theta3) - 0.0672*thetad1*cos(theta2)*cos(theta5)*sin(theta3)*sin(theta4)*sin(theta5) - 0.0672*thetad1*cos(theta3)*cos(theta5)*sin(theta2)*sin(theta4)*sin(theta5) - 0.0672*thetad1*cos(theta4)*cos(theta5)*sin(theta2)*sin(theta3)*sin(theta5) ;
C(2,3) = 0.4875*thetad1*sin(theta2)*sin(theta3) - 0.150528*thetad1*cos(theta2)*sin(theta3) - 0.150528*thetad1*cos(theta3)*sin(theta2) - 0.4875*thetad1*cos(theta2)*cos(theta3) - 0.190918*thetad1*cos(theta2)*cos(theta3)*cos(theta4) - 0.07*thetad1*cos(theta2)*cos(theta3)*cos(theta5) + 0.44*thetad4*cos(theta2)*cos(theta3)*cos(theta4) + 0.22*thetad5*cos(theta2)*cos(theta3)*cos(theta4) + 0.373674*thetad1*cos(theta2)*cos(theta3)*sin(theta4) + 0.373674*thetad1*cos(theta2)*cos(theta4)*sin(theta3) + 0.373674*thetad1*cos(theta3)*cos(theta4)*sin(theta2) - 0.014*thetad1*cos(theta2)*cos(theta3)*sin(theta5) + 0.190918*thetad1*cos(theta2)*sin(theta3)*sin(theta4) + 0.190918*thetad1*cos(theta3)*sin(theta2)*sin(theta4) + 0.190918*thetad1*cos(theta4)*sin(theta2)*sin(theta3) + 0.07*thetad1*cos(theta5)*sin(theta2)*sin(theta3) - 0.44*thetad4*cos(theta2)*sin(theta3)*sin(theta4) - 0.44*thetad4*cos(theta3)*sin(theta2)*sin(theta4) - 0.44*thetad4*cos(theta4)*sin(theta2)*sin(theta3) - 0.22*thetad5*cos(theta2)*sin(theta3)*sin(theta4) - 0.22*thetad5*cos(theta3)*sin(theta2)*sin(theta4) - 0.22*thetad5*cos(theta4)*sin(theta2)*sin(theta3) - 0.373674*thetad1*sin(theta2)*sin(theta3)*sin(theta4) + 0.014*thetad1*sin(theta2)*sin(theta3)*sin(theta5) - 0.7*thetad4*cos(theta1)*cos(theta2)*cos(theta3)*sin(theta4) - 0.7*thetad4*cos(theta1)*cos(theta2)*cos(theta4)*sin(theta3) - 0.7*thetad4*cos(theta1)*cos(theta3)*cos(theta4)*sin(theta2) + 0.049*thetad1*cos(theta2)*cos(theta3)*cos(theta5)*sin(theta4) + 0.049*thetad1*cos(theta2)*cos(theta4)*cos(theta5)*sin(theta3) + 0.049*thetad1*cos(theta3)*cos(theta4)*cos(theta5)*sin(theta2) - 0.35*thetad5*cos(theta1)*cos(theta2)*cos(theta3)*sin(theta4) - 0.35*thetad5*cos(theta1)*cos(theta2)*cos(theta4)*sin(theta3) - 0.35*thetad5*cos(theta1)*cos(theta3)*cos(theta4)*sin(theta2) + 0.1*thetad4*cos(theta2)*cos(theta3)*sin(theta1)*sin(theta4) + 0.1*thetad4*cos(theta2)*cos(theta4)*sin(theta1)*sin(theta3) + 0.1*thetad4*cos(theta3)*cos(theta4)*sin(theta1)*sin(theta2) + 0.0098*thetad1*cos(theta2)*cos(theta3)*sin(theta4)*sin(theta5) + 0.0098*thetad1*cos(theta2)*cos(theta4)*sin(theta3)*sin(theta5) + 0.0098*thetad1*cos(theta3)*cos(theta4)*sin(theta2)*sin(theta5) + 0.05*thetad5*cos(theta2)*cos(theta3)*sin(theta1)*sin(theta4) + 0.05*thetad5*cos(theta2)*cos(theta4)*sin(theta1)*sin(theta3) + 0.05*thetad5*cos(theta3)*cos(theta4)*sin(theta1)*sin(theta2) + 0.7*thetad4*cos(theta1)*sin(theta2)*sin(theta3)*sin(theta4) - 0.049*thetad1*cos(theta5)*sin(theta2)*sin(theta3)*sin(theta4) + 0.35*thetad5*cos(theta1)*sin(theta2)*sin(theta3)*sin(theta4) - 0.1*thetad4*sin(theta1)*sin(theta2)*sin(theta3)*sin(theta4) - 0.0098*thetad1*sin(theta2)*sin(theta3)*sin(theta4)*sin(theta5) - 0.05*thetad5*sin(theta1)*sin(theta2)*sin(theta3)*sin(theta4) - 0.88*thetad4*cos(theta1)^2*cos(theta2)*cos(theta3)*cos(theta4) - 0.028*thetad1*cos(theta2)*cos(theta3)*cos(theta4)*cos(theta5)^2 - 0.44*thetad5*cos(theta1)^2*cos(theta2)*cos(theta3)*cos(theta4) + 0.88*thetad4*cos(theta1)^2*cos(theta2)*sin(theta3)*sin(theta4) + 0.88*thetad4*cos(theta1)^2*cos(theta3)*sin(theta2)*sin(theta4) + 0.88*thetad4*cos(theta1)^2*cos(theta4)*sin(theta2)*sin(theta3) + 0.028*thetad1*cos(theta2)*cos(theta5)^2*sin(theta3)*sin(theta4) + 0.028*thetad1*cos(theta3)*cos(theta5)^2*sin(theta2)*sin(theta4) + 0.028*thetad1*cos(theta4)*cos(theta5)^2*sin(theta2)*sin(theta3) + 0.44*thetad5*cos(theta1)^2*cos(theta2)*sin(theta3)*sin(theta4) + 0.44*thetad5*cos(theta1)^2*cos(theta3)*sin(theta2)*sin(theta4) + 0.44*thetad5*cos(theta1)^2*cos(theta4)*sin(theta2)*sin(theta3) + 3.14*thetad4*cos(theta1)*cos(theta2)*cos(theta3)*cos(theta4)*sin(theta1) + 1.57*thetad5*cos(theta1)*cos(theta2)*cos(theta3)*cos(theta4)*sin(theta1) + 0.0672*thetad1*cos(theta2)*cos(theta3)*cos(theta4)*cos(theta5)*sin(theta5) - 3.14*thetad4*cos(theta1)*cos(theta2)*sin(theta1)*sin(theta3)*sin(theta4) - 3.14*thetad4*cos(theta1)*cos(theta3)*sin(theta1)*sin(theta2)*sin(theta4) - 3.14*thetad4*cos(theta1)*cos(theta4)*sin(theta1)*sin(theta2)*sin(theta3) - 1.57*thetad5*cos(theta1)*cos(theta2)*sin(theta1)*sin(theta3)*sin(theta4) - 1.57*thetad5*cos(theta1)*cos(theta3)*sin(theta1)*sin(theta2)*sin(theta4) - 1.57*thetad5*cos(theta1)*cos(theta4)*sin(theta1)*sin(theta2)*sin(theta3) - 0.0672*thetad1*cos(theta2)*cos(theta5)*sin(theta3)*sin(theta4)*sin(theta5) - 0.0672*thetad1*cos(theta3)*cos(theta5)*sin(theta2)*sin(theta4)*sin(theta5) - 0.0672*thetad1*cos(theta4)*cos(theta5)*sin(theta2)*sin(theta3)*sin(theta5) ;
C(2,4) = 5.64*thetad4*cos(theta2)*sin(theta2) - 0.1*thetad5*cos(theta1) - 1.4*thetad4*sin(theta1) - 0.7*thetad5*sin(theta1) - 0.2*thetad4*cos(theta1) + 2.82*thetad5*cos(theta2)*sin(theta2) + 5.64*thetad4*cos(theta3)*sin(theta3) + 2.82*thetad5*cos(theta3)*sin(theta3) + 5.64*thetad4*cos(theta4)*sin(theta4) + 2.82*thetad5*cos(theta4)*sin(theta4) + 0.4*thetad4*cos(theta1)*cos(theta2)^2 + 0.4*thetad4*cos(theta1)*cos(theta3)^2 + 0.2*thetad5*cos(theta1)*cos(theta2)^2 + 0.4*thetad4*cos(theta1)*cos(theta4)^2 + 0.2*thetad5*cos(theta1)*cos(theta3)^2 + 0.2*thetad5*cos(theta1)*cos(theta4)^2 + 2.8*thetad4*cos(theta2)^2*sin(theta1) + 2.8*thetad4*cos(theta3)^2*sin(theta1) + 1.4*thetad5*cos(theta2)^2*sin(theta1) + 2.8*thetad4*cos(theta4)^2*sin(theta1) + 1.4*thetad5*cos(theta3)^2*sin(theta1) + 1.4*thetad5*cos(theta4)^2*sin(theta1) - 0.8*thetad4*cos(theta1)*cos(theta2)^2*cos(theta3)^2 - 0.8*thetad4*cos(theta1)*cos(theta2)^2*cos(theta4)^2 - 0.4*thetad5*cos(theta1)*cos(theta2)^2*cos(theta3)^2 - 0.8*thetad4*cos(theta1)*cos(theta3)^2*cos(theta4)^2 - 0.4*thetad5*cos(theta1)*cos(theta2)^2*cos(theta4)^2 - 0.4*thetad5*cos(theta1)*cos(theta3)^2*cos(theta4)^2 - 5.6*thetad4*cos(theta2)^2*cos(theta3)^2*sin(theta1) - 5.6*thetad4*cos(theta2)^2*cos(theta4)^2*sin(theta1) - 2.8*thetad5*cos(theta2)^2*cos(theta3)^2*sin(theta1) - 5.6*thetad4*cos(theta3)^2*cos(theta4)^2*sin(theta1) - 2.8*thetad5*cos(theta2)^2*cos(theta4)^2*sin(theta1) - 2.8*thetad5*cos(theta3)^2*cos(theta4)^2*sin(theta1) + 0.249082*thetad1*cos(theta2)*cos(theta3)*cos(theta4) + 0.44*thetad2*cos(theta2)*cos(theta3)*cos(theta4) + 0.44*thetad3*cos(theta2)*cos(theta3)*cos(theta4) + 0.373674*thetad1*cos(theta2)*cos(theta3)*sin(theta4) + 0.373674*thetad1*cos(theta2)*cos(theta4)*sin(theta3) + 0.373674*thetad1*cos(theta3)*cos(theta4)*sin(theta2) - 0.249082*thetad1*cos(theta2)*sin(theta3)*sin(theta4) - 0.249082*thetad1*cos(theta3)*sin(theta2)*sin(theta4) - 0.249082*thetad1*cos(theta4)*sin(theta2)*sin(theta3) - 0.44*thetad2*cos(theta2)*sin(theta3)*sin(theta4) - 0.44*thetad2*cos(theta3)*sin(theta2)*sin(theta4) - 0.44*thetad2*cos(theta4)*sin(theta2)*sin(theta3) - 0.44*thetad3*cos(theta2)*sin(theta3)*sin(theta4) - 0.44*thetad3*cos(theta3)*sin(theta2)*sin(theta4) - 0.44*thetad3*cos(theta4)*sin(theta2)*sin(theta3) - 0.373674*thetad1*sin(theta2)*sin(theta3)*sin(theta4) - 6.28*thetad4*cos(theta1)^2*cos(theta2)*sin(theta2) - 3.14*thetad5*cos(theta1)^2*cos(theta2)*sin(theta2) - 11.28*thetad4*cos(theta2)*cos(theta3)^2*sin(theta2) - 6.28*thetad4*cos(theta1)^2*cos(theta3)*sin(theta3) - 11.28*thetad4*cos(theta2)*cos(theta4)^2*sin(theta2) - 11.28*thetad4*cos(theta2)^2*cos(theta3)*sin(theta3) - 5.64*thetad5*cos(theta2)*cos(theta3)^2*sin(theta2) - 3.14*thetad5*cos(theta1)^2*cos(theta3)*sin(theta3) - 6.28*thetad4*cos(theta1)^2*cos(theta4)*sin(theta4) - 5.64*thetad5*cos(theta2)*cos(theta4)^2*sin(theta2) - 5.64*thetad5*cos(theta2)^2*cos(theta3)*sin(theta3) - 11.28*thetad4*cos(theta3)*cos(theta4)^2*sin(theta3) - 11.28*thetad4*cos(theta2)^2*cos(theta4)*sin(theta4) - 3.14*thetad5*cos(theta1)^2*cos(theta4)*sin(theta4) - 11.28*thetad4*cos(theta3)^2*cos(theta4)*sin(theta4) - 5.64*thetad5*cos(theta3)*cos(theta4)^2*sin(theta3) - 5.64*thetad5*cos(theta2)^2*cos(theta4)*sin(theta4) - 5.64*thetad5*cos(theta3)^2*cos(theta4)*sin(theta4) + 12.56*thetad4*cos(theta1)^2*cos(theta2)*cos(theta3)^2*sin(theta2) + 12.56*thetad4*cos(theta1)^2*cos(theta2)*cos(theta4)^2*sin(theta2) + 12.56*thetad4*cos(theta1)^2*cos(theta2)^2*cos(theta3)*sin(theta3) + 6.28*thetad5*cos(theta1)^2*cos(theta2)*cos(theta3)^2*sin(theta2) + 6.28*thetad5*cos(theta1)^2*cos(theta2)*cos(theta4)^2*sin(theta2) + 6.28*thetad5*cos(theta1)^2*cos(theta2)^2*cos(theta3)*sin(theta3) + 22.56*thetad4*cos(theta2)*cos(theta3)^2*cos(theta4)^2*sin(theta2) + 12.56*thetad4*cos(theta1)^2*cos(theta3)*cos(theta4)^2*sin(theta3) + 12.56*thetad4*cos(theta1)^2*cos(theta2)^2*cos(theta4)*sin(theta4) + 12.56*thetad4*cos(theta1)^2*cos(theta3)^2*cos(theta4)*sin(theta4) + 22.56*thetad4*cos(theta2)^2*cos(theta3)*cos(theta4)^2*sin(theta3) + 11.28*thetad5*cos(theta2)*cos(theta3)^2*cos(theta4)^2*sin(theta2) + 6.28*thetad5*cos(theta1)^2*cos(theta3)*cos(theta4)^2*sin(theta3) + 6.28*thetad5*cos(theta1)^2*cos(theta2)^2*cos(theta4)*sin(theta4) + 22.56*thetad4*cos(theta2)^2*cos(theta3)^2*cos(theta4)*sin(theta4) + 6.28*thetad5*cos(theta1)^2*cos(theta3)^2*cos(theta4)*sin(theta4) + 11.28*thetad5*cos(theta2)^2*cos(theta3)*cos(theta4)^2*sin(theta3) + 11.28*thetad5*cos(theta2)^2*cos(theta3)^2*cos(theta4)*sin(theta4) - 0.7*thetad1*cos(theta1)*cos(theta2)*cos(theta3)*sin(theta4) - 0.7*thetad1*cos(theta1)*cos(theta2)*cos(theta4)*sin(theta3) - 0.7*thetad1*cos(theta1)*cos(theta3)*cos(theta4)*sin(theta2) - 0.7*thetad2*cos(theta1)*cos(theta2)*cos(theta3)*sin(theta4) - 0.7*thetad2*cos(theta1)*cos(theta2)*cos(theta4)*sin(theta3) - 0.7*thetad2*cos(theta1)*cos(theta3)*cos(theta4)*sin(theta2) - 0.7*thetad3*cos(theta1)*cos(theta2)*cos(theta3)*sin(theta4) - 0.7*thetad3*cos(theta1)*cos(theta2)*cos(theta4)*sin(theta3) - 0.7*thetad3*cos(theta1)*cos(theta3)*cos(theta4)*sin(theta2) + 0.049*thetad1*cos(theta2)*cos(theta3)*cos(theta5)*sin(theta4) + 0.049*thetad1*cos(theta2)*cos(theta4)*cos(theta5)*sin(theta3) + 0.049*thetad1*cos(theta3)*cos(theta4)*cos(theta5)*sin(theta2) + 1.6*thetad4*cos(theta1)*cos(theta2)^2*cos(theta3)^2*cos(theta4)^2 + 0.8*thetad5*cos(theta1)*cos(theta2)^2*cos(theta3)^2*cos(theta4)^2 - 1.76*thetad4*cos(theta1)*cos(theta2)*sin(theta1)*sin(theta2) + 0.1*thetad1*cos(theta2)*cos(theta3)*sin(theta1)*sin(theta4) + 0.1*thetad1*cos(theta2)*cos(theta4)*sin(theta1)*sin(theta3) + 0.1*thetad1*cos(theta3)*cos(theta4)*sin(theta1)*sin(theta2) - 0.88*thetad5*cos(theta1)*cos(theta2)*sin(theta1)*sin(theta2) + 0.1*thetad2*cos(theta2)*cos(theta3)*sin(theta1)*sin(theta4) + 0.1*thetad2*cos(theta2)*cos(theta4)*sin(theta1)*sin(theta3) + 0.1*thetad2*cos(theta3)*cos(theta4)*sin(theta1)*sin(theta2) - 1.76*thetad4*cos(theta1)*cos(theta3)*sin(theta1)*sin(theta3) + 0.1*thetad3*cos(theta2)*cos(theta3)*sin(theta1)*sin(theta4) + 0.1*thetad3*cos(theta2)*cos(theta4)*sin(theta1)*sin(theta3) + 0.1*thetad3*cos(theta3)*cos(theta4)*sin(theta1)*sin(theta2) - 0.88*thetad5*cos(theta1)*cos(theta3)*sin(theta1)*sin(theta3) - 1.76*thetad4*cos(theta1)*cos(theta4)*sin(theta1)*sin(theta4) + 0.0098*thetad1*cos(theta2)*cos(theta3)*sin(theta4)*sin(theta5) + 0.0098*thetad1*cos(theta2)*cos(theta4)*sin(theta3)*sin(theta5) + 0.0098*thetad1*cos(theta3)*cos(theta4)*sin(theta2)*sin(theta5) - 0.88*thetad5*cos(theta1)*cos(theta4)*sin(theta1)*sin(theta4) + 11.2*thetad4*cos(theta2)^2*cos(theta3)^2*cos(theta4)^2*sin(theta1) + 5.6*thetad5*cos(theta2)^2*cos(theta3)^2*cos(theta4)^2*sin(theta1) + 0.7*thetad1*cos(theta1)*sin(theta2)*sin(theta3)*sin(theta4) + 0.7*thetad2*cos(theta1)*sin(theta2)*sin(theta3)*sin(theta4) + 0.7*thetad3*cos(theta1)*sin(theta2)*sin(theta3)*sin(theta4) - 0.049*thetad1*cos(theta5)*sin(theta2)*sin(theta3)*sin(theta4) - 0.1*thetad1*sin(theta1)*sin(theta2)*sin(theta3)*sin(theta4) - 0.1*thetad2*sin(theta1)*sin(theta2)*sin(theta3)*sin(theta4) - 0.1*thetad3*sin(theta1)*sin(theta2)*sin(theta3)*sin(theta4) - 0.0098*thetad1*sin(theta2)*sin(theta3)*sin(theta4)*sin(theta5) - 0.88*thetad1*cos(theta1)^2*cos(theta2)*cos(theta3)*cos(theta4) - 0.88*thetad2*cos(theta1)^2*cos(theta2)*cos(theta3)*cos(theta4) - 0.88*thetad3*cos(theta1)^2*cos(theta2)*cos(theta3)*cos(theta4) - 0.028*thetad1*cos(theta2)*cos(theta3)*cos(theta4)*cos(theta5)^2 + 0.88*thetad1*cos(theta1)^2*cos(theta2)*sin(theta3)*sin(theta4) + 0.88*thetad1*cos(theta1)^2*cos(theta3)*sin(theta2)*sin(theta4) + 0.88*thetad1*cos(theta1)^2*cos(theta4)*sin(theta2)*sin(theta3) + 0.88*thetad2*cos(theta1)^2*cos(theta2)*sin(theta3)*sin(theta4) + 0.88*thetad2*cos(theta1)^2*cos(theta3)*sin(theta2)*sin(theta4) + 0.88*thetad2*cos(theta1)^2*cos(theta4)*sin(theta2)*sin(theta3) + 0.88*thetad3*cos(theta1)^2*cos(theta2)*sin(theta3)*sin(theta4) + 0.88*thetad3*cos(theta1)^2*cos(theta3)*sin(theta2)*sin(theta4) + 0.88*thetad3*cos(theta1)^2*cos(theta4)*sin(theta2)*sin(theta3) + 0.028*thetad1*cos(theta2)*cos(theta5)^2*sin(theta3)*sin(theta4) + 0.028*thetad1*cos(theta3)*cos(theta5)^2*sin(theta2)*sin(theta4) + 0.028*thetad1*cos(theta4)*cos(theta5)^2*sin(theta2)*sin(theta3) + 3.14*thetad1*cos(theta1)*cos(theta2)*cos(theta3)*cos(theta4)*sin(theta1) + 3.14*thetad2*cos(theta1)*cos(theta2)*cos(theta3)*cos(theta4)*sin(theta1) + 3.14*thetad3*cos(theta1)*cos(theta2)*cos(theta3)*cos(theta4)*sin(theta1) + 0.0672*thetad1*cos(theta2)*cos(theta3)*cos(theta4)*cos(theta5)*sin(theta5) + 0.8*thetad4*cos(theta1)*cos(theta2)*cos(theta3)*sin(theta2)*sin(theta3) + 0.4*thetad5*cos(theta1)*cos(theta2)*cos(theta3)*sin(theta2)*sin(theta3) + 0.8*thetad4*cos(theta1)*cos(theta2)*cos(theta4)*sin(theta2)*sin(theta4) + 0.4*thetad5*cos(theta1)*cos(theta2)*cos(theta4)*sin(theta2)*sin(theta4) + 0.8*thetad4*cos(theta1)*cos(theta3)*cos(theta4)*sin(theta3)*sin(theta4) + 0.4*thetad5*cos(theta1)*cos(theta3)*cos(theta4)*sin(theta3)*sin(theta4) - 25.12*thetad4*cos(theta1)^2*cos(theta2)*cos(theta3)^2*cos(theta4)^2*sin(theta2) - 25.12*thetad4*cos(theta1)^2*cos(theta2)^2*cos(theta3)*cos(theta4)^2*sin(theta3) - 12.56*thetad5*cos(theta1)^2*cos(theta2)*cos(theta3)^2*cos(theta4)^2*sin(theta2) - 25.12*thetad4*cos(theta1)^2*cos(theta2)^2*cos(theta3)^2*cos(theta4)*sin(theta4) - 12.56*thetad5*cos(theta1)^2*cos(theta2)^2*cos(theta3)*cos(theta4)^2*sin(theta3) - 12.56*thetad5*cos(theta1)^2*cos(theta2)^2*cos(theta3)^2*cos(theta4)*sin(theta4) - 3.14*thetad1*cos(theta1)*cos(theta2)*sin(theta1)*sin(theta3)*sin(theta4) - 3.14*thetad1*cos(theta1)*cos(theta3)*sin(theta1)*sin(theta2)*sin(theta4) - 3.14*thetad1*cos(theta1)*cos(theta4)*sin(theta1)*sin(theta2)*sin(theta3) - 3.14*thetad2*cos(theta1)*cos(theta2)*sin(theta1)*sin(theta3)*sin(theta4) - 3.14*thetad2*cos(theta1)*cos(theta3)*sin(theta1)*sin(theta2)*sin(theta4) - 3.14*thetad2*cos(theta1)*cos(theta4)*sin(theta1)*sin(theta2)*sin(theta3) - 3.14*thetad3*cos(theta1)*cos(theta2)*sin(theta1)*sin(theta3)*sin(theta4) - 3.14*thetad3*cos(theta1)*cos(theta3)*sin(theta1)*sin(theta2)*sin(theta4) - 3.14*thetad3*cos(theta1)*cos(theta4)*sin(theta1)*sin(theta2)*sin(theta3) + 5.6*thetad4*cos(theta2)*cos(theta3)*sin(theta1)*sin(theta2)*sin(theta3) + 2.8*thetad5*cos(theta2)*cos(theta3)*sin(theta1)*sin(theta2)*sin(theta3) + 5.6*thetad4*cos(theta2)*cos(theta4)*sin(theta1)*sin(theta2)*sin(theta4) + 2.8*thetad5*cos(theta2)*cos(theta4)*sin(theta1)*sin(theta2)*sin(theta4) + 5.6*thetad4*cos(theta3)*cos(theta4)*sin(theta1)*sin(theta3)*sin(theta4) - 0.0672*thetad1*cos(theta2)*cos(theta5)*sin(theta3)*sin(theta4)*sin(theta5) - 0.0672*thetad1*cos(theta3)*cos(theta5)*sin(theta2)*sin(theta4)*sin(theta5) - 0.0672*thetad1*cos(theta4)*cos(theta5)*sin(theta2)*sin(theta3)*sin(theta5) + 2.8*thetad5*cos(theta3)*cos(theta4)*sin(theta1)*sin(theta3)*sin(theta4) + 3.52*thetad4*cos(theta1)*cos(theta2)*cos(theta3)^2*sin(theta1)*sin(theta2) + 3.52*thetad4*cos(theta1)*cos(theta2)*cos(theta4)^2*sin(theta1)*sin(theta2) + 3.52*thetad4*cos(theta1)*cos(theta2)^2*cos(theta3)*sin(theta1)*sin(theta3) + 1.76*thetad5*cos(theta1)*cos(theta2)*cos(theta3)^2*sin(theta1)*sin(theta2) + 1.76*thetad5*cos(theta1)*cos(theta2)*cos(theta4)^2*sin(theta1)*sin(theta2) + 1.76*thetad5*cos(theta1)*cos(theta2)^2*cos(theta3)*sin(theta1)*sin(theta3) + 3.52*thetad4*cos(theta1)*cos(theta3)*cos(theta4)^2*sin(theta1)*sin(theta3) + 3.52*thetad4*cos(theta1)*cos(theta2)^2*cos(theta4)*sin(theta1)*sin(theta4) + 3.52*thetad4*cos(theta1)*cos(theta3)^2*cos(theta4)*sin(theta1)*sin(theta4) + 1.76*thetad5*cos(theta1)*cos(theta3)*cos(theta4)^2*sin(theta1)*sin(theta3) + 1.76*thetad5*cos(theta1)*cos(theta2)^2*cos(theta4)*sin(theta1)*sin(theta4) + 1.76*thetad5*cos(theta1)*cos(theta3)^2*cos(theta4)*sin(theta1)*sin(theta4) - 22.56*thetad4*cos(theta2)*cos(theta3)*cos(theta4)*sin(theta2)*sin(theta3)*sin(theta4) - 11.28*thetad5*cos(theta2)*cos(theta3)*cos(theta4)*sin(theta2)*sin(theta3)*sin(theta4) - 1.6*thetad4*cos(theta1)*cos(theta2)*cos(theta3)*cos(theta4)^2*sin(theta2)*sin(theta3) - 1.6*thetad4*cos(theta1)*cos(theta2)*cos(theta3)^2*cos(theta4)*sin(theta2)*sin(theta4) - 0.8*thetad5*cos(theta1)*cos(theta2)*cos(theta3)*cos(theta4)^2*sin(theta2)*sin(theta3) - 1.6*thetad4*cos(theta1)*cos(theta2)^2*cos(theta3)*cos(theta4)*sin(theta3)*sin(theta4) - 0.8*thetad5*cos(theta1)*cos(theta2)*cos(theta3)^2*cos(theta4)*sin(theta2)*sin(theta4) - 0.8*thetad5*cos(theta1)*cos(theta2)^2*cos(theta3)*cos(theta4)*sin(theta3)*sin(theta4) - 11.2*thetad4*cos(theta2)*cos(theta3)*cos(theta4)^2*sin(theta1)*sin(theta2)*sin(theta3) - 11.2*thetad4*cos(theta2)*cos(theta3)^2*cos(theta4)*sin(theta1)*sin(theta2)*sin(theta4) - 5.6*thetad5*cos(theta2)*cos(theta3)*cos(theta4)^2*sin(theta1)*sin(theta2)*sin(theta3) - 11.2*thetad4*cos(theta2)^2*cos(theta3)*cos(theta4)*sin(theta1)*sin(theta3)*sin(theta4) - 5.6*thetad5*cos(theta2)*cos(theta3)^2*cos(theta4)*sin(theta1)*sin(theta2)*sin(theta4) - 5.6*thetad5*cos(theta2)^2*cos(theta3)*cos(theta4)*sin(theta1)*sin(theta3)*sin(theta4) - 7.04*thetad4*cos(theta1)*cos(theta2)*cos(theta3)^2*cos(theta4)^2*sin(theta1)*sin(theta2) - 7.04*thetad4*cos(theta1)*cos(theta2)^2*cos(theta3)*cos(theta4)^2*sin(theta1)*sin(theta3) - 3.52*thetad5*cos(theta1)*cos(theta2)*cos(theta3)^2*cos(theta4)^2*sin(theta1)*sin(theta2) - 7.04*thetad4*cos(theta1)*cos(theta2)^2*cos(theta3)^2*cos(theta4)*sin(theta1)*sin(theta4) - 3.52*thetad5*cos(theta1)*cos(theta2)^2*cos(theta3)*cos(theta4)^2*sin(theta1)*sin(theta3) - 3.52*thetad5*cos(theta1)*cos(theta2)^2*cos(theta3)^2*cos(theta4)*sin(theta1)*sin(theta4) + 25.12*thetad4*cos(theta1)^2*cos(theta2)*cos(theta3)*cos(theta4)*sin(theta2)*sin(theta3)*sin(theta4) + 12.56*thetad5*cos(theta1)^2*cos(theta2)*cos(theta3)*cos(theta4)*sin(theta2)*sin(theta3)*sin(theta4) + 7.04*thetad4*cos(theta1)*cos(theta2)*cos(theta3)*cos(theta4)*sin(theta1)*sin(theta2)*sin(theta3)*sin(theta4) + 3.52*thetad5*cos(theta1)*cos(theta2)*cos(theta3)*cos(theta4)*sin(theta1)*sin(theta2)*sin(theta3)*sin(theta4) ;
